simulink model "ODE_Hand_Model_v08_IPC_v03"  (Simulink 7.5)
settings: Solver=FixedStepDiscrete  StartTime=0.0  StopTime=inf  FixedStep=0.0315/(4*12)  RelTol=1e-3
values from neighbouring files (symbols this model uses):
  f_step = 0.7    [Set_Parameters.m]
  force_step = 20    [Set_Parameters.m]
  K_Conn = eye(4)*k_conn    [Set_Parameters.m]
  K_D = 30    [Set_Parameters.m]
  K_Or = eye(3)*k_Or    [Set_Parameters.m]
  K_Ot = eye(3)*k_Ot    [Set_Parameters.m]
  K_P = 350    [Set_Parameters.m]
  ksi = 0.9    [Set_Parameters.m]
  Kx = diag([diag(K_Ot)' diag(K_Or)' diag(K_Conn)'])    [Set_Parameters.m]
  l_des = [l1_des; l2_des; l3_des; l4_des]    [Set_Parameters.m]
  Mo = diag([sphere_mass*ones(1,3) (2/5)*sphere_mass*sphere_radius^2*ones(1,3)])    [Set_Parameters.m]
  qd_initial_touch = [0 0.3655   -0.5897   -0.5897     0       -0.3333   +0.5942   +0.5942         0       -0.298   --0.5226   --0.5226           0       -0.3333   +0.5942   +0.5942]    [Set_Parameters.m]
  R_O_Desired = R_O(x_i_v02(qd_initial_touch))    [Set_Parameters.m]
  t_f_start = 2.5    [Set_Parameters.m]
  torque_step = 60    [Set_Parameters.m]
  x_O_desired = (1/4)*sum(x_i_v02(qd_initial_touch))    [Set_Parameters.m]
undefined symbols (not defined in the file or in its folder): sigbuilder_block
libraries: dspmtrx3 x33, simulink x2, dspinverses x1
(part 2 of 6)

== matlab function Control/IPC/J/J_Or1/Embedded MATLAB Function1 ==
  data: xi input double size=[4 3]; J output double
%#eml
function J=J1(xi)

x1x=xi(1,1); x1y=xi(1,2); x1z=xi(1,3); 
x2x=xi(2,1); x2y=xi(2,2); x2z=xi(2,3);
x3x=xi(3,1); x3y=xi(3,2); x3z=xi(3,3);
x4x=xi(4,1); x4y=xi(4,2); x4z=xi(4,3);


J=[(x1x + (-1) .* x3x) .* (x1y + (-1) .* x3y) .* ((x1x + (-1) .*  ...
  x3x) .^ 2 + (x1y + (-1) .* x3y) .^ 2 + (x1z + (-1) .* x3z) .^ 2)  ...
  .^ (-3 / 2) .* (((-1) .* x1y + x3y) .* (x2x + (-1) .* x4x) + (x1x  ...
  + (-1) .* x3x) .* (x2y + (-1) .* x4y)) .* ((((-1) .* x1y + x3y) .* ...
   (x2x + (-1) .* x4x) + (x1x + (-1) .* x3x) .* (x2y + (-1) .* x4y)) ...
   .^ 2 + ((x1z + (-1) .* x3z) .* (x2x + (-1) .* x4x) + (-1) .* ( ...
  x1x + (-1) .* x3x) .* (x2z + (-1) .* x4z)) .^ 2 + (((-1) .* x1z +  ...
  x3z) .* (x2y + (-1) .* x4y) + (x1y + (-1) .* x3y) .* (x2z + (-1)  ...
  .* x4z)) .^ 2) .^ (-1 / 2) .* (((x1x + (-1) .* x3x) .* ((x1x + ( ...
  -1) .* x3x) .^ 2 + (x1y + (-1) .* x3y) .^ 2 + (x1z + (-1) .* x3z)  ...
  .^ 2) .^ (-1 / 2) + (x2x + (-1) .* x4x) .* ((x2x + (-1) .* x4x)  ...
  .^ 2 + (x2y + (-1) .* x4y) .^ 2 + (x2z + (-1) .* x4z) .^ 2) .^ ( ...
  -1 / 2)) .^ 2 + ((x1y + (-1) .* x3y) .* ((x1x + (-1) .* x3x) .^ 2  ...
  + (x1y + (-1) .* x3y) .^ 2 + (x1z + (-1) .* x3z) .^ 2) .^ (-1 / 2) ...
   + (x2y + (-1) .* x4y) .* ((x2x + (-1) .* x4x) .^ 2 + (x2y + (-1)  ...
  .* x4y) .^ 2 + (x2z + (-1) .* x4z) .^ 2) .^ (-1 / 2)) .^ 2 + ((( ...
  x1x + (-1) .* x3x) .^ 2 + (x1y + (-1) .* x3y) .^ 2 + (x1z + (-1)  ...
  .* x3z) .^ 2) .^ (-1 / 2) .* (x1z + (-1) .* x3z) + ((x2x + (-1) .* ...
   x4x) .^ 2 + (x2y + (-1) .* x4y) .^ 2 + (x2z + (-1) .* x4z) .^ 2)  ...
  .^ (-1 / 2) .* (x2z + (-1) .* x4z)) .^ 2) .^ (-1 / 2) + (1 / 2) .* ...
   (((-1) .* x1y + x3y) .* (x2x + (-1) .* x4x) + (x1x + (-1) .* x3x) ...
   .* (x2y + (-1) .* x4y)) .* ((((-1) .* x1y + x3y) .* (x2x + (-1)  ...
  .* x4x) + (x1x + (-1) .* x3x) .* (x2y + (-1) .* x4y)) .^ 2 + (( ...
  x1z + (-1) .* x3z) .* (x2x + (-1) .* x4x) + (-1) .* (x1x + (-1) .* ...
   x3x) .* (x2z + (-1) .* x4z)) .^ 2 + (((-1) .* x1z + x3z) .* (x2y  ...
  + (-1) .* x4y) + (x1y + (-1) .* x3y) .* (x2z + (-1) .* x4z)) .^ 2) ...
   .^ (-1 / 2) .* (2 .* ((-1) .* (x1x + (-1) .* x3x) .^ 2 .* ((x1x + ...
   (-1) .* x3x) .^ 2 + (x1y + (-1) .* x3y) .^ 2 + (x1z + (-1) .*  ...
  x3z) .^ 2) .^ (-3 / 2) + ((x1x + (-1) .* x3x) .^ 2 + (x1y + (-1)  ...
  .* x3y) .^ 2 + (x1z + (-1) .* x3z) .^ 2) .^ (-1 / 2)) .* ((x1x + ( ...
  -1) .* x3x) .* ((x1x + (-1) .* x3x) .^ 2 + (x1y + (-1) .* x3y) .^  ...
  2 + (x1z + (-1) .* x3z) .^ 2) .^ (-1 / 2) + (x2x + (-1) .* x4x) .* ...
   ((x2x + (-1) .* x4x) .^ 2 + (x2y + (-1) .* x4y) .^ 2 + (x2z + ( ...
  -1) .* x4z) .^ 2) .^ (-1 / 2)) + (-2) .* (x1x + (-1) .* x3x) .* ( ...
  x1y + (-1) .* x3y) .* ((x1x + (-1) .* x3x) .^ 2 + (x1y + (-1) .*  ...
  x3y) .^ 2 + (x1z + (-1) .* x3z) .^ 2) .^ (-3 / 2) .* ((x1y + (-1)  ...
  .* x3y) .* ((x1x + (-1) .* x3x) .^ 2 + (x1y + (-1) .* x3y) .^ 2 +  ...
  (x1z + (-1) .* x3z) .^ 2) .^ (-1 / 2) + (x2y + (-1) .* x4y) .* (( ...
  x2x + (-1) .* x4x) .^ 2 + (x2y + (-1) .* x4y) .^ 2 + (x2z + (-1)  ...
  .* x4z) .^ 2) .^ (-1 / 2)) + (-2) .* (x1x + (-1) .* x3x) .* ((x1x  ...
  + (-1) .* x3x) .^ 2 + (x1y + (-1) .* x3y) .^ 2 + (x1z + (-1) .*  ...
  x3z) .^ 2) .^ (-3 / 2) .* (x1z + (-1) .* x3z) .* (((x1x + (-1) .*  ...
  x3x) .^ 2 + (x1y + (-1) .* x3y) .^ 2 + (x1z + (-1) .* x3z) .^ 2)  ...
  .^ (-1 / 2) .* (x1z + (-1) .* x3z) + ((x2x + (-1) .* x4x) .^ 2 + ( ...
  x2y + (-1) .* x4y) .^ 2 + (x2z + (-1) .* x4z) .^ 2) .^ (-1 / 2) .* ...
   (x2z + (-1) .* x4z))) .* (((x1x + (-1) .* x3x) .* ((x1x + (-1) .* ...
   x3x) .^ 2 + (x1y + (-1) .* x3y) .^ 2 + (x1z + (-1) .* x3z) .^ 2)  ...
  .^ (-1 / 2) + (x2x + (-1) .* x4x) .* ((x2x + (-1) .* x4x) .^ 2 + ( ...
  x2y + (-1) .* x4y) .^ 2 + (x2z + (-1) .* x4z) .^ 2) .^ (-1 / 2))  ...
  .^ 2 + ((x1y + (-1) .* x3y) .* ((x1x + (-1) .* x3x) .^ 2 + (x1y +  ...
  (-1) .* x3y) .^ 2 + (x1z + (-1) .* x3z) .^ 2) .^ (-1 / 2) + (x2y + ...
   (-1) .* x4y) .* ((x2x + (-1) .* x4x) .^ 2 + (x2y + (-1) .* x4y)  ...
  .^ 2 + (x2z + (-1) .* x4z) .^ 2) .^ (-1 / 2)) .^ 2 + (((x1x + (-1) ...
   .* x3x) .^ 2 + (x1y + (-1) .* x3y) .^ 2 + (x1z + (-1) .* x3z) .^  ...
  2) .^ (-1 / 2) .* (x1z + (-1) .* x3z) + ((x2x + (-1) .* x4x) .^ 2  ...
  + (x2y + (-1) .* x4y) .^ 2 + (x2z + (-1) .* x4z) .^ 2) .^ (-1 / 2) ...
   .* (x2z + (-1) .* x4z)) .^ 2) .^ (-3 / 2) .* ((x1y + (-1) .* x3y) ...
   .* ((x1x + (-1) .* x3x) .^ 2 + (x1y + (-1) .* x3y) .^ 2 + (x1z +  ...
  (-1) .* x3z) .^ 2) .^ (-1 / 2) + (x2y + (-1) .* x4y) .* ((x2x + ( ...
  -1) .* x4x) .^ 2 + (x2y + (-1) .* x4y) .^ 2 + (x2z + (-1) .* x4z)  ...
  .^ 2) .^ (-1 / 2)) + (-1) .* (x2y + (-1) .* x4y) .* ((((-1) .*  ...
  x1y + x3y) .* (x2x + (-1) .* x4x) + (x1x + (-1) .* x3x) .* (x2y +  ...
  (-1) .* x4y)) .^ 2 + ((x1z + (-1) .* x3z) .* (x2x + (-1) .* x4x) + ...
   (-1) .* (x1x + (-1) .* x3x) .* (x2z + (-1) .* x4z)) .^ 2 + (((-1) ...
   .* x1z + x3z) .* (x2y + (-1) .* x4y) + (x1y + (-1) .* x3y) .* ( ...
  x2z + (-1) .* x4z)) .^ 2) .^ (-1 / 2) .* (((x1x + (-1) .* x3x) .*  ...
  ((x1x + (-1) .* x3x) .^ 2 + (x1y + (-1) .* x3y) .^ 2 + (x1z + (-1) ...
   .* x3z) .^ 2) .^ (-1 / 2) + (x2x + (-1) .* x4x) .* ((x2x + (-1)  ...
  .* x4x) .^ 2 + (x2y + (-1) .* x4y) .^ 2 + (x2z + (-1) .* x4z) .^  ...
  2) .^ (-1 / 2)) .^ 2 + ((x1y + (-1) .* x3y) .* ((x1x + (-1) .*  ...
  x3x) .^ 2 + (x1y + (-1) .* x3y) .^ 2 + (x1z + (-1) .* x3z) .^ 2)  ...
  .^ (-1 / 2) + (x2y + (-1) .* x4y) .* ((x2x + (-1) .* x4x) .^ 2 + ( ...
  x2y + (-1) .* x4y) .^ 2 + (x2z + (-1) .* x4z) .^ 2) .^ (-1 / 2))  ...
  .^ 2 + (((x1x + (-1) .* x3x) .^ 2 + (x1y + (-1) .* x3y) .^ 2 + ( ...
  x1z + (-1) .* x3z) .^ 2) .^ (-1 / 2) .* (x1z + (-1) .* x3z) + (( ...
  x2x + (-1) .* x4x) .^ 2 + (x2y + (-1) .* x4y) .^ 2 + (x2z + (-1)  ...
  .* x4z) .^ 2) .^ (-1 / 2) .* (x2z + (-1) .* x4z)) .^ 2) .^ (-1 /  ...
  2) .* ((x1y + (-1) .* x3y) .* ((x1x + (-1) .* x3x) .^ 2 + (x1y + ( ...
  -1) .* x3y) .^ 2 + (x1z + (-1) .* x3z) .^ 2) .^ (-1 / 2) + (x2y +  ...
  (-1) .* x4y) .* ((x2x + (-1) .* x4x) .^ 2 + (x2y + (-1) .* x4y)  ...
  .^ 2 + (x2z + (-1) .* x4z) .^ 2) .^ (-1 / 2)) + (-1) .* (x1x + ( ...
  -1) .* x3x) .* ((x1x + (-1) .* x3x) .^ 2 + (x1y + (-1) .* x3y) .^  ...
  2 + (x1z + (-1) .* x3z) .^ 2) .^ (-3 / 2) .* (x1z + (-1) .* x3z)  ...
  .* ((((-1) .* x1y + x3y) .* (x2x + (-1) .* x4x) + (x1x + (-1) .*  ...
  x3x) .* (x2y + (-1) .* x4y)) .^ 2 + ((x1z + (-1) .* x3z) .* (x2x + ...
   (-1) .* x4x) + (-1) .* (x1x + (-1) .* x3x) .* (x2z + (-1) .* x4z) ...
  ) .^ 2 + (((-1) .* x1z + x3z) .* (x2y + (-1) .* x4y) + (x1y + (-1) ...
   .* x3y) .* (x2z + (-1) .* x4z)) .^ 2) .^ (-1 / 2) .* (((x1x + ( ...
  -1) .* x3x) .* ((x1x + (-1) .* x3x) .^ 2 + (x1y + (-1) .* x3y) .^  ...
  2 + (x1z + (-1) .* x3z) .^ 2) .^ (-1 / 2) + (x2x + (-1) .* x4x) .* ...
   ((x2x + (-1) .* x4x) .^ 2 + (x2y + (-1) .* x4y) .^ 2 + (x2z + ( ...
  -1) .* x4z) .^ 2) .^ (-1 / 2)) .^ 2 + ((x1y + (-1) .* x3y) .* (( ...
  x1x + (-1) .* x3x) .^ 2 + (x1y + (-1) .* x3y) .^ 2 + (x1z + (-1)  ...
  .* x3z) .^ 2) .^ (-1 / 2) + (x2y + (-1) .* x4y) .* ((x2x + (-1) .* ...
   x4x) .^ 2 + (x2y + (-1) .* x4y) .^ 2 + (x2z + (-1) .* x4z) .^ 2)  ...
  .^ (-1 / 2)) .^ 2 + (((x1x + (-1) .* x3x) .^ 2 + (x1y + (-1) .*  ...
  x3y) .^ 2 + (x1z + (-1) .* x3z) .^ 2) .^ (-1 / 2) .* (x1z + (-1)  ...
  .* x3z) + ((x2x + (-1) .* x4x) .^ 2 + (x2y + (-1) .* x4y) .^ 2 + ( ...
  x2z + (-1) .* x4z) .^ 2) .^ (-1 / 2) .* (x2z + (-1) .* x4z)) .^ 2) ...
   .^ (-1 / 2) .* ((x1z + (-1) .* x3z) .* (x2x + (-1) .* x4x) + (-1) ...
   .* (x1x + (-1) .* x3x) .* (x2z + (-1) .* x4z)) + (-1 / 2) .* (((( ...
  -1) .* x1y + x3y) .* (x2x + (-1) .* x4x) + (x1x + (-1) .* x3x) .*  ...
  (x2y + (-1) .* x4y)) .^ 2 + ((x1z + (-1) .* x3z) .* (x2x + (-1) .* ...
   x4x) + (-1) .* (x1x + (-1) .* x3x) .* (x2z + (-1) .* x4z)) .^ 2 + ...
   (((-1) .* x1z + x3z) .* (x2y + (-1) .* x4y) + (x1y + (-1) .* x3y) ...
   .* (x2z + (-1) .* x4z)) .^ 2) .^ (-1 / 2) .* (2 .* ((-1) .* (x1x  ...
  + (-1) .* x3x) .^ 2 .* ((x1x + (-1) .* x3x) .^ 2 + (x1y + (-1) .*  ...
  x3y) .^ 2 + (x1z + (-1) .* x3z) .^ 2) .^ (-3 / 2) + ((x1x + (-1)  ...
  .* x3x) .^ 2 + (x1y + (-1) .* x3y) .^ 2 + (x1z + (-1) .* x3z) .^  ...
  2) .^ (-1 / 2)) .* ((x1x + (-1) .* x3x) .* ((x1x + (-1) .* x3x)  ...
  .^ 2 + (x1y + (-1) .* x3y) .^ 2 + (x1z + (-1) .* x3z) .^ 2) .^ ( ...
  -1 / 2) + (x2x + (-1) .* x4x) .* ((x2x + (-1) .* x4x) .^ 2 + (x2y  ...
  + (-1) .* x4y) .^ 2 + (x2z + (-1) .* x4z) .^ 2) .^ (-1 / 2)) + ( ...
  -2) .* (x1x + (-1) .* x3x) .* (x1y + (-1) .* x3y) .* ((x1x + (-1)  ...
  .* x3x) .^ 2 + (x1y + (-1) .* x3y) .^ 2 + (x1z + (-1) .* x3z) .^  ...
  2) .^ (-3 / 2) .* ((x1y + (-1) .* x3y) .* ((x1x + (-1) .* x3x) .^  ...
  2 + (x1y + (-1) .* x3y) .^ 2 + (x1z + (-1) .* x3z) .^ 2) .^ (-1 /  ...
  2) + (x2y + (-1) .* x4y) .* ((x2x + (-1) .* x4x) .^ 2 + (x2y + ( ...
  -1) .* x4y) .^ 2 + (x2z + (-1) .* x4z) .^ 2) .^ (-1 / 2)) + (-2)  ...
  .* (x1x + (-1) .* x3x) .* ((x1x + (-1) .* x3x) .^ 2 + (x1y + (-1)  ...
  .* x3y) .^ 2 + (x1z + (-1) .* x3z) .^ 2) .^ (-3 / 2) .* (x1z + ( ...
  -1) .* x3z) .* (((x1x + (-1) .* x3x) .^ 2 + (x1y + (-1) .* x3y)  ...
  .^ 2 + (x1z + (-1) .* x3z) .^ 2) .^ (-1 / 2) .* (x1z + (-1) .*  ...
  x3z) + ((x2x + (-1) .* x4x) .^ 2 + (x2y + (-1) .* x4y) .^ 2 + ( ...
  x2z + (-1) .* x4z) .^ 2) .^ (-1 / 2) .* (x2z + (-1) .* x4z))) .* ( ...
  ((x1x + (-1) .* x3x) .* ((x1x + (-1) .* x3x) .^ 2 + (x1y + (-1) .* ...
   x3y) .^ 2 + (x1z + (-1) .* x3z) .^ 2) .^ (-1 / 2) + (x2x + (-1)  ...
  .* x4x) .* ((x2x + (-1) .* x4x) .^ 2 + (x2y + (-1) .* x4y) .^ 2 +  ...
  (x2z + (-1) .* x4z) .^ 2) .^ (-1 / 2)) .^ 2 + ((x1y + (-1) .* x3y) ...
   .* ((x1x + (-1) .* x3x) .^ 2 + (x1y + (-1) .* x3y) .^ 2 + (x1z +  ...
  (-1) .* x3z) .^ 2) .^ (-1 / 2) + (x2y + (-1) .* x4y) .* ((x2x + ( ...
  -1) .* x4x) .^ 2 + (x2y + (-1) .* x4y) .^ 2 + (x2z + (-1) .* x4z)  ...
  .^ 2) .^ (-1 / 2)) .^ 2 + (((x1x + (-1) .* x3x) .^ 2 + (x1y + (-1) ...
   .* x3y) .^ 2 + (x1z + (-1) .* x3z) .^ 2) .^ (-1 / 2) .* (x1z + ( ...
  -1) .* x3z) + ((x2x + (-1) .* x4x) .^ 2 + (x2y + (-1) .* x4y) .^  ...
  2 + (x2z + (-1) .* x4z) .^ 2) .^ (-1 / 2) .* (x2z + (-1) .* x4z))  ...
  .^ 2) .^ (-3 / 2) .* ((x1z + (-1) .* x3z) .* (x2x + (-1) .* x4x) + ...
   (-1) .* (x1x + (-1) .* x3x) .* (x2z + (-1) .* x4z)) .* (((x1x + ( ...
  -1) .* x3x) .^ 2 + (x1y + (-1) .* x3y) .^ 2 + (x1z + (-1) .* x3z)  ...
  .^ 2) .^ (-1 / 2) .* (x1z + (-1) .* x3z) + ((x2x + (-1) .* x4x)  ...
  .^ 2 + (x2y + (-1) .* x4y) .^ 2 + (x2z + (-1) .* x4z) .^ 2) .^ ( ...
  -1 / 2) .* (x2z + (-1) .* x4z)) + ((((-1) .* x1y + x3y) .* (x2x +  ...
  (-1) .* x4x) + (x1x + (-1) .* x3x) .* (x2y + (-1) .* x4y)) .^ 2 +  ...
  ((x1z + (-1) .* x3z) .* (x2x + (-1) .* x4x) + (-1) .* (x1x + (-1)  ...
  .* x3x) .* (x2z + (-1) .* x4z)) .^ 2 + (((-1) .* x1z + x3z) .* ( ...
  x2y + (-1) .* x4y) + (x1y + (-1) .* x3y) .* (x2z + (-1) .* x4z))  ...
  .^ 2) .^ (-1 / 2) .* (((x1x + (-1) .* x3x) .* ((x1x + (-1) .* x3x) ...
   .^ 2 + (x1y + (-1) .* x3y) .^ 2 + (x1z + (-1) .* x3z) .^ 2) .^ ( ...
  -1 / 2) + (x2x + (-1) .* x4x) .* ((x2x + (-1) .* x4x) .^ 2 + (x2y  ...
  + (-1) .* x4y) .^ 2 + (x2z + (-1) .* x4z) .^ 2) .^ (-1 / 2)) .^ 2  ...
  + ((x1y + (-1) .* x3y) .* ((x1x + (-1) .* x3x) .^ 2 + (x1y + (-1)  ...
  .* x3y) .^ 2 + (x1z + (-1) .* x3z) .^ 2) .^ (-1 / 2) + (x2y + (-1) ...
   .* x4y) .* ((x2x + (-1) .* x4x) .^ 2 + (x2y + (-1) .* x4y) .^ 2 + ...
   (x2z + (-1) .* x4z) .^ 2) .^ (-1 / 2)) .^ 2 + (((x1x + (-1) .*  ...
  x3x) .^ 2 + (x1y + (-1) .* x3y) .^ 2 + (x1z + (-1) .* x3z) .^ 2)  ...
  .^ (-1 / 2) .* (x1z + (-1) .* x3z) + ((x2x + (-1) .* x4x) .^ 2 + ( ...
  x2y + (-1) .* x4y) .^ 2 + (x2z + (-1) .* x4z) .^ 2) .^ (-1 / 2) .* ...
   (x2z + (-1) .* x4z)) .^ 2) .^ (-1 / 2) .* (((x1x + (-1) .* x3x)  ...
  .^ 2 + (x1y + (-1) .* x3y) .^ 2 + (x1z + (-1) .* x3z) .^ 2) .^ ( ...
  -1 / 2) .* (x1z + (-1) .* x3z) + ((x2x + (-1) .* x4x) .^ 2 + (x2y  ...
  + (-1) .* x4y) .^ 2 + (x2z + (-1) .* x4z) .^ 2) .^ (-1 / 2) .* ( ...
  x2z + (-1) .* x4z)) .* ((-1) .* x2z + x4z) + (1 / 2) .* (((-1) .*  ...
  x1y + x3y) .* (x2x + (-1) .* x4x) + (x1x + (-1) .* x3x) .* (x2y +  ...
  (-1) .* x4y)) .* ((((-1) .* x1y + x3y) .* (x2x + (-1) .* x4x) + ( ...
  x1x + (-1) .* x3x) .* (x2y + (-1) .* x4y)) .^ 2 + ((x1z + (-1) .*  ...
  x3z) .* (x2x + (-1) .* x4x) + (-1) .* (x1x + (-1) .* x3x) .* (x2z  ...
  + (-1) .* x4z)) .^ 2 + (((-1) .* x1z + x3z) .* (x2y + (-1) .* x4y) ...
   + (x1y + (-1) .* x3y) .* (x2z + (-1) .* x4z)) .^ 2) .^ (-3 / 2)  ...
  .* (((x1x + (-1) .* x3x) .* ((x1x + (-1) .* x3x) .^ 2 + (x1y + ( ...
  -1) .* x3y) .^ 2 + (x1z + (-1) .* x3z) .^ 2) .^ (-1 / 2) + (x2x +  ...
  (-1) .* x4x) .* ((x2x + (-1) .* x4x) .^ 2 + (x2y + (-1) .* x4y)  ...
  .^ 2 + (x2z + (-1) .* x4z) .^ 2) .^ (-1 / 2)) .^ 2 + ((x1y + (-1)  ...
  .* x3y) .* ((x1x + (-1) .* x3x) .^ 2 + (x1y + (-1) .* x3y) .^ 2 +  ...
  (x1z + (-1) .* x3z) .^ 2) .^ (-1 / 2) + (x2y + (-1) .* x4y) .* (( ...
  x2x + (-1) .* x4x) .^ 2 + (x2y + (-1) .* x4y) .^ 2 + (x2z + (-1)  ...
  .* x4z) .^ 2) .^ (-1 / 2)) .^ 2 + (((x1x + (-1) .* x3x) .^ 2 + ( ...
  x1y + (-1) .* x3y) .^ 2 + (x1z + (-1) .* x3z) .^ 2) .^ (-1 / 2) .* ...
   (x1z + (-1) .* x3z) + ((x2x + (-1) .* x4x) .^ 2 + (x2y + (-1) .*  ...
  x4y) .^ 2 + (x2z + (-1) .* x4z) .^ 2) .^ (-1 / 2) .* (x2z + (-1)  ...
  .* x4z)) .^ 2) .^ (-1 / 2) .* ((x1y + (-1) .* x3y) .* ((x1x + (-1) ...
   .* x3x) .^ 2 + (x1y + (-1) .* x3y) .^ 2 + (x1z + (-1) .* x3z) .^  ...
  2) .^ (-1 / 2) + (x2y + (-1) .* x4y) .* ((x2x + (-1) .* x4x) .^ 2  ...
  + (x2y + (-1) .* x4y) .^ 2 + (x2z + (-1) .* x4z) .^ 2) .^ (-1 / 2) ...
  ) .* (2 .* (((-1) .* x1y + x3y) .* (x2x + (-1) .* x4x) + (x1x + ( ...
  -1) .* x3x) .* (x2y + (-1) .* x4y)) .* (x2y + (-1) .* x4y) + 2 .*  ...
  ((x1z + (-1) .* x3z) .* (x2x + (-1) .* x4x) + (-1) .* (x1x + (-1)  ...
  .* x3x) .* (x2z + (-1) .* x4z)) .* ((-1) .* x2z + x4z)) + (-1 / 2) ...
   .* ((((-1) .* x1y + x3y) .* (x2x + (-1) .* x4x) + (x1x + (-1) .*  ...
  x3x) .* (x2y + (-1) .* x4y)) .^ 2 + ((x1z + (-1) .* x3z) .* (x2x + ...
   (-1) .* x4x) + (-1) .* (x1x + (-1) .* x3x) .* (x2z + (-1) .* x4z) ...
  ) .^ 2 + (((-1) .* x1z + x3z) .* (x2y + (-1) .* x4y) + (x1y + (-1) ...
   .* x3y) .* (x2z + (-1) .* x4z)) .^ 2) .^ (-3 / 2) .* (((x1x + ( ...
  -1) .* x3x) .* ((x1x + (-1) .* x3x) .^ 2 + (x1y + (-1) .* x3y) .^  ...
  2 + (x1z + (-1) .* x3z) .^ 2) .^ (-1 / 2) + (x2x + (-1) .* x4x) .* ...
   ((x2x + (-1) .* x4x) .^ 2 + (x2y + (-1) .* x4y) .^ 2 + (x2z + ( ...
  -1) .* x4z) .^ 2) .^ (-1 / 2)) .^ 2 + ((x1y + (-1) .* x3y) .* (( ...
  x1x + (-1) .* x3x) .^ 2 + (x1y + (-1) .* x3y) .^ 2 + (x1z + (-1)  ...
  .* x3z) .^ 2) .^ (-1 / 2) + (x2y + (-1) .* x4y) .* ((x2x + (-1) .* ...
   x4x) .^ 2 + (x2y + (-1) .* x4y) .^ 2 + (x2z + (-1) .* x4z) .^ 2)  ...
  .^ (-1 / 2)) .^ 2 + (((x1x + (-1) .* x3x) .^ 2 + (x1y + (-1) .*  ...
  x3y) .^ 2 + (x1z + (-1) .* x3z) .^ 2) .^ (-1 / 2) .* (x1z + (-1)  ...
  .* x3z) + ((x2x + (-1) .* x4x) .^ 2 + (x2y + (-1) .* x4y) .^ 2 + ( ...
  x2z + (-1) .* x4z) .^ 2) .^ (-1 / 2) .* (x2z + (-1) .* x4z)) .^ 2) ...
   .^ (-1 / 2) .* ((x1z + (-1) .* x3z) .* (x2x + (-1) .* x4x) + (-1) ...
   .* (x1x + (-1) .* x3x) .* (x2z + (-1) .* x4z)) .* (((x1x + (-1)  ...
  .* x3x) .^ 2 + (x1y + (-1) .* x3y) .^ 2 + (x1z + (-1) .* x3z) .^  ...
  2) .^ (-1 / 2) .* (x1z + (-1) .* x3z) + ((x2x + (-1) .* x4x) .^ 2  ...
  + (x2y + (-1) .* x4y) .^ 2 + (x2z + (-1) .* x4z) .^ 2) .^ (-1 / 2) ...
   .* (x2z + (-1) .* x4z)) .* (2 .* (((-1) .* x1y + x3y) .* (x2x + ( ...
  -1) .* x4x) + (x1x + (-1) .* x3x) .* (x2y + (-1) .* x4y)) .* (x2y  ...
  + (-1) .* x4y) + 2 .* ((x1z + (-1) .* x3z) .* (x2x + (-1) .* x4x)  ...
  + (-1) .* (x1x + (-1) .* x3x) .* (x2z + (-1) .* x4z)) .* ((-1) .*  ...
  x2z + x4z)),(-1) .* ((-1) .* (x1y + (-1) .* x3y) .^ 2 .* ((x1x + ( ...
  -1) .* x3x) .^ 2 + (x1y + (-1) .* x3y) .^ 2 + (x1z + (-1) .* x3z)  ...
  .^ 2) .^ (-3 / 2) + ((x1x + (-1) .* x3x) .^ 2 + (x1y + (-1) .*  ...
  x3y) .^ 2 + (x1z + (-1) .* x3z) .^ 2) .^ (-1 / 2)) .* (((-1) .*  ...
  x1y + x3y) .* (x2x + (-1) .* x4x) + (x1x + (-1) .* x3x) .* (x2y +  ...
  (-1) .* x4y)) .* ((((-1) .* x1y + x3y) .* (x2x + (-1) .* x4x) + ( ...
  x1x + (-1) .* x3x) .* (x2y + (-1) .* x4y)) .^ 2 + ((x1z + (-1) .*  ...
  x3z) .* (x2x + (-1) .* x4x) + (-1) .* (x1x + (-1) .* x3x) .* (x2z  ...
  + (-1) .* x4z)) .^ 2 + (((-1) .* x1z + x3z) .* (x2y + (-1) .* x4y) ...
   + (x1y + (-1) .* x3y) .* (x2z + (-1) .* x4z)) .^ 2) .^ (-1 / 2)  ...
  .* (((x1x + (-1) .* x3x) .* ((x1x + (-1) .* x3x) .^ 2 + (x1y + ( ...
  -1) .* x3y) .^ 2 + (x1z + (-1) .* x3z) .^ 2) .^ (-1 / 2) + (x2x +  ...
  (-1) .* x4x) .* ((x2x + (-1) .* x4x) .^ 2 + (x2y + (-1) .* x4y)  ...
  .^ 2 + (x2z + (-1) .* x4z) .^ 2) .^ (-1 / 2)) .^ 2 + ((x1y + (-1)  ...
  .* x3y) .* ((x1x + (-1) .* x3x) .^ 2 + (x1y + (-1) .* x3y) .^ 2 +  ...
  (x1z + (-1) .* x3z) .^ 2) .^ (-1 / 2) + (x2y + (-1) .* x4y) .* (( ...
  x2x + (-1) .* x4x) .^ 2 + (x2y + (-1) .* x4y) .^ 2 + (x2z + (-1)  ...
  .* x4z) .^ 2) .^ (-1 / 2)) .^ 2 + (((x1x + (-1) .* x3x) .^ 2 + ( ...
  x1y + (-1) .* x3y) .^ 2 + (x1z + (-1) .* x3z) .^ 2) .^ (-1 / 2) .* ...
   (x1z + (-1) .* x3z) + ((x2x + (-1) .* x4x) .^ 2 + (x2y + (-1) .*  ...
  x4y) .^ 2 + (x2z + (-1) .* x4z) .^ 2) .^ (-1 / 2) .* (x2z + (-1)  ...
  .* x4z)) .^ 2) .^ (-1 / 2) + (1 / 2) .* (((-1) .* x1y + x3y) .* ( ...
  x2x + (-1) .* x4x) + (x1x + (-1) .* x3x) .* (x2y + (-1) .* x4y))  ...
  .* ((((-1) .* x1y + x3y) .* (x2x + (-1) .* x4x) + (x1x + (-1) .*  ...
  x3x) .* (x2y + (-1) .* x4y)) .^ 2 + ((x1z + (-1) .* x3z) .* (x2x + ...
   (-1) .* x4x) + (-1) .* (x1x + (-1) .* x3x) .* (x2z + (-1) .* x4z) ...
  ) .^ 2 + (((-1) .* x1z + x3z) .* (x2y + (-1) .* x4y) + (x1y + (-1) ...
   .* x3y) .* (x2z + (-1) .* x4z)) .^ 2) .^ (-1 / 2) .* ((-2) .* ( ...
  x1x + (-1) .* x3x) .* (x1y + (-1) .* x3y) .* ((x1x + (-1) .* x3x)  ...
  .^ 2 + (x1y + (-1) .* x3y) .^ 2 + (x1z + (-1) .* x3z) .^ 2) .^ ( ...
  -3 / 2) .* ((x1x + (-1) .* x3x) .* ((x1x + (-1) .* x3x) .^ 2 + ( ...
  x1y + (-1) .* x3y) .^ 2 + (x1z + (-1) .* x3z) .^ 2) .^ (-1 / 2) +  ...
  (x2x + (-1) .* x4x) .* ((x2x + (-1) .* x4x) .^ 2 + (x2y + (-1) .*  ...
  x4y) .^ 2 + (x2z + (-1) .* x4z) .^ 2) .^ (-1 / 2)) + 2 .* ((-1) .* ...
   (x1y + (-1) .* x3y) .^ 2 .* ((x1x + (-1) .* x3x) .^ 2 + (x1y + ( ...
  -1) .* x3y) .^ 2 + (x1z + (-1) .* x3z) .^ 2) .^ (-3 / 2) + ((x1x + ...
   (-1) .* x3x) .^ 2 + (x1y + (-1) .* x3y) .^ 2 + (x1z + (-1) .*  ...
  x3z) .^ 2) .^ (-1 / 2)) .* ((x1y + (-1) .* x3y) .* ((x1x + (-1) .* ...
   x3x) .^ 2 + (x1y + (-1) .* x3y) .^ 2 + (x1z + (-1) .* x3z) .^ 2)  ...
  .^ (-1 / 2) + (x2y + (-1) .* x4y) .* ((x2x + (-1) .* x4x) .^ 2 + ( ...
  x2y + (-1) .* x4y) .^ 2 + (x2z + (-1) .* x4z) .^ 2) .^ (-1 / 2)) + ...
   (-2) .* (x1y + (-1) .* x3y) .* ((x1x + (-1) .* x3x) .^ 2 + (x1y + ...
   (-1) .* x3y) .^ 2 + (x1z + (-1) .* x3z) .^ 2) .^ (-3 / 2) .* ( ...
  x1z + (-1) .* x3z) .* (((x1x + (-1) .* x3x) .^ 2 + (x1y + (-1) .*  ...
  x3y) .^ 2 + (x1z + (-1) .* x3z) .^ 2) .^ (-1 / 2) .* (x1z + (-1)  ...
  .* x3z) + ((x2x + (-1) .* x4x) .^ 2 + (x2y + (-1) .* x4y) .^ 2 + ( ...
  x2z + (-1) .* x4z) .^ 2) .^ (-1 / 2) .* (x2z + (-1) .* x4z))) .* ( ...
  ((x1x + (-1) .* x3x) .* ((x1x + (-1) .* x3x) .^ 2 + (x1y + (-1) .* ...
   x3y) .^ 2 + (x1z + (-1) .* x3z) .^ 2) .^ (-1 / 2) + (x2x + (-1)  ...
  .* x4x) .* ((x2x + (-1) .* x4x) .^ 2 + (x2y + (-1) .* x4y) .^ 2 +  ...
  (x2z + (-1) .* x4z) .^ 2) .^ (-1 / 2)) .^ 2 + ((x1y + (-1) .* x3y) ...
   .* ((x1x + (-1) .* x3x) .^ 2 + (x1y + (-1) .* x3y) .^ 2 + (x1z +  ...
  (-1) .* x3z) .^ 2) .^ (-1 / 2) + (x2y + (-1) .* x4y) .* ((x2x + ( ...
  -1) .* x4x) .^ 2 + (x2y + (-1) .* x4y) .^ 2 + (x2z + (-1) .* x4z)  ...
  .^ 2) .^ (-1 / 2)) .^ 2 + (((x1x + (-1) .* x3x) .^ 2 + (x1y + (-1) ...
   .* x3y) .^ 2 + (x1z + (-1) .* x3z) .^ 2) .^ (-1 / 2) .* (x1z + ( ...
  -1) .* x3z) + ((x2x + (-1) .* x4x) .^ 2 + (x2y + (-1) .* x4y) .^  ...
  2 + (x2z + (-1) .* x4z) .^ 2) .^ (-1 / 2) .* (x2z + (-1) .* x4z))  ...
  .^ 2) .^ (-3 / 2) .* ((x1y + (-1) .* x3y) .* ((x1x + (-1) .* x3x)  ...
  .^ 2 + (x1y + (-1) .* x3y) .^ 2 + (x1z + (-1) .* x3z) .^ 2) .^ ( ...
  -1 / 2) + (x2y + (-1) .* x4y) .* ((x2x + (-1) .* x4x) .^ 2 + (x2y  ...
  + (-1) .* x4y) .^ 2 + (x2z + (-1) .* x4z) .^ 2) .^ (-1 / 2)) + ( ...
  -1) .* ((-1) .* x2x + x4x) .* ((((-1) .* x1y + x3y) .* (x2x + (-1) ...
   .* x4x) + (x1x + (-1) .* x3x) .* (x2y + (-1) .* x4y)) .^ 2 + (( ...
  x1z + (-1) .* x3z) .* (x2x + (-1) .* x4x) + (-1) .* (x1x + (-1) .* ...
   x3x) .* (x2z + (-1) .* x4z)) .^ 2 + (((-1) .* x1z + x3z) .* (x2y  ...
  + (-1) .* x4y) + (x1y + (-1) .* x3y) .* (x2z + (-1) .* x4z)) .^ 2) ...
   .^ (-1 / 2) .* (((x1x + (-1) .* x3x) .* ((x1x + (-1) .* x3x) .^  ...
  2 + (x1y + (-1) .* x3y) .^ 2 + (x1z + (-1) .* x3z) .^ 2) .^ (-1 /  ...
  2) + (x2x + (-1) .* x4x) .* ((x2x + (-1) .* x4x) .^ 2 + (x2y + ( ...
  -1) .* x4y) .^ 2 + (x2z + (-1) .* x4z) .^ 2) .^ (-1 / 2)) .^ 2 + ( ...
  (x1y + (-1) .* x3y) .* ((x1x + (-1) .* x3x) .^ 2 + (x1y + (-1) .*  ...
  x3y) .^ 2 + (x1z + (-1) .* x3z) .^ 2) .^ (-1 / 2) + (x2y + (-1) .* ...
   x4y) .* ((x2x + (-1) .* x4x) .^ 2 + (x2y + (-1) .* x4y) .^ 2 + ( ...
  x2z + (-1) .* x4z) .^ 2) .^ (-1 / 2)) .^ 2 + (((x1x + (-1) .* x3x) ...
   .^ 2 + (x1y + (-1) .* x3y) .^ 2 + (x1z + (-1) .* x3z) .^ 2) .^ ( ...
  -1 / 2) .* (x1z + (-1) .* x3z) + ((x2x + (-1) .* x4x) .^ 2 + (x2y  ...
  + (-1) .* x4y) .^ 2 + (x2z + (-1) .* x4z) .^ 2) .^ (-1 / 2) .* ( ...
  x2z + (-1) .* x4z)) .^ 2) .^ (-1 / 2) .* ((x1y + (-1) .* x3y) .* ( ...
  (x1x + (-1) .* x3x) .^ 2 + (x1y + (-1) .* x3y) .^ 2 + (x1z + (-1)  ...
  .* x3z) .^ 2) .^ (-1 / 2) + (x2y + (-1) .* x4y) .* ((x2x + (-1) .* ...
   x4x) .^ 2 + (x2y + (-1) .* x4y) .^ 2 + (x2z + (-1) .* x4z) .^ 2)  ...
  .^ (-1 / 2)) + (-1) .* (x1y + (-1) .* x3y) .* ((x1x + (-1) .* x3x) ...
   .^ 2 + (x1y + (-1) .* x3y) .^ 2 + (x1z + (-1) .* x3z) .^ 2) .^ ( ...
  -3 / 2) .* (x1z + (-1) .* x3z) .* ((((-1) .* x1y + x3y) .* (x2x +  ...
  (-1) .* x4x) + (x1x + (-1) .* x3x) .* (x2y + (-1) .* x4y)) .^ 2 +  ...
  ((x1z + (-1) .* x3z) .* (x2x + (-1) .* x4x) + (-1) .* (x1x + (-1)  ...
  .* x3x) .* (x2z + (-1) .* x4z)) .^ 2 + (((-1) .* x1z + x3z) .* ( ...
  x2y + (-1) .* x4y) + (x1y + (-1) .* x3y) .* (x2z + (-1) .* x4z))  ...
  .^ 2) .^ (-1 / 2) .* (((x1x + (-1) .* x3x) .* ((x1x + (-1) .* x3x) ...
   .^ 2 + (x1y + (-1) .* x3y) .^ 2 + (x1z + (-1) .* x3z) .^ 2) .^ ( ...
  -1 / 2) + (x2x + (-1) .* x4x) .* ((x2x + (-1) .* x4x) .^ 2 + (x2y  ...
  + (-1) .* x4y) .^ 2 + (x2z + (-1) .* x4z) .^ 2) .^ (-1 / 2)) .^ 2  ...
  + ((x1y + (-1) .* x3y) .* ((x1x + (-1) .* x3x) .^ 2 + (x1y + (-1)  ...
  .* x3y) .^ 2 + (x1z + (-1) .* x3z) .^ 2) .^ (-1 / 2) + (x2y + (-1) ...
   .* x4y) .* ((x2x + (-1) .* x4x) .^ 2 + (x2y + (-1) .* x4y) .^ 2 + ...
   (x2z + (-1) .* x4z) .^ 2) .^ (-1 / 2)) .^ 2 + (((x1x + (-1) .*  ...
  x3x) .^ 2 + (x1y + (-1) .* x3y) .^ 2 + (x1z + (-1) .* x3z) .^ 2)  ...
  .^ (-1 / 2) .* (x1z + (-1) .* x3z) + ((x2x + (-1) .* x4x) .^ 2 + ( ...
  x2y + (-1) .* x4y) .^ 2 + (x2z + (-1) .* x4z) .^ 2) .^ (-1 / 2) .* ...
   (x2z + (-1) .* x4z)) .^ 2) .^ (-1 / 2) .* ((x1z + (-1) .* x3z) .* ...
   (x2x + (-1) .* x4x) + (-1) .* (x1x + (-1) .* x3x) .* (x2z + (-1)  ...
  .* x4z)) + (1 / 2) .* (((-1) .* x1y + x3y) .* (x2x + (-1) .* x4x)  ...
  + (x1x + (-1) .* x3x) .* (x2y + (-1) .* x4y)) .* ((((-1) .* x1y +  ...
  x3y) .* (x2x + (-1) .* x4x) + (x1x + (-1) .* x3x) .* (x2y + (-1)  ...
  .* x4y)) .^ 2 + ((x1z + (-1) .* x3z) .* (x2x + (-1) .* x4x) + (-1) ...
   .* (x1x + (-1) .* x3x) .* (x2z + (-1) .* x4z)) .^ 2 + (((-1) .*  ...
  x1z + x3z) .* (x2y + (-1) .* x4y) + (x1y + (-1) .* x3y) .* (x2z +  ...
  (-1) .* x4z)) .^ 2) .^ (-3 / 2) .* (((x1x + (-1) .* x3x) .* ((x1x  ...
  + (-1) .* x3x) .^ 2 + (x1y + (-1) .* x3y) .^ 2 + (x1z + (-1) .*  ...
  x3z) .^ 2) .^ (-1 / 2) + (x2x + (-1) .* x4x) .* ((x2x + (-1) .*  ...
  x4x) .^ 2 + (x2y + (-1) .* x4y) .^ 2 + (x2z + (-1) .* x4z) .^ 2)  ...
  .^ (-1 / 2)) .^ 2 + ((x1y + (-1) .* x3y) .* ((x1x + (-1) .* x3x)  ...
  .^ 2 + (x1y + (-1) .* x3y) .^ 2 + (x1z + (-1) .* x3z) .^ 2) .^ ( ...
  -1 / 2) + (x2y + (-1) .* x4y) .* ((x2x + (-1) .* x4x) .^ 2 + (x2y  ...
  + (-1) .* x4y) .^ 2 + (x2z + (-1) .* x4z) .^ 2) .^ (-1 / 2)) .^ 2  ...
  + (((x1x + (-1) .* x3x) .^ 2 + (x1y + (-1) .* x3y) .^ 2 + (x1z + ( ...
  -1) .* x3z) .^ 2) .^ (-1 / 2) .* (x1z + (-1) .* x3z) + ((x2x + ( ...
  -1) .* x4x) .^ 2 + (x2y + (-1) .* x4y) .^ 2 + (x2z + (-1) .* x4z)  ...
  .^ 2) .^ (-1 / 2) .* (x2z + (-1) .* x4z)) .^ 2) .^ (-1 / 2) .* (( ...
  x1y + (-1) .* x3y) .* ((x1x + (-1) .* x3x) .^ 2 + (x1y + (-1) .*  ...
  x3y) .^ 2 + (x1z + (-1) .* x3z) .^ 2) .^ (-1 / 2) + (x2y + (-1) .* ...
   x4y) .* ((x2x + (-1) .* x4x) .^ 2 + (x2y + (-1) .* x4y) .^ 2 + ( ...
  x2z + (-1) .* x4z) .^ 2) .^ (-1 / 2)) .* (2 .* ((-1) .* x2x + x4x) ...
   .* (((-1) .* x1y + x3y) .* (x2x + (-1) .* x4x) + (x1x + (-1) .*  ...
  x3x) .* (x2y + (-1) .* x4y)) + 2 .* (((-1) .* x1z + x3z) .* (x2y + ...
   (-1) .* x4y) + (x1y + (-1) .* x3y) .* (x2z + (-1) .* x4z)) .* ( ...
  x2z + (-1) .* x4z)) + (-1 / 2) .* ((((-1) .* x1y + x3y) .* (x2x +  ...
  (-1) .* x4x) + (x1x + (-1) .* x3x) .* (x2y + (-1) .* x4y)) .^ 2 +  ...
  ((x1z + (-1) .* x3z) .* (x2x + (-1) .* x4x) + (-1) .* (x1x + (-1)  ...
  .* x3x) .* (x2z + (-1) .* x4z)) .^ 2 + (((-1) .* x1z + x3z) .* ( ...
  x2y + (-1) .* x4y) + (x1y + (-1) .* x3y) .* (x2z + (-1) .* x4z))  ...
  .^ 2) .^ (-1 / 2) .* ((-2) .* (x1x + (-1) .* x3x) .* (x1y + (-1)  ...
  .* x3y) .* ((x1x + (-1) .* x3x) .^ 2 + (x1y + (-1) .* x3y) .^ 2 +  ...
  (x1z + (-1) .* x3z) .^ 2) .^ (-3 / 2) .* ((x1x + (-1) .* x3x) .* ( ...
  (x1x + (-1) .* x3x) .^ 2 + (x1y + (-1) .* x3y) .^ 2 + (x1z + (-1)  ...
  .* x3z) .^ 2) .^ (-1 / 2) + (x2x + (-1) .* x4x) .* ((x2x + (-1) .* ...
   x4x) .^ 2 + (x2y + (-1) .* x4y) .^ 2 + (x2z + (-1) .* x4z) .^ 2)  ...
  .^ (-1 / 2)) + 2 .* ((-1) .* (x1y + (-1) .* x3y) .^ 2 .* ((x1x + ( ...
  -1) .* x3x) .^ 2 + (x1y + (-1) .* x3y) .^ 2 + (x1z + (-1) .* x3z)  ...
  .^ 2) .^ (-3 / 2) + ((x1x + (-1) .* x3x) .^ 2 + (x1y + (-1) .*  ...
  x3y) .^ 2 + (x1z + (-1) .* x3z) .^ 2) .^ (-1 / 2)) .* ((x1y + (-1) ...
   .* x3y) .* ((x1x + (-1) .* x3x) .^ 2 + (x1y + (-1) .* x3y) .^ 2 + ...
   (x1z + (-1) .* x3z) .^ 2) .^ (-1 / 2) + (x2y + (-1) .* x4y) .* (( ...
  x2x + (-1) .* x4x) .^ 2 + (x2y + (-1) .* x4y) .^ 2 + (x2z + (-1)  ...
  .* x4z) .^ 2) .^ (-1 / 2)) + (-2) .* (x1y + (-1) .* x3y) .* ((x1x  ...
  + (-1) .* x3x) .^ 2 + (x1y + (-1) .* x3y) .^ 2 + (x1z + (-1) .*  ...
  x3z) .^ 2) .^ (-3 / 2) .* (x1z + (-1) .* x3z) .* (((x1x + (-1) .*  ...
  x3x) .^ 2 + (x1y + (-1) .* x3y) .^ 2 + (x1z + (-1) .* x3z) .^ 2)  ...
  .^ (-1 / 2) .* (x1z + (-1) .* x3z) + ((x2x + (-1) .* x4x) .^ 2 + ( ...
  x2y + (-1) .* x4y) .^ 2 + (x2z + (-1) .* x4z) .^ 2) .^ (-1 / 2) .* ...
   (x2z + (-1) .* x4z))) .* (((x1x + (-1) .* x3x) .* ((x1x + (-1) .* ...
   x3x) .^ 2 + (x1y + (-1) .* x3y) .^ 2 + (x1z + (-1) .* x3z) .^ 2)  ...
  .^ (-1 / 2) + (x2x + (-1) .* x4x) .* ((x2x + (-1) .* x4x) .^ 2 + ( ...
  x2y + (-1) .* x4y) .^ 2 + (x2z + (-1) .* x4z) .^ 2) .^ (-1 / 2))  ...
  .^ 2 + ((x1y + (-1) .* x3y) .* ((x1x + (-1) .* x3x) .^ 2 + (x1y +  ...
  (-1) .* x3y) .^ 2 + (x1z + (-1) .* x3z) .^ 2) .^ (-1 / 2) + (x2y + ...
   (-1) .* x4y) .* ((x2x + (-1) .* x4x) .^ 2 + (x2y + (-1) .* x4y)  ...
  .^ 2 + (x2z + (-1) .* x4z) .^ 2) .^ (-1 / 2)) .^ 2 + (((x1x + (-1) ...
   .* x3x) .^ 2 + (x1y + (-1) .* x3y) .^ 2 + (x1z + (-1) .* x3z) .^  ...
  2) .^ (-1 / 2) .* (x1z + (-1) .* x3z) + ((x2x + (-1) .* x4x) .^ 2  ...
  + (x2y + (-1) .* x4y) .^ 2 + (x2z + (-1) .* x4z) .^ 2) .^ (-1 / 2) ...
   .* (x2z + (-1) .* x4z)) .^ 2) .^ (-3 / 2) .* ((x1z + (-1) .* x3z) ...
   .* (x2x + (-1) .* x4x) + (-1) .* (x1x + (-1) .* x3x) .* (x2z + ( ...
  -1) .* x4z)) .* (((x1x + (-1) .* x3x) .^ 2 + (x1y + (-1) .* x3y)  ...
  .^ 2 + (x1z + (-1) .* x3z) .^ 2) .^ (-1 / 2) .* (x1z + (-1) .*  ...
  x3z) + ((x2x + (-1) .* x4x) .^ 2 + (x2y + (-1) .* x4y) .^ 2 + ( ...
  x2z + (-1) .* x4z) .^ 2) .^ (-1 / 2) .* (x2z + (-1) .* x4z)) + ( ...
  -1 / 2) .* ((((-1) .* x1y + x3y) .* (x2x + (-1) .* x4x) + (x1x + ( ...
  -1) .* x3x) .* (x2y + (-1) .* x4y)) .^ 2 + ((x1z + (-1) .* x3z) .* ...
   (x2x + (-1) .* x4x) + (-1) .* (x1x + (-1) .* x3x) .* (x2z + (-1)  ...
  .* x4z)) .^ 2 + (((-1) .* x1z + x3z) .* (x2y + (-1) .* x4y) + ( ...
  x1y + (-1) .* x3y) .* (x2z + (-1) .* x4z)) .^ 2) .^ (-3 / 2) .* (( ...
  (x1x + (-1) .* x3x) .* ((x1x + (-1) .* x3x) .^ 2 + (x1y + (-1) .*  ...
  x3y) .^ 2 + (x1z + (-1) .* x3z) .^ 2) .^ (-1 / 2) + (x2x + (-1) .* ...
   x4x) .* ((x2x + (-1) .* x4x) .^ 2 + (x2y + (-1) .* x4y) .^ 2 + ( ...
  x2z + (-1) .* x4z) .^ 2) .^ (-1 / 2)) .^ 2 + ((x1y + (-1) .* x3y)  ...
  .* ((x1x + (-1) .* x3x) .^ 2 + (x1y + (-1) .* x3y) .^ 2 + (x1z + ( ...
  -1) .* x3z) .^ 2) .^ (-1 / 2) + (x2y + (-1) .* x4y) .* ((x2x + ( ...
  -1) .* x4x) .^ 2 + (x2y + (-1) .* x4y) .^ 2 + (x2z + (-1) .* x4z)  ...
  .^ 2) .^ (-1 / 2)) .^ 2 + (((x1x + (-1) .* x3x) .^ 2 + (x1y + (-1) ...
   .* x3y) .^ 2 + (x1z + (-1) .* x3z) .^ 2) .^ (-1 / 2) .* (x1z + ( ...
  -1) .* x3z) + ((x2x + (-1) .* x4x) .^ 2 + (x2y + (-1) .* x4y) .^  ...
  2 + (x2z + (-1) .* x4z) .^ 2) .^ (-1 / 2) .* (x2z + (-1) .* x4z))  ...
  .^ 2) .^ (-1 / 2) .* ((x1z + (-1) .* x3z) .* (x2x + (-1) .* x4x) + ...
   (-1) .* (x1x + (-1) .* x3x) .* (x2z + (-1) .* x4z)) .* (2 .* (( ...
  -1) .* x2x + x4x) .* (((-1) .* x1y + x3y) .* (x2x + (-1) .* x4x) + ...
   (x1x + (-1) .* x3x) .* (x2y + (-1) .* x4y)) + 2 .* (((-1) .* x1z  ...
  + x3z) .* (x2y + (-1) .* x4y) + (x1y + (-1) .* x3y) .* (x2z + (-1) ...
   .* x4z)) .* (x2z + (-1) .* x4z)) .* (((x1x + (-1) .* x3x) .^ 2 +  ...
  (x1y + (-1) .* x3y) .^ 2 + (x1z + (-1) .* x3z) .^ 2) .^ (-1 / 2)  ...
  .* (x1z + (-1) .* x3z) + ((x2x + (-1) .* x4x) .^ 2 + (x2y + (-1)  ...
  .* x4y) .^ 2 + (x2z + (-1) .* x4z) .^ 2) .^ (-1 / 2) .* (x2z + ( ...
  -1) .* x4z)),(x1y + (-1) .* x3y) .* ((x1x + (-1) .* x3x) .^ 2 + ( ...
  x1y + (-1) .* x3y) .^ 2 + (x1z + (-1) .* x3z) .^ 2) .^ (-3 / 2) .* ...
   (x1z + (-1) .* x3z) .* (((-1) .* x1y + x3y) .* (x2x + (-1) .*  ...
  x4x) + (x1x + (-1) .* x3x) .* (x2y + (-1) .* x4y)) .* ((((-1) .*  ...
  x1y + x3y) .* (x2x + (-1) .* x4x) + (x1x + (-1) .* x3x) .* (x2y +  ...
  (-1) .* x4y)) .^ 2 + ((x1z + (-1) .* x3z) .* (x2x + (-1) .* x4x) + ...
   (-1) .* (x1x + (-1) .* x3x) .* (x2z + (-1) .* x4z)) .^ 2 + (((-1) ...
   .* x1z + x3z) .* (x2y + (-1) .* x4y) + (x1y + (-1) .* x3y) .* ( ...
  x2z + (-1) .* x4z)) .^ 2) .^ (-1 / 2) .* (((x1x + (-1) .* x3x) .*  ...
  ((x1x + (-1) .* x3x) .^ 2 + (x1y + (-1) .* x3y) .^ 2 + (x1z + (-1) ...
   .* x3z) .^ 2) .^ (-1 / 2) + (x2x + (-1) .* x4x) .* ((x2x + (-1)  ...
  .* x4x) .^ 2 + (x2y + (-1) .* x4y) .^ 2 + (x2z + (-1) .* x4z) .^  ...
  2) .^ (-1 / 2)) .^ 2 + ((x1y + (-1) .* x3y) .* ((x1x + (-1) .*  ...
  x3x) .^ 2 + (x1y + (-1) .* x3y) .^ 2 + (x1z + (-1) .* x3z) .^ 2)  ...
  .^ (-1 / 2) + (x2y + (-1) .* x4y) .* ((x2x + (-1) .* x4x) .^ 2 + ( ...
  x2y + (-1) .* x4y) .^ 2 + (x2z + (-1) .* x4z) .^ 2) .^ (-1 / 2))  ...
  .^ 2 + (((x1x + (-1) .* x3x) .^ 2 + (x1y + (-1) .* x3y) .^ 2 + ( ...
  x1z + (-1) .* x3z) .^ 2) .^ (-1 / 2) .* (x1z + (-1) .* x3z) + (( ...
  x2x + (-1) .* x4x) .^ 2 + (x2y + (-1) .* x4y) .^ 2 + (x2z + (-1)  ...
  .* x4z) .^ 2) .^ (-1 / 2) .* (x2z + (-1) .* x4z)) .^ 2) .^ (-1 /  ...
  2) + (1 / 2) .* (((-1) .* x1y + x3y) .* (x2x + (-1) .* x4x) + ( ...
  x1x + (-1) .* x3x) .* (x2y + (-1) .* x4y)) .* ((((-1) .* x1y +  ...
  x3y) .* (x2x + (-1) .* x4x) + (x1x + (-1) .* x3x) .* (x2y + (-1)  ...
  .* x4y)) .^ 2 + ((x1z + (-1) .* x3z) .* (x2x + (-1) .* x4x) + (-1) ...
   .* (x1x + (-1) .* x3x) .* (x2z + (-1) .* x4z)) .^ 2 + (((-1) .*  ...
  x1z + x3z) .* (x2y + (-1) .* x4y) + (x1y + (-1) .* x3y) .* (x2z +  ...
  (-1) .* x4z)) .^ 2) .^ (-1 / 2) .* ((-2) .* (x1x + (-1) .* x3x) .* ...
   ((x1x + (-1) .* x3x) .^ 2 + (x1y + (-1) .* x3y) .^ 2 + (x1z + ( ...
  -1) .* x3z) .^ 2) .^ (-3 / 2) .* (x1z + (-1) .* x3z) .* ((x1x + ( ...
  -1) .* x3x) .* ((x1x + (-1) .* x3x) .^ 2 + (x1y + (-1) .* x3y) .^  ...
  2 + (x1z + (-1) .* x3z) .^ 2) .^ (-1 / 2) + (x2x + (-1) .* x4x) .* ...
   ((x2x + (-1) .* x4x) .^ 2 + (x2y + (-1) .* x4y) .^ 2 + (x2z + ( ...
  -1) .* x4z) .^ 2) .^ (-1 / 2)) + (-2) .* (x1y + (-1) .* x3y) .* (( ...
  x1x + (-1) .* x3x) .^ 2 + (x1y + (-1) .* x3y) .^ 2 + (x1z + (-1)  ...
  .* x3z) .^ 2) .^ (-3 / 2) .* (x1z + (-1) .* x3z) .* ((x1y + (-1)  ...
  .* x3y) .* ((x1x + (-1) .* x3x) .^ 2 + (x1y + (-1) .* x3y) .^ 2 +  ...
  (x1z + (-1) .* x3z) .^ 2) .^ (-1 / 2) + (x2y + (-1) .* x4y) .* (( ...
  x2x + (-1) .* x4x) .^ 2 + (x2y + (-1) .* x4y) .^ 2 + (x2z + (-1)  ...
  .* x4z) .^ 2) .^ (-1 / 2)) + 2 .* (((x1x + (-1) .* x3x) .^ 2 + ( ...
  x1y + (-1) .* x3y) .^ 2 + (x1z + (-1) .* x3z) .^ 2) .^ (-1 / 2) +  ...
  (-1) .* ((x1x + (-1) .* x3x) .^ 2 + (x1y + (-1) .* x3y) .^ 2 + ( ...
  x1z + (-1) .* x3z) .^ 2) .^ (-3 / 2) .* (x1z + (-1) .* x3z) .^ 2)  ...
  .* (((x1x + (-1) .* x3x) .^ 2 + (x1y + (-1) .* x3y) .^ 2 + (x1z +  ...
  (-1) .* x3z) .^ 2) .^ (-1 / 2) .* (x1z + (-1) .* x3z) + ((x2x + ( ...
  -1) .* x4x) .^ 2 + (x2y + (-1) .* x4y) .^ 2 + (x2z + (-1) .* x4z)  ...
  .^ 2) .^ (-1 / 2) .* (x2z + (-1) .* x4z))) .* (((x1x + (-1) .*  ...
  x3x) .* ((x1x + (-1) .* x3x) .^ 2 + (x1y + (-1) .* x3y) .^ 2 + ( ...
  x1z + (-1) .* x3z) .^ 2) .^ (-1 / 2) + (x2x + (-1) .* x4x) .* (( ...
  x2x + (-1) .* x4x) .^ 2 + (x2y + (-1) .* x4y) .^ 2 + (x2z + (-1)  ...
  .* x4z) .^ 2) .^ (-1 / 2)) .^ 2 + ((x1y + (-1) .* x3y) .* ((x1x +  ...
  (-1) .* x3x) .^ 2 + (x1y + (-1) .* x3y) .^ 2 + (x1z + (-1) .* x3z) ...
   .^ 2) .^ (-1 / 2) + (x2y + (-1) .* x4y) .* ((x2x + (-1) .* x4x)  ...
  .^ 2 + (x2y + (-1) .* x4y) .^ 2 + (x2z + (-1) .* x4z) .^ 2) .^ ( ...
  -1 / 2)) .^ 2 + (((x1x + (-1) .* x3x) .^ 2 + (x1y + (-1) .* x3y)  ...
  .^ 2 + (x1z + (-1) .* x3z) .^ 2) .^ (-1 / 2) .* (x1z + (-1) .*  ...
  x3z) + ((x2x + (-1) .* x4x) .^ 2 + (x2y + (-1) .* x4y) .^ 2 + ( ...
  x2z + (-1) .* x4z) .^ 2) .^ (-1 / 2) .* (x2z + (-1) .* x4z)) .^ 2) ...
   .^ (-3 / 2) .* ((x1y + (-1) .* x3y) .* ((x1x + (-1) .* x3x) .^ 2  ...
  + (x1y + (-1) .* x3y) .^ 2 + (x1z + (-1) .* x3z) .^ 2) .^ (-1 / 2) ...
   + (x2y + (-1) .* x4y) .* ((x2x + (-1) .* x4x) .^ 2 + (x2y + (-1)  ...
  .* x4y) .^ 2 + (x2z + (-1) .* x4z) .^ 2) .^ (-1 / 2)) + (1 / 2) .* ...
   (((-1) .* x1y + x3y) .* (x2x + (-1) .* x4x) + (x1x + (-1) .* x3x) ...
   .* (x2y + (-1) .* x4y)) .* (2 .* (x2x + (-1) .* x4x) .* ((x1z + ( ...
  -1) .* x3z) .* (x2x + (-1) .* x4x) + (-1) .* (x1x + (-1) .* x3x)  ...
  .* (x2z + (-1) .* x4z)) + 2 .* ((-1) .* x2y + x4y) .* (((-1) .*  ...
  x1z + x3z) .* (x2y + (-1) .* x4y) + (x1y + (-1) .* x3y) .* (x2z +  ...
  (-1) .* x4z))) .* ((((-1) .* x1y + x3y) .* (x2x + (-1) .* x4x) + ( ...
  x1x + (-1) .* x3x) .* (x2y + (-1) .* x4y)) .^ 2 + ((x1z + (-1) .*  ...
  x3z) .* (x2x + (-1) .* x4x) + (-1) .* (x1x + (-1) .* x3x) .* (x2z  ...
  + (-1) .* x4z)) .^ 2 + (((-1) .* x1z + x3z) .* (x2y + (-1) .* x4y) ...
   + (x1y + (-1) .* x3y) .* (x2z + (-1) .* x4z)) .^ 2) .^ (-3 / 2)  ...
  .* (((x1x + (-1) .* x3x) .* ((x1x + (-1) .* x3x) .^ 2 + (x1y + ( ...
  -1) .* x3y) .^ 2 + (x1z + (-1) .* x3z) .^ 2) .^ (-1 / 2) + (x2x +  ...
  (-1) .* x4x) .* ((x2x + (-1) .* x4x) .^ 2 + (x2y + (-1) .* x4y)  ...
  .^ 2 + (x2z + (-1) .* x4z) .^ 2) .^ (-1 / 2)) .^ 2 + ((x1y + (-1)  ...
  .* x3y) .* ((x1x + (-1) .* x3x) .^ 2 + (x1y + (-1) .* x3y) .^ 2 +  ...
  (x1z + (-1) .* x3z) .^ 2) .^ (-1 / 2) + (x2y + (-1) .* x4y) .* (( ...
  x2x + (-1) .* x4x) .^ 2 + (x2y + (-1) .* x4y) .^ 2 + (x2z + (-1)  ...
  .* x4z) .^ 2) .^ (-1 / 2)) .^ 2 + (((x1x + (-1) .* x3x) .^ 2 + ( ...
  x1y + (-1) .* x3y) .^ 2 + (x1z + (-1) .* x3z) .^ 2) .^ (-1 / 2) .* ...
   (x1z + (-1) .* x3z) + ((x2x + (-1) .* x4x) .^ 2 + (x2y + (-1) .*  ...
  x4y) .^ 2 + (x2z + (-1) .* x4z) .^ 2) .^ (-1 / 2) .* (x2z + (-1)  ...
  .* x4z)) .^ 2) .^ (-1 / 2) .* ((x1y + (-1) .* x3y) .* ((x1x + (-1) ...
   .* x3x) .^ 2 + (x1y + (-1) .* x3y) .^ 2 + (x1z + (-1) .* x3z) .^  ...
  2) .^ (-1 / 2) + (x2y + (-1) .* x4y) .* ((x2x + (-1) .* x4x) .^ 2  ...
  + (x2y + (-1) .* x4y) .^ 2 + (x2z + (-1) .* x4z) .^ 2) .^ (-1 / 2) ...
  ) + (((x1x + (-1) .* x3x) .^ 2 + (x1y + (-1) .* x3y) .^ 2 + (x1z + ...
   (-1) .* x3z) .^ 2) .^ (-1 / 2) + (-1) .* ((x1x + (-1) .* x3x) .^  ...
  2 + (x1y + (-1) .* x3y) .^ 2 + (x1z + (-1) .* x3z) .^ 2) .^ (-3 /  ...
  2) .* (x1z + (-1) .* x3z) .^ 2) .* ((((-1) .* x1y + x3y) .* (x2x + ...
   (-1) .* x4x) + (x1x + (-1) .* x3x) .* (x2y + (-1) .* x4y)) .^ 2 + ...
   ((x1z + (-1) .* x3z) .* (x2x + (-1) .* x4x) + (-1) .* (x1x + (-1) ...
   .* x3x) .* (x2z + (-1) .* x4z)) .^ 2 + (((-1) .* x1z + x3z) .* ( ...
  x2y + (-1) .* x4y) + (x1y + (-1) .* x3y) .* (x2z + (-1) .* x4z))  ...
  .^ 2) .^ (-1 / 2) .* (((x1x + (-1) .* x3x) .* ((x1x + (-1) .* x3x) ...
   .^ 2 + (x1y + (-1) .* x3y) .^ 2 + (x1z + (-1) .* x3z) .^ 2) .^ ( ...
  -1 / 2) + (x2x + (-1) .* x4x) .* ((x2x + (-1) .* x4x) .^ 2 + (x2y  ...
  + (-1) .* x4y) .^ 2 + (x2z + (-1) .* x4z) .^ 2) .^ (-1 / 2)) .^ 2  ...
  + ((x1y + (-1) .* x3y) .* ((x1x + (-1) .* x3x) .^ 2 + (x1y + (-1)  ...
  .* x3y) .^ 2 + (x1z + (-1) .* x3z) .^ 2) .^ (-1 / 2) + (x2y + (-1) ...
   .* x4y) .* ((x2x + (-1) .* x4x) .^ 2 + (x2y + (-1) .* x4y) .^ 2 + ...
   (x2z + (-1) .* x4z) .^ 2) .^ (-1 / 2)) .^ 2 + (((x1x + (-1) .*  ...
  x3x) .^ 2 + (x1y + (-1) .* x3y) .^ 2 + (x1z + (-1) .* x3z) .^ 2)  ...
  .^ (-1 / 2) .* (x1z + (-1) .* x3z) + ((x2x + (-1) .* x4x) .^ 2 + ( ...
  x2y + (-1) .* x4y) .^ 2 + (x2z + (-1) .* x4z) .^ 2) .^ (-1 / 2) .* ...
   (x2z + (-1) .* x4z)) .^ 2) .^ (-1 / 2) .* ((x1z + (-1) .* x3z) .* ...
   (x2x + (-1) .* x4x) + (-1) .* (x1x + (-1) .* x3x) .* (x2z + (-1)  ...
  .* x4z)) + (x2x + (-1) .* x4x) .* ((((-1) .* x1y + x3y) .* (x2x +  ...
  (-1) .* x4x) + (x1x + (-1) .* x3x) .* (x2y + (-1) .* x4y)) .^ 2 +  ...
  ((x1z + (-1) .* x3z) .* (x2x + (-1) .* x4x) + (-1) .* (x1x + (-1)  ...
  .* x3x) .* (x2z + (-1) .* x4z)) .^ 2 + (((-1) .* x1z + x3z) .* ( ...
  x2y + (-1) .* x4y) + (x1y + (-1) .* x3y) .* (x2z + (-1) .* x4z))  ...
  .^ 2) .^ (-1 / 2) .* (((x1x + (-1) .* x3x) .* ((x1x + (-1) .* x3x) ...
   .^ 2 + (x1y + (-1) .* x3y) .^ 2 + (x1z + (-1) .* x3z) .^ 2) .^ ( ...
  -1 / 2) + (x2x + (-1) .* x4x) .* ((x2x + (-1) .* x4x) .^ 2 + (x2y  ...
  + (-1) .* x4y) .^ 2 + (x2z + (-1) .* x4z) .^ 2) .^ (-1 / 2)) .^ 2  ...
  + ((x1y + (-1) .* x3y) .* ((x1x + (-1) .* x3x) .^ 2 + (x1y + (-1)  ...
  .* x3y) .^ 2 + (x1z + (-1) .* x3z) .^ 2) .^ (-1 / 2) + (x2y + (-1) ...
   .* x4y) .* ((x2x + (-1) .* x4x) .^ 2 + (x2y + (-1) .* x4y) .^ 2 + ...
   (x2z + (-1) .* x4z) .^ 2) .^ (-1 / 2)) .^ 2 + (((x1x + (-1) .*  ...
  x3x) .^ 2 + (x1y + (-1) .* x3y) .^ 2 + (x1z + (-1) .* x3z) .^ 2)  ...
  .^ (-1 / 2) .* (x1z + (-1) .* x3z) + ((x2x + (-1) .* x4x) .^ 2 + ( ...
  x2y + (-1) .* x4y) .^ 2 + (x2z + (-1) .* x4z) .^ 2) .^ (-1 / 2) .* ...
   (x2z + (-1) .* x4z)) .^ 2) .^ (-1 / 2) .* (((x1x + (-1) .* x3x)  ...
  .^ 2 + (x1y + (-1) .* x3y) .^ 2 + (x1z + (-1) .* x3z) .^ 2) .^ ( ...
  -1 / 2) .* (x1z + (-1) .* x3z) + ((x2x + (-1) .* x4x) .^ 2 + (x2y  ...
  + (-1) .* x4y) .^ 2 + (x2z + (-1) .* x4z) .^ 2) .^ (-1 / 2) .* ( ...
  x2z + (-1) .* x4z)) + (-1 / 2) .* ((((-1) .* x1y + x3y) .* (x2x +  ...
  (-1) .* x4x) + (x1x + (-1) .* x3x) .* (x2y + (-1) .* x4y)) .^ 2 +  ...
  ((x1z + (-1) .* x3z) .* (x2x + (-1) .* x4x) + (-1) .* (x1x + (-1)  ...
  .* x3x) .* (x2z + (-1) .* x4z)) .^ 2 + (((-1) .* x1z + x3z) .* ( ...
  x2y + (-1) .* x4y) + (x1y + (-1) .* x3y) .* (x2z + (-1) .* x4z))  ...
  .^ 2) .^ (-1 / 2) .* ((-2) .* (x1x + (-1) .* x3x) .* ((x1x + (-1)  ...
  .* x3x) .^ 2 + (x1y + (-1) .* x3y) .^ 2 + (x1z + (-1) .* x3z) .^  ...
  2) .^ (-3 / 2) .* (x1z + (-1) .* x3z) .* ((x1x + (-1) .* x3x) .* ( ...
  (x1x + (-1) .* x3x) .^ 2 + (x1y + (-1) .* x3y) .^ 2 + (x1z + (-1)  ...
  .* x3z) .^ 2) .^ (-1 / 2) + (x2x + (-1) .* x4x) .* ((x2x + (-1) .* ...
   x4x) .^ 2 + (x2y + (-1) .* x4y) .^ 2 + (x2z + (-1) .* x4z) .^ 2)  ...
  .^ (-1 / 2)) + (-2) .* (x1y + (-1) .* x3y) .* ((x1x + (-1) .* x3x) ...
   .^ 2 + (x1y + (-1) .* x3y) .^ 2 + (x1z + (-1) .* x3z) .^ 2) .^ ( ...
  -3 / 2) .* (x1z + (-1) .* x3z) .* ((x1y + (-1) .* x3y) .* ((x1x +  ...
  (-1) .* x3x) .^ 2 + (x1y + (-1) .* x3y) .^ 2 + (x1z + (-1) .* x3z) ...
   .^ 2) .^ (-1 / 2) + (x2y + (-1) .* x4y) .* ((x2x + (-1) .* x4x)  ...
  .^ 2 + (x2y + (-1) .* x4y) .^ 2 + (x2z + (-1) .* x4z) .^ 2) .^ ( ...
  -1 / 2)) + 2 .* (((x1x + (-1) .* x3x) .^ 2 + (x1y + (-1) .* x3y)  ...
  .^ 2 + (x1z + (-1) .* x3z) .^ 2) .^ (-1 / 2) + (-1) .* ((x1x + ( ...
  -1) .* x3x) .^ 2 + (x1y + (-1) .* x3y) .^ 2 + (x1z + (-1) .* x3z)  ...
  .^ 2) .^ (-3 / 2) .* (x1z + (-1) .* x3z) .^ 2) .* (((x1x + (-1) .* ...
   x3x) .^ 2 + (x1y + (-1) .* x3y) .^ 2 + (x1z + (-1) .* x3z) .^ 2)  ...
  .^ (-1 / 2) .* (x1z + (-1) .* x3z) + ((x2x + (-1) .* x4x) .^ 2 + ( ...
  x2y + (-1) .* x4y) .^ 2 + (x2z + (-1) .* x4z) .^ 2) .^ (-1 / 2) .* ...
   (x2z + (-1) .* x4z))) .* (((x1x + (-1) .* x3x) .* ((x1x + (-1) .* ...
   x3x) .^ 2 + (x1y + (-1) .* x3y) .^ 2 + (x1z + (-1) .* x3z) .^ 2)  ...
  .^ (-1 / 2) + (x2x + (-1) .* x4x) .* ((x2x + (-1) .* x4x) .^ 2 + ( ...
  x2y + (-1) .* x4y) .^ 2 + (x2z + (-1) .* x4z) .^ 2) .^ (-1 / 2))  ...
  .^ 2 + ((x1y + (-1) .* x3y) .* ((x1x + (-1) .* x3x) .^ 2 + (x1y +  ...
  (-1) .* x3y) .^ 2 + (x1z + (-1) .* x3z) .^ 2) .^ (-1 / 2) + (x2y + ...
   (-1) .* x4y) .* ((x2x + (-1) .* x4x) .^ 2 + (x2y + (-1) .* x4y)  ...
  .^ 2 + (x2z + (-1) .* x4z) .^ 2) .^ (-1 / 2)) .^ 2 + (((x1x + (-1) ...
   .* x3x) .^ 2 + (x1y + (-1) .* x3y) .^ 2 + (x1z + (-1) .* x3z) .^  ...
  2) .^ (-1 / 2) .* (x1z + (-1) .* x3z) + ((x2x + (-1) .* x4x) .^ 2  ...
  + (x2y + (-1) .* x4y) .^ 2 + (x2z + (-1) .* x4z) .^ 2) .^ (-1 / 2) ...
   .* (x2z + (-1) .* x4z)) .^ 2) .^ (-3 / 2) .* ((x1z + (-1) .* x3z) ...
   .* (x2x + (-1) .* x4x) + (-1) .* (x1x + (-1) .* x3x) .* (x2z + ( ...
  -1) .* x4z)) .* (((x1x + (-1) .* x3x) .^ 2 + (x1y + (-1) .* x3y)  ...
  .^ 2 + (x1z + (-1) .* x3z) .^ 2) .^ (-1 / 2) .* (x1z + (-1) .*  ...
  x3z) + ((x2x + (-1) .* x4x) .^ 2 + (x2y + (-1) .* x4y) .^ 2 + ( ...
  x2z + (-1) .* x4z) .^ 2) .^ (-1 / 2) .* (x2z + (-1) .* x4z)) + ( ...
  -1 / 2) .* (2 .* (x2x + (-1) .* x4x) .* ((x1z + (-1) .* x3z) .* ( ...
  x2x + (-1) .* x4x) + (-1) .* (x1x + (-1) .* x3x) .* (x2z + (-1) .* ...
   x4z)) + 2 .* ((-1) .* x2y + x4y) .* (((-1) .* x1z + x3z) .* (x2y  ...
  + (-1) .* x4y) + (x1y + (-1) .* x3y) .* (x2z + (-1) .* x4z))) .* ( ...
  (((-1) .* x1y + x3y) .* (x2x + (-1) .* x4x) + (x1x + (-1) .* x3x)  ...
  .* (x2y + (-1) .* x4y)) .^ 2 + ((x1z + (-1) .* x3z) .* (x2x + (-1) ...
   .* x4x) + (-1) .* (x1x + (-1) .* x3x) .* (x2z + (-1) .* x4z)) .^  ...
  2 + (((-1) .* x1z + x3z) .* (x2y + (-1) .* x4y) + (x1y + (-1) .*  ...
  x3y) .* (x2z + (-1) .* x4z)) .^ 2) .^ (-3 / 2) .* (((x1x + (-1) .* ...
   x3x) .* ((x1x + (-1) .* x3x) .^ 2 + (x1y + (-1) .* x3y) .^ 2 + ( ...
  x1z + (-1) .* x3z) .^ 2) .^ (-1 / 2) + (x2x + (-1) .* x4x) .* (( ...
  x2x + (-1) .* x4x) .^ 2 + (x2y + (-1) .* x4y) .^ 2 + (x2z + (-1)  ...
  .* x4z) .^ 2) .^ (-1 / 2)) .^ 2 + ((x1y + (-1) .* x3y) .* ((x1x +  ...
  (-1) .* x3x) .^ 2 + (x1y + (-1) .* x3y) .^ 2 + (x1z + (-1) .* x3z) ...
   .^ 2) .^ (-1 / 2) + (x2y + (-1) .* x4y) .* ((x2x + (-1) .* x4x)  ...
  .^ 2 + (x2y + (-1) .* x4y) .^ 2 + (x2z + (-1) .* x4z) .^ 2) .^ ( ...
  -1 / 2)) .^ 2 + (((x1x + (-1) .* x3x) .^ 2 + (x1y + (-1) .* x3y)  ...
  .^ 2 + (x1z + (-1) .* x3z) .^ 2) .^ (-1 / 2) .* (x1z + (-1) .*  ...
  x3z) + ((x2x + (-1) .* x4x) .^ 2 + (x2y + (-1) .* x4y) .^ 2 + ( ...
  x2z + (-1) .* x4z) .^ 2) .^ (-1 / 2) .* (x2z + (-1) .* x4z)) .^ 2) ...
   .^ (-1 / 2) .* ((x1z + (-1) .* x3z) .* (x2x + (-1) .* x4x) + (-1) ...
   .* (x1x + (-1) .* x3x) .* (x2z + (-1) .* x4z)) .* (((x1x + (-1)  ...
  .* x3x) .^ 2 + (x1y + (-1) .* x3y) .^ 2 + (x1z + (-1) .* x3z) .^  ...
  2) .^ (-1 / 2) .* (x1z + (-1) .* x3z) + ((x2x + (-1) .* x4x) .^ 2  ...
  + (x2y + (-1) .* x4y) .^ 2 + (x2z + (-1) .* x4z) .^ 2) .^ (-1 / 2) ...
   .* (x2z + (-1) .* x4z)),(1 / 2) .* (((-1) .* x1y + x3y) .* (x2x + ...
   (-1) .* x4x) + (x1x + (-1) .* x3x) .* (x2y + (-1) .* x4y)) .* (2  ...
  .* ((-1) .* x1y + x3y) .* (((-1) .* x1y + x3y) .* (x2x + (-1) .*  ...
  x4x) + (x1x + (-1) .* x3x) .* (x2y + (-1) .* x4y)) + 2 .* (x1z + ( ...
  -1) .* x3z) .* ((x1z + (-1) .* x3z) .* (x2x + (-1) .* x4x) + (-1)  ...
  .* (x1x + (-1) .* x3x) .* (x2z + (-1) .* x4z))) .* ((((-1) .* x1y  ...
  + x3y) .* (x2x + (-1) .* x4x) + (x1x + (-1) .* x3x) .* (x2y + (-1) ...
   .* x4y)) .^ 2 + ((x1z + (-1) .* x3z) .* (x2x + (-1) .* x4x) + ( ...
  -1) .* (x1x + (-1) .* x3x) .* (x2z + (-1) .* x4z)) .^ 2 + (((-1)  ...
  .* x1z + x3z) .* (x2y + (-1) .* x4y) + (x1y + (-1) .* x3y) .* ( ...
  x2z + (-1) .* x4z)) .^ 2) .^ (-3 / 2) .* (((x1x + (-1) .* x3x) .*  ...
  ((x1x + (-1) .* x3x) .^ 2 + (x1y + (-1) .* x3y) .^ 2 + (x1z + (-1) ...
   .* x3z) .^ 2) .^ (-1 / 2) + (x2x + (-1) .* x4x) .* ((x2x + (-1)  ...
  .* x4x) .^ 2 + (x2y + (-1) .* x4y) .^ 2 + (x2z + (-1) .* x4z) .^  ...
  2) .^ (-1 / 2)) .^ 2 + ((x1y + (-1) .* x3y) .* ((x1x + (-1) .*  ...
  x3x) .^ 2 + (x1y + (-1) .* x3y) .^ 2 + (x1z + (-1) .* x3z) .^ 2)  ...
  .^ (-1 / 2) + (x2y + (-1) .* x4y) .* ((x2x + (-1) .* x4x) .^ 2 + ( ...
  x2y + (-1) .* x4y) .^ 2 + (x2z + (-1) .* x4z) .^ 2) .^ (-1 / 2))  ...
  .^ 2 + (((x1x + (-1) .* x3x) .^ 2 + (x1y + (-1) .* x3y) .^ 2 + ( ...
  x1z + (-1) .* x3z) .^ 2) .^ (-1 / 2) .* (x1z + (-1) .* x3z) + (( ...
  x2x + (-1) .* x4x) .^ 2 + (x2y + (-1) .* x4y) .^ 2 + (x2z + (-1)  ...
  .* x4z) .^ 2) .^ (-1 / 2) .* (x2z + (-1) .* x4z)) .^ 2) .^ (-1 /  ...
  2) .* ((x1y + (-1) .* x3y) .* ((x1x + (-1) .* x3x) .^ 2 + (x1y + ( ...
  -1) .* x3y) .^ 2 + (x1z + (-1) .* x3z) .^ 2) .^ (-1 / 2) + (x2y +  ...
  (-1) .* x4y) .* ((x2x + (-1) .* x4x) .^ 2 + (x2y + (-1) .* x4y)  ...
  .^ 2 + (x2z + (-1) .* x4z) .^ 2) .^ (-1 / 2)) + (-1) .* ((-1) .*  ...
  x1y + x3y) .* ((((-1) .* x1y + x3y) .* (x2x + (-1) .* x4x) + (x1x  ...
  + (-1) .* x3x) .* (x2y + (-1) .* x4y)) .^ 2 + ((x1z + (-1) .* x3z) ...
   .* (x2x + (-1) .* x4x) + (-1) .* (x1x + (-1) .* x3x) .* (x2z + ( ...
  -1) .* x4z)) .^ 2 + (((-1) .* x1z + x3z) .* (x2y + (-1) .* x4y) +  ...
  (x1y + (-1) .* x3y) .* (x2z + (-1) .* x4z)) .^ 2) .^ (-1 / 2) .* ( ...
  ((x1x + (-1) .* x3x) .* ((x1x + (-1) .* x3x) .^ 2 + (x1y + (-1) .* ...
   x3y) .^ 2 + (x1z + (-1) .* x3z) .^ 2) .^ (-1 / 2) + (x2x + (-1)  ...
  .* x4x) .* ((x2x + (-1) .* x4x) .^ 2 + (x2y + (-1) .* x4y) .^ 2 +  ...
  (x2z + (-1) .* x4z) .^ 2) .^ (-1 / 2)) .^ 2 + ((x1y + (-1) .* x3y) ...
   .* ((x1x + (-1) .* x3x) .^ 2 + (x1y + (-1) .* x3y) .^ 2 + (x1z +  ...
  (-1) .* x3z) .^ 2) .^ (-1 / 2) + (x2y + (-1) .* x4y) .* ((x2x + ( ...
  -1) .* x4x) .^ 2 + (x2y + (-1) .* x4y) .^ 2 + (x2z + (-1) .* x4z)  ...
  .^ 2) .^ (-1 / 2)) .^ 2 + (((x1x + (-1) .* x3x) .^ 2 + (x1y + (-1) ...
   .* x3y) .^ 2 + (x1z + (-1) .* x3z) .^ 2) .^ (-1 / 2) .* (x1z + ( ...
  -1) .* x3z) + ((x2x + (-1) .* x4x) .^ 2 + (x2y + (-1) .* x4y) .^  ...
  2 + (x2z + (-1) .* x4z) .^ 2) .^ (-1 / 2) .* (x2z + (-1) .* x4z))  ...
  .^ 2) .^ (-1 / 2) .* ((x1y + (-1) .* x3y) .* ((x1x + (-1) .* x3x)  ...
  .^ 2 + (x1y + (-1) .* x3y) .^ 2 + (x1z + (-1) .* x3z) .^ 2) .^ ( ...
  -1 / 2) + (x2y + (-1) .* x4y) .* ((x2x + (-1) .* x4x) .^ 2 + (x2y  ...
  + (-1) .* x4y) .^ 2 + (x2z + (-1) .* x4z) .^ 2) .^ (-1 / 2)) + (1  ...
  / 2) .* (((-1) .* x1y + x3y) .* (x2x + (-1) .* x4x) + (x1x + (-1)  ...
  .* x3x) .* (x2y + (-1) .* x4y)) .* ((((-1) .* x1y + x3y) .* (x2x + ...
   (-1) .* x4x) + (x1x + (-1) .* x3x) .* (x2y + (-1) .* x4y)) .^ 2 + ...
   ((x1z + (-1) .* x3z) .* (x2x + (-1) .* x4x) + (-1) .* (x1x + (-1) ...
   .* x3x) .* (x2z + (-1) .* x4z)) .^ 2 + (((-1) .* x1z + x3z) .* ( ...
  x2y + (-1) .* x4y) + (x1y + (-1) .* x3y) .* (x2z + (-1) .* x4z))  ...
  .^ 2) .^ (-1 / 2) .* (((x1x + (-1) .* x3x) .* ((x1x + (-1) .* x3x) ...
   .^ 2 + (x1y + (-1) .* x3y) .^ 2 + (x1z + (-1) .* x3z) .^ 2) .^ ( ...
  -1 / 2) + (x2x + (-1) .* x4x) .* ((x2x + (-1) .* x4x) .^ 2 + (x2y  ...
  + (-1) .* x4y) .^ 2 + (x2z + (-1) .* x4z) .^ 2) .^ (-1 / 2)) .^ 2  ...
  + ((x1y + (-1) .* x3y) .* ((x1x + (-1) .* x3x) .^ 2 + (x1y + (-1)  ...
  .* x3y) .^ 2 + (x1z + (-1) .* x3z) .^ 2) .^ (-1 / 2) + (x2y + (-1) ...
   .* x4y) .* ((x2x + (-1) .* x4x) .^ 2 + (x2y + (-1) .* x4y) .^ 2 + ...
   (x2z + (-1) .* x4z) .^ 2) .^ (-1 / 2)) .^ 2 + (((x1x + (-1) .*  ...
  x3x) .^ 2 + (x1y + (-1) .* x3y) .^ 2 + (x1z + (-1) .* x3z) .^ 2)  ...
  .^ (-1 / 2) .* (x1z + (-1) .* x3z) + ((x2x + (-1) .* x4x) .^ 2 + ( ...
  x2y + (-1) .* x4y) .^ 2 + (x2z + (-1) .* x4z) .^ 2) .^ (-1 / 2) .* ...
   (x2z + (-1) .* x4z)) .^ 2) .^ (-3 / 2) .* ((x1y + (-1) .* x3y) .* ...
   ((x1x + (-1) .* x3x) .^ 2 + (x1y + (-1) .* x3y) .^ 2 + (x1z + ( ...
  -1) .* x3z) .^ 2) .^ (-1 / 2) + (x2y + (-1) .* x4y) .* ((x2x + ( ...
  -1) .* x4x) .^ 2 + (x2y + (-1) .* x4y) .^ 2 + (x2z + (-1) .* x4z)  ...
  .^ 2) .^ (-1 / 2)) .* (2 .* ((-1) .* (x2x + (-1) .* x4x) .^ 2 .* ( ...
  (x2x + (-1) .* x4x) .^ 2 + (x2y + (-1) .* x4y) .^ 2 + (x2z + (-1)  ...
  .* x4z) .^ 2) .^ (-3 / 2) + ((x2x + (-1) .* x4x) .^ 2 + (x2y + ( ...
  -1) .* x4y) .^ 2 + (x2z + (-1) .* x4z) .^ 2) .^ (-1 / 2)) .* (( ...
  x1x + (-1) .* x3x) .* ((x1x + (-1) .* x3x) .^ 2 + (x1y + (-1) .*  ...
  x3y) .^ 2 + (x1z + (-1) .* x3z) .^ 2) .^ (-1 / 2) + (x2x + (-1) .* ...
   x4x) .* ((x2x + (-1) .* x4x) .^ 2 + (x2y + (-1) .* x4y) .^ 2 + ( ...
  x2z + (-1) .* x4z) .^ 2) .^ (-1 / 2)) + (-2) .* (x2x + (-1) .*  ...
  x4x) .* (x2y + (-1) .* x4y) .* ((x1y + (-1) .* x3y) .* ((x1x + ( ...
  -1) .* x3x) .^ 2 + (x1y + (-1) .* x3y) .^ 2 + (x1z + (-1) .* x3z)  ...
  .^ 2) .^ (-1 / 2) + (x2y + (-1) .* x4y) .* ((x2x + (-1) .* x4x)  ...
  .^ 2 + (x2y + (-1) .* x4y) .^ 2 + (x2z + (-1) .* x4z) .^ 2) .^ ( ...
  -1 / 2)) .* ((x2x + (-1) .* x4x) .^ 2 + (x2y + (-1) .* x4y) .^ 2 + ...
   (x2z + (-1) .* x4z) .^ 2) .^ (-3 / 2) + (-2) .* (x2x + (-1) .*  ...
  x4x) .* (((x1x + (-1) .* x3x) .^ 2 + (x1y + (-1) .* x3y) .^ 2 + ( ...
  x1z + (-1) .* x3z) .^ 2) .^ (-1 / 2) .* (x1z + (-1) .* x3z) + (( ...
  x2x + (-1) .* x4x) .^ 2 + (x2y + (-1) .* x4y) .^ 2 + (x2z + (-1)  ...
  .* x4z) .^ 2) .^ (-1 / 2) .* (x2z + (-1) .* x4z)) .* ((x2x + (-1)  ...
  .* x4x) .^ 2 + (x2y + (-1) .* x4y) .^ 2 + (x2z + (-1) .* x4z) .^  ...
  2) .^ (-3 / 2) .* (x2z + (-1) .* x4z)) + (x1z + (-1) .* x3z) .* (( ...
  ((-1) .* x1y + x3y) .* (x2x + (-1) .* x4x) + (x1x + (-1) .* x3x)  ...
  .* (x2y + (-1) .* x4y)) .^ 2 + ((x1z + (-1) .* x3z) .* (x2x + (-1) ...
   .* x4x) + (-1) .* (x1x + (-1) .* x3x) .* (x2z + (-1) .* x4z)) .^  ...
  2 + (((-1) .* x1z + x3z) .* (x2y + (-1) .* x4y) + (x1y + (-1) .*  ...
  x3y) .* (x2z + (-1) .* x4z)) .^ 2) .^ (-1 / 2) .* (((x1x + (-1) .* ...
   x3x) .* ((x1x + (-1) .* x3x) .^ 2 + (x1y + (-1) .* x3y) .^ 2 + ( ...
  x1z + (-1) .* x3z) .^ 2) .^ (-1 / 2) + (x2x + (-1) .* x4x) .* (( ...
  x2x + (-1) .* x4x) .^ 2 + (x2y + (-1) .* x4y) .^ 2 + (x2z + (-1)  ...
  .* x4z) .^ 2) .^ (-1 / 2)) .^ 2 + ((x1y + (-1) .* x3y) .* ((x1x +  ...
  (-1) .* x3x) .^ 2 + (x1y + (-1) .* x3y) .^ 2 + (x1z + (-1) .* x3z) ...
   .^ 2) .^ (-1 / 2) + (x2y + (-1) .* x4y) .* ((x2x + (-1) .* x4x)  ...
  .^ 2 + (x2y + (-1) .* x4y) .^ 2 + (x2z + (-1) .* x4z) .^ 2) .^ ( ...
  -1 / 2)) .^ 2 + (((x1x + (-1) .* x3x) .^ 2 + (x1y + (-1) .* x3y)  ...
  .^ 2 + (x1z + (-1) .* x3z) .^ 2) .^ (-1 / 2) .* (x1z + (-1) .*  ...
  x3z) + ((x2x + (-1) .* x4x) .^ 2 + (x2y + (-1) .* x4y) .^ 2 + ( ...
  x2z + (-1) .* x4z) .^ 2) .^ (-1 / 2) .* (x2z + (-1) .* x4z)) .^ 2) ...
   .^ (-1 / 2) .* (((x1x + (-1) .* x3x) .^ 2 + (x1y + (-1) .* x3y)  ...
  .^ 2 + (x1z + (-1) .* x3z) .^ 2) .^ (-1 / 2) .* (x1z + (-1) .*  ...
  x3z) + ((x2x + (-1) .* x4x) .^ 2 + (x2y + (-1) .* x4y) .^ 2 + ( ...
  x2z + (-1) .* x4z) .^ 2) .^ (-1 / 2) .* (x2z + (-1) .* x4z)) + ( ...
  -1 / 2) .* (2 .* ((-1) .* x1y + x3y) .* (((-1) .* x1y + x3y) .* ( ...
  x2x + (-1) .* x4x) + (x1x + (-1) .* x3x) .* (x2y + (-1) .* x4y)) + ...
   2 .* (x1z + (-1) .* x3z) .* ((x1z + (-1) .* x3z) .* (x2x + (-1)  ...
  .* x4x) + (-1) .* (x1x + (-1) .* x3x) .* (x2z + (-1) .* x4z))) .*  ...
  ((((-1) .* x1y + x3y) .* (x2x + (-1) .* x4x) + (x1x + (-1) .* x3x) ...
   .* (x2y + (-1) .* x4y)) .^ 2 + ((x1z + (-1) .* x3z) .* (x2x + ( ...
  -1) .* x4x) + (-1) .* (x1x + (-1) .* x3x) .* (x2z + (-1) .* x4z))  ...
  .^ 2 + (((-1) .* x1z + x3z) .* (x2y + (-1) .* x4y) + (x1y + (-1)  ...
  .* x3y) .* (x2z + (-1) .* x4z)) .^ 2) .^ (-3 / 2) .* (((x1x + (-1) ...
   .* x3x) .* ((x1x + (-1) .* x3x) .^ 2 + (x1y + (-1) .* x3y) .^ 2 + ...
   (x1z + (-1) .* x3z) .^ 2) .^ (-1 / 2) + (x2x + (-1) .* x4x) .* (( ...
  x2x + (-1) .* x4x) .^ 2 + (x2y + (-1) .* x4y) .^ 2 + (x2z + (-1)  ...
  .* x4z) .^ 2) .^ (-1 / 2)) .^ 2 + ((x1y + (-1) .* x3y) .* ((x1x +  ...
  (-1) .* x3x) .^ 2 + (x1y + (-1) .* x3y) .^ 2 + (x1z + (-1) .* x3z) ...
   .^ 2) .^ (-1 / 2) + (x2y + (-1) .* x4y) .* ((x2x + (-1) .* x4x)  ...
  .^ 2 + (x2y + (-1) .* x4y) .^ 2 + (x2z + (-1) .* x4z) .^ 2) .^ ( ...
  -1 / 2)) .^ 2 + (((x1x + (-1) .* x3x) .^ 2 + (x1y + (-1) .* x3y)  ...
  .^ 2 + (x1z + (-1) .* x3z) .^ 2) .^ (-1 / 2) .* (x1z + (-1) .*  ...
  x3z) + ((x2x + (-1) .* x4x) .^ 2 + (x2y + (-1) .* x4y) .^ 2 + ( ...
  x2z + (-1) .* x4z) .^ 2) .^ (-1 / 2) .* (x2z + (-1) .* x4z)) .^ 2) ...
   .^ (-1 / 2) .* ((x1z + (-1) .* x3z) .* (x2x + (-1) .* x4x) + (-1) ...
   .* (x1x + (-1) .* x3x) .* (x2z + (-1) .* x4z)) .* (((x1x + (-1)  ...
  .* x3x) .^ 2 + (x1y + (-1) .* x3y) .^ 2 + (x1z + (-1) .* x3z) .^  ...
  2) .^ (-1 / 2) .* (x1z + (-1) .* x3z) + ((x2x + (-1) .* x4x) .^ 2  ...
  + (x2y + (-1) .* x4y) .^ 2 + (x2z + (-1) .* x4z) .^ 2) .^ (-1 / 2) ...
   .* (x2z + (-1) .* x4z)) + (-1 / 2) .* ((((-1) .* x1y + x3y) .* ( ...
  x2x + (-1) .* x4x) + (x1x + (-1) .* x3x) .* (x2y + (-1) .* x4y))  ...
  .^ 2 + ((x1z + (-1) .* x3z) .* (x2x + (-1) .* x4x) + (-1) .* (x1x  ...
  + (-1) .* x3x) .* (x2z + (-1) .* x4z)) .^ 2 + (((-1) .* x1z + x3z) ...
   .* (x2y + (-1) .* x4y) + (x1y + (-1) .* x3y) .* (x2z + (-1) .*  ...
  x4z)) .^ 2) .^ (-1 / 2) .* (((x1x + (-1) .* x3x) .* ((x1x + (-1)  ...
  .* x3x) .^ 2 + (x1y + (-1) .* x3y) .^ 2 + (x1z + (-1) .* x3z) .^  ...
  2) .^ (-1 / 2) + (x2x + (-1) .* x4x) .* ((x2x + (-1) .* x4x) .^ 2  ...
  + (x2y + (-1) .* x4y) .^ 2 + (x2z + (-1) .* x4z) .^ 2) .^ (-1 / 2) ...
  ) .^ 2 + ((x1y + (-1) .* x3y) .* ((x1x + (-1) .* x3x) .^ 2 + (x1y  ...
  + (-1) .* x3y) .^ 2 + (x1z + (-1) .* x3z) .^ 2) .^ (-1 / 2) + ( ...
  x2y + (-1) .* x4y) .* ((x2x + (-1) .* x4x) .^ 2 + (x2y + (-1) .*  ...
  x4y) .^ 2 + (x2z + (-1) .* x4z) .^ 2) .^ (-1 / 2)) .^ 2 + (((x1x + ...
   (-1) .* x3x) .^ 2 + (x1y + (-1) .* x3y) .^ 2 + (x1z + (-1) .*  ...
  x3z) .^ 2) .^ (-1 / 2) .* (x1z + (-1) .* x3z) + ((x2x + (-1) .*  ...
  x4x) .^ 2 + (x2y + (-1) .* x4y) .^ 2 + (x2z + (-1) .* x4z) .^ 2)  ...
  .^ (-1 / 2) .* (x2z + (-1) .* x4z)) .^ 2) .^ (-3 / 2) .* ((x1z + ( ...
  -1) .* x3z) .* (x2x + (-1) .* x4x) + (-1) .* (x1x + (-1) .* x3x)  ...
  .* (x2z + (-1) .* x4z)) .* (2 .* ((-1) .* (x2x + (-1) .* x4x) .^  ...
  2 .* ((x2x + (-1) .* x4x) .^ 2 + (x2y + (-1) .* x4y) .^ 2 + (x2z + ...
   (-1) .* x4z) .^ 2) .^ (-3 / 2) + ((x2x + (-1) .* x4x) .^ 2 + ( ...
  x2y + (-1) .* x4y) .^ 2 + (x2z + (-1) .* x4z) .^ 2) .^ (-1 / 2))  ...
  .* ((x1x + (-1) .* x3x) .* ((x1x + (-1) .* x3x) .^ 2 + (x1y + (-1) ...
   .* x3y) .^ 2 + (x1z + (-1) .* x3z) .^ 2) .^ (-1 / 2) + (x2x + ( ...
  -1) .* x4x) .* ((x2x + (-1) .* x4x) .^ 2 + (x2y + (-1) .* x4y) .^  ...
  2 + (x2z + (-1) .* x4z) .^ 2) .^ (-1 / 2)) + (-2) .* (x2x + (-1)  ...
  .* x4x) .* (x2y + (-1) .* x4y) .* ((x1y + (-1) .* x3y) .* ((x1x +  ...
  (-1) .* x3x) .^ 2 + (x1y + (-1) .* x3y) .^ 2 + (x1z + (-1) .* x3z) ...
   .^ 2) .^ (-1 / 2) + (x2y + (-1) .* x4y) .* ((x2x + (-1) .* x4x)  ...
  .^ 2 + (x2y + (-1) .* x4y) .^ 2 + (x2z + (-1) .* x4z) .^ 2) .^ ( ...
  -1 / 2)) .* ((x2x + (-1) .* x4x) .^ 2 + (x2y + (-1) .* x4y) .^ 2 + ...
   (x2z + (-1) .* x4z) .^ 2) .^ (-3 / 2) + (-2) .* (x2x + (-1) .*  ...
  x4x) .* (((x1x + (-1) .* x3x) .^ 2 + (x1y + (-1) .* x3y) .^ 2 + ( ...
  x1z + (-1) .* x3z) .^ 2) .^ (-1 / 2) .* (x1z + (-1) .* x3z) + (( ...
  x2x + (-1) .* x4x) .^ 2 + (x2y + (-1) .* x4y) .^ 2 + (x2z + (-1)  ...
  .* x4z) .^ 2) .^ (-1 / 2) .* (x2z + (-1) .* x4z)) .* ((x2x + (-1)  ...
  .* x4x) .^ 2 + (x2y + (-1) .* x4y) .^ 2 + (x2z + (-1) .* x4z) .^  ...
  2) .^ (-3 / 2) .* (x2z + (-1) .* x4z)) .* (((x1x + (-1) .* x3x)  ...
  .^ 2 + (x1y + (-1) .* x3y) .^ 2 + (x1z + (-1) .* x3z) .^ 2) .^ ( ...
  -1 / 2) .* (x1z + (-1) .* x3z) + ((x2x + (-1) .* x4x) .^ 2 + (x2y  ...
  + (-1) .* x4y) .^ 2 + (x2z + (-1) .* x4z) .^ 2) .^ (-1 / 2) .* ( ...
  x2z + (-1) .* x4z)) + (x2x + (-1) .* x4x) .* (((-1) .* x1y + x3y)  ...
  .* (x2x + (-1) .* x4x) + (x1x + (-1) .* x3x) .* (x2y + (-1) .*  ...
  x4y)) .* (x2y + (-1) .* x4y) .* ((((-1) .* x1y + x3y) .* (x2x + ( ...
  -1) .* x4x) + (x1x + (-1) .* x3x) .* (x2y + (-1) .* x4y)) .^ 2 + ( ...
  (x1z + (-1) .* x3z) .* (x2x + (-1) .* x4x) + (-1) .* (x1x + (-1)  ...
  .* x3x) .* (x2z + (-1) .* x4z)) .^ 2 + (((-1) .* x1z + x3z) .* ( ...
  x2y + (-1) .* x4y) + (x1y + (-1) .* x3y) .* (x2z + (-1) .* x4z))  ...
  .^ 2) .^ (-1 / 2) .* (((x1x + (-1) .* x3x) .* ((x1x + (-1) .* x3x) ...
   .^ 2 + (x1y + (-1) .* x3y) .^ 2 + (x1z + (-1) .* x3z) .^ 2) .^ ( ...
  -1 / 2) + (x2x + (-1) .* x4x) .* ((x2x + (-1) .* x4x) .^ 2 + (x2y  ...
  + (-1) .* x4y) .^ 2 + (x2z + (-1) .* x4z) .^ 2) .^ (-1 / 2)) .^ 2  ...
  + ((x1y + (-1) .* x3y) .* ((x1x + (-1) .* x3x) .^ 2 + (x1y + (-1)  ...
  .* x3y) .^ 2 + (x1z + (-1) .* x3z) .^ 2) .^ (-1 / 2) + (x2y + (-1) ...
   .* x4y) .* ((x2x + (-1) .* x4x) .^ 2 + (x2y + (-1) .* x4y) .^ 2 + ...
   (x2z + (-1) .* x4z) .^ 2) .^ (-1 / 2)) .^ 2 + (((x1x + (-1) .*  ...
  x3x) .^ 2 + (x1y + (-1) .* x3y) .^ 2 + (x1z + (-1) .* x3z) .^ 2)  ...
  .^ (-1 / 2) .* (x1z + (-1) .* x3z) + ((x2x + (-1) .* x4x) .^ 2 + ( ...
  x2y + (-1) .* x4y) .^ 2 + (x2z + (-1) .* x4z) .^ 2) .^ (-1 / 2) .* ...
   (x2z + (-1) .* x4z)) .^ 2) .^ (-1 / 2) .* ((x2x + (-1) .* x4x)  ...
  .^ 2 + (x2y + (-1) .* x4y) .^ 2 + (x2z + (-1) .* x4z) .^ 2) .^ ( ...
  -3 / 2) + (-1) .* (x2x + (-1) .* x4x) .* ((((-1) .* x1y + x3y) .*  ...
  (x2x + (-1) .* x4x) + (x1x + (-1) .* x3x) .* (x2y + (-1) .* x4y))  ...
  .^ 2 + ((x1z + (-1) .* x3z) .* (x2x + (-1) .* x4x) + (-1) .* (x1x  ...
  + (-1) .* x3x) .* (x2z + (-1) .* x4z)) .^ 2 + (((-1) .* x1z + x3z) ...
   .* (x2y + (-1) .* x4y) + (x1y + (-1) .* x3y) .* (x2z + (-1) .*  ...
  x4z)) .^ 2) .^ (-1 / 2) .* (((x1x + (-1) .* x3x) .* ((x1x + (-1)  ...
  .* x3x) .^ 2 + (x1y + (-1) .* x3y) .^ 2 + (x1z + (-1) .* x3z) .^  ...
  2) .^ (-1 / 2) + (x2x + (-1) .* x4x) .* ((x2x + (-1) .* x4x) .^ 2  ...
  + (x2y + (-1) .* x4y) .^ 2 + (x2z + (-1) .* x4z) .^ 2) .^ (-1 / 2) ...
  ) .^ 2 + ((x1y + (-1) .* x3y) .* ((x1x + (-1) .* x3x) .^ 2 + (x1y  ...
  + (-1) .* x3y) .^ 2 + (x1z + (-1) .* x3z) .^ 2) .^ (-1 / 2) + ( ...
  x2y + (-1) .* x4y) .* ((x2x + (-1) .* x4x) .^ 2 + (x2y + (-1) .*  ...
  x4y) .^ 2 + (x2z + (-1) .* x4z) .^ 2) .^ (-1 / 2)) .^ 2 + (((x1x + ...
   (-1) .* x3x) .^ 2 + (x1y + (-1) .* x3y) .^ 2 + (x1z + (-1) .*  ...
  x3z) .^ 2) .^ (-1 / 2) .* (x1z + (-1) .* x3z) + ((x2x + (-1) .*  ...
  x4x) .^ 2 + (x2y + (-1) .* x4y) .^ 2 + (x2z + (-1) .* x4z) .^ 2)  ...
  .^ (-1 / 2) .* (x2z + (-1) .* x4z)) .^ 2) .^ (-1 / 2) .* ((x1z + ( ...
  -1) .* x3z) .* (x2x + (-1) .* x4x) + (-1) .* (x1x + (-1) .* x3x)  ...
  .* (x2z + (-1) .* x4z)) .* ((x2x + (-1) .* x4x) .^ 2 + (x2y + (-1) ...
   .* x4y) .^ 2 + (x2z + (-1) .* x4z) .^ 2) .^ (-3 / 2) .* (x2z + ( ...
  -1) .* x4z),(-1) .* (((-1) .* x1y + x3y) .* (x2x + (-1) .* x4x) +  ...
  (x1x + (-1) .* x3x) .* (x2y + (-1) .* x4y)) .* ((((-1) .* x1y +  ...
  x3y) .* (x2x + (-1) .* x4x) + (x1x + (-1) .* x3x) .* (x2y + (-1)  ...
  .* x4y)) .^ 2 + ((x1z + (-1) .* x3z) .* (x2x + (-1) .* x4x) + (-1) ...
   .* (x1x + (-1) .* x3x) .* (x2z + (-1) .* x4z)) .^ 2 + (((-1) .*  ...
  x1z + x3z) .* (x2y + (-1) .* x4y) + (x1y + (-1) .* x3y) .* (x2z +  ...
  (-1) .* x4z)) .^ 2) .^ (-1 / 2) .* (((x1x + (-1) .* x3x) .* ((x1x  ...
  + (-1) .* x3x) .^ 2 + (x1y + (-1) .* x3y) .^ 2 + (x1z + (-1) .*  ...
  x3z) .^ 2) .^ (-1 / 2) + (x2x + (-1) .* x4x) .* ((x2x + (-1) .*  ...
  x4x) .^ 2 + (x2y + (-1) .* x4y) .^ 2 + (x2z + (-1) .* x4z) .^ 2)  ...
  .^ (-1 / 2)) .^ 2 + ((x1y + (-1) .* x3y) .* ((x1x + (-1) .* x3x)  ...
  .^ 2 + (x1y + (-1) .* x3y) .^ 2 + (x1z + (-1) .* x3z) .^ 2) .^ ( ...
  -1 / 2) + (x2y + (-1) .* x4y) .* ((x2x + (-1) .* x4x) .^ 2 + (x2y  ...
  + (-1) .* x4y) .^ 2 + (x2z + (-1) .* x4z) .^ 2) .^ (-1 / 2)) .^ 2  ...
  + (((x1x + (-1) .* x3x) .^ 2 + (x1y + (-1) .* x3y) .^ 2 + (x1z + ( ...
  -1) .* x3z) .^ 2) .^ (-1 / 2) .* (x1z + (-1) .* x3z) + ((x2x + ( ...
  -1) .* x4x) .^ 2 + (x2y + (-1) .* x4y) .^ 2 + (x2z + (-1) .* x4z)  ...
  .^ 2) .^ (-1 / 2) .* (x2z + (-1) .* x4z)) .^ 2) .^ (-1 / 2) .* (( ...
  -1) .* (x2y + (-1) .* x4y) .^ 2 .* ((x2x + (-1) .* x4x) .^ 2 + ( ...
  x2y + (-1) .* x4y) .^ 2 + (x2z + (-1) .* x4z) .^ 2) .^ (-3 / 2) +  ...
  ((x2x + (-1) .* x4x) .^ 2 + (x2y + (-1) .* x4y) .^ 2 + (x2z + (-1) ...
   .* x4z) .^ 2) .^ (-1 / 2)) + (1 / 2) .* (((-1) .* x1y + x3y) .* ( ...
  x2x + (-1) .* x4x) + (x1x + (-1) .* x3x) .* (x2y + (-1) .* x4y))  ...
  .* (2 .* (x1x + (-1) .* x3x) .* (((-1) .* x1y + x3y) .* (x2x + ( ...
  -1) .* x4x) + (x1x + (-1) .* x3x) .* (x2y + (-1) .* x4y)) + 2 .* ( ...
  (-1) .* x1z + x3z) .* (((-1) .* x1z + x3z) .* (x2y + (-1) .* x4y)  ...
  + (x1y + (-1) .* x3y) .* (x2z + (-1) .* x4z))) .* ((((-1) .* x1y + ...
   x3y) .* (x2x + (-1) .* x4x) + (x1x + (-1) .* x3x) .* (x2y + (-1)  ...
  .* x4y)) .^ 2 + ((x1z + (-1) .* x3z) .* (x2x + (-1) .* x4x) + (-1) ...
   .* (x1x + (-1) .* x3x) .* (x2z + (-1) .* x4z)) .^ 2 + (((-1) .*  ...
  x1z + x3z) .* (x2y + (-1) .* x4y) + (x1y + (-1) .* x3y) .* (x2z +  ...
  (-1) .* x4z)) .^ 2) .^ (-3 / 2) .* (((x1x + (-1) .* x3x) .* ((x1x  ...
  + (-1) .* x3x) .^ 2 + (x1y + (-1) .* x3y) .^ 2 + (x1z + (-1) .*  ...
  x3z) .^ 2) .^ (-1 / 2) + (x2x + (-1) .* x4x) .* ((x2x + (-1) .*  ...
  x4x) .^ 2 + (x2y + (-1) .* x4y) .^ 2 + (x2z + (-1) .* x4z) .^ 2)  ...
  .^ (-1 / 2)) .^ 2 + ((x1y + (-1) .* x3y) .* ((x1x + (-1) .* x3x)  ...
  .^ 2 + (x1y + (-1) .* x3y) .^ 2 + (x1z + (-1) .* x3z) .^ 2) .^ ( ...
  -1 / 2) + (x2y + (-1) .* x4y) .* ((x2x + (-1) .* x4x) .^ 2 + (x2y  ...
  + (-1) .* x4y) .^ 2 + (x2z + (-1) .* x4z) .^ 2) .^ (-1 / 2)) .^ 2  ...
  + (((x1x + (-1) .* x3x) .^ 2 + (x1y + (-1) .* x3y) .^ 2 + (x1z + ( ...
  -1) .* x3z) .^ 2) .^ (-1 / 2) .* (x1z + (-1) .* x3z) + ((x2x + ( ...
  -1) .* x4x) .^ 2 + (x2y + (-1) .* x4y) .^ 2 + (x2z + (-1) .* x4z)  ...
  .^ 2) .^ (-1 / 2) .* (x2z + (-1) .* x4z)) .^ 2) .^ (-1 / 2) .* (( ...
  x1y + (-1) .* x3y) .* ((x1x + (-1) .* x3x) .^ 2 + (x1y + (-1) .*  ...
  x3y) .^ 2 + (x1z + (-1) .* x3z) .^ 2) .^ (-1 / 2) + (x2y + (-1) .* ...
   x4y) .* ((x2x + (-1) .* x4x) .^ 2 + (x2y + (-1) .* x4y) .^ 2 + ( ...
  x2z + (-1) .* x4z) .^ 2) .^ (-1 / 2)) + (-1) .* (x1x + (-1) .*  ...
  x3x) .* ((((-1) .* x1y + x3y) .* (x2x + (-1) .* x4x) + (x1x + (-1) ...
   .* x3x) .* (x2y + (-1) .* x4y)) .^ 2 + ((x1z + (-1) .* x3z) .* ( ...
  x2x + (-1) .* x4x) + (-1) .* (x1x + (-1) .* x3x) .* (x2z + (-1) .* ...
   x4z)) .^ 2 + (((-1) .* x1z + x3z) .* (x2y + (-1) .* x4y) + (x1y + ...
   (-1) .* x3y) .* (x2z + (-1) .* x4z)) .^ 2) .^ (-1 / 2) .* (((x1x  ...
  + (-1) .* x3x) .* ((x1x + (-1) .* x3x) .^ 2 + (x1y + (-1) .* x3y)  ...
  .^ 2 + (x1z + (-1) .* x3z) .^ 2) .^ (-1 / 2) + (x2x + (-1) .* x4x) ...
   .* ((x2x + (-1) .* x4x) .^ 2 + (x2y + (-1) .* x4y) .^ 2 + (x2z +  ...
  (-1) .* x4z) .^ 2) .^ (-1 / 2)) .^ 2 + ((x1y + (-1) .* x3y) .* (( ...
  x1x + (-1) .* x3x) .^ 2 + (x1y + (-1) .* x3y) .^ 2 + (x1z + (-1)  ...
  .* x3z) .^ 2) .^ (-1 / 2) + (x2y + (-1) .* x4y) .* ((x2x + (-1) .* ...
   x4x) .^ 2 + (x2y + (-1) .* x4y) .^ 2 + (x2z + (-1) .* x4z) .^ 2)  ...
  .^ (-1 / 2)) .^ 2 + (((x1x + (-1) .* x3x) .^ 2 + (x1y + (-1) .*  ...
  x3y) .^ 2 + (x1z + (-1) .* x3z) .^ 2) .^ (-1 / 2) .* (x1z + (-1)  ...
  .* x3z) + ((x2x + (-1) .* x4x) .^ 2 + (x2y + (-1) .* x4y) .^ 2 + ( ...
  x2z + (-1) .* x4z) .^ 2) .^ (-1 / 2) .* (x2z + (-1) .* x4z)) .^ 2) ...
   .^ (-1 / 2) .* ((x1y + (-1) .* x3y) .* ((x1x + (-1) .* x3x) .^ 2  ...
  + (x1y + (-1) .* x3y) .^ 2 + (x1z + (-1) .* x3z) .^ 2) .^ (-1 / 2) ...
   + (x2y + (-1) .* x4y) .* ((x2x + (-1) .* x4x) .^ 2 + (x2y + (-1)  ...
  .* x4y) .^ 2 + (x2z + (-1) .* x4z) .^ 2) .^ (-1 / 2)) + (1 / 2) .* ...
   (((-1) .* x1y + x3y) .* (x2x + (-1) .* x4x) + (x1x + (-1) .* x3x) ...
   .* (x2y + (-1) .* x4y)) .* ((((-1) .* x1y + x3y) .* (x2x + (-1)  ...
  .* x4x) + (x1x + (-1) .* x3x) .* (x2y + (-1) .* x4y)) .^ 2 + (( ...
  x1z + (-1) .* x3z) .* (x2x + (-1) .* x4x) + (-1) .* (x1x + (-1) .* ...
   x3x) .* (x2z + (-1) .* x4z)) .^ 2 + (((-1) .* x1z + x3z) .* (x2y  ...
  + (-1) .* x4y) + (x1y + (-1) .* x3y) .* (x2z + (-1) .* x4z)) .^ 2) ...
   .^ (-1 / 2) .* (((x1x + (-1) .* x3x) .* ((x1x + (-1) .* x3x) .^  ...
  2 + (x1y + (-1) .* x3y) .^ 2 + (x1z + (-1) .* x3z) .^ 2) .^ (-1 /  ...
  2) + (x2x + (-1) .* x4x) .* ((x2x + (-1) .* x4x) .^ 2 + (x2y + ( ...
  -1) .* x4y) .^ 2 + (x2z + (-1) .* x4z) .^ 2) .^ (-1 / 2)) .^ 2 + ( ...
  (x1y + (-1) .* x3y) .* ((x1x + (-1) .* x3x) .^ 2 + (x1y + (-1) .*  ...
  x3y) .^ 2 + (x1z + (-1) .* x3z) .^ 2) .^ (-1 / 2) + (x2y + (-1) .* ...
   x4y) .* ((x2x + (-1) .* x4x) .^ 2 + (x2y + (-1) .* x4y) .^ 2 + ( ...
  x2z + (-1) .* x4z) .^ 2) .^ (-1 / 2)) .^ 2 + (((x1x + (-1) .* x3x) ...
   .^ 2 + (x1y + (-1) .* x3y) .^ 2 + (x1z + (-1) .* x3z) .^ 2) .^ ( ...
  -1 / 2) .* (x1z + (-1) .* x3z) + ((x2x + (-1) .* x4x) .^ 2 + (x2y  ...
  + (-1) .* x4y) .^ 2 + (x2z + (-1) .* x4z) .^ 2) .^ (-1 / 2) .* ( ...
  x2z + (-1) .* x4z)) .^ 2) .^ (-3 / 2) .* ((x1y + (-1) .* x3y) .* ( ...
  (x1x + (-1) .* x3x) .^ 2 + (x1y + (-1) .* x3y) .^ 2 + (x1z + (-1)  ...
  .* x3z) .^ 2) .^ (-1 / 2) + (x2y + (-1) .* x4y) .* ((x2x + (-1) .* ...
   x4x) .^ 2 + (x2y + (-1) .* x4y) .^ 2 + (x2z + (-1) .* x4z) .^ 2)  ...
  .^ (-1 / 2)) .* (2 .* ((-1) .* (x2y + (-1) .* x4y) .^ 2 .* ((x2x + ...
   (-1) .* x4x) .^ 2 + (x2y + (-1) .* x4y) .^ 2 + (x2z + (-1) .*  ...
  x4z) .^ 2) .^ (-3 / 2) + ((x2x + (-1) .* x4x) .^ 2 + (x2y + (-1)  ...
  .* x4y) .^ 2 + (x2z + (-1) .* x4z) .^ 2) .^ (-1 / 2)) .* ((x1y + ( ...
  -1) .* x3y) .* ((x1x + (-1) .* x3x) .^ 2 + (x1y + (-1) .* x3y) .^  ...
  2 + (x1z + (-1) .* x3z) .^ 2) .^ (-1 / 2) + (x2y + (-1) .* x4y) .* ...
   ((x2x + (-1) .* x4x) .^ 2 + (x2y + (-1) .* x4y) .^ 2 + (x2z + ( ...
  -1) .* x4z) .^ 2) .^ (-1 / 2)) + (-2) .* (x2x + (-1) .* x4x) .* ( ...
  x2y + (-1) .* x4y) .* ((x1x + (-1) .* x3x) .* ((x1x + (-1) .* x3x) ...
   .^ 2 + (x1y + (-1) .* x3y) .^ 2 + (x1z + (-1) .* x3z) .^ 2) .^ ( ...
  -1 / 2) + (x2x + (-1) .* x4x) .* ((x2x + (-1) .* x4x) .^ 2 + (x2y  ...
  + (-1) .* x4y) .^ 2 + (x2z + (-1) .* x4z) .^ 2) .^ (-1 / 2)) .* (( ...
  x2x + (-1) .* x4x) .^ 2 + (x2y + (-1) .* x4y) .^ 2 + (x2z + (-1)  ...
  .* x4z) .^ 2) .^ (-3 / 2) + (-2) .* (x2y + (-1) .* x4y) .* (((x1x  ...
  + (-1) .* x3x) .^ 2 + (x1y + (-1) .* x3y) .^ 2 + (x1z + (-1) .*  ...
  x3z) .^ 2) .^ (-1 / 2) .* (x1z + (-1) .* x3z) + ((x2x + (-1) .*  ...
  x4x) .^ 2 + (x2y + (-1) .* x4y) .^ 2 + (x2z + (-1) .* x4z) .^ 2)  ...
  .^ (-1 / 2) .* (x2z + (-1) .* x4z)) .* ((x2x + (-1) .* x4x) .^ 2 + ...
   (x2y + (-1) .* x4y) .^ 2 + (x2z + (-1) .* x4z) .^ 2) .^ (-3 / 2)  ...
  .* (x2z + (-1) .* x4z)) + (-1 / 2) .* (2 .* (x1x + (-1) .* x3x) .* ...
   (((-1) .* x1y + x3y) .* (x2x + (-1) .* x4x) + (x1x + (-1) .* x3x) ...
   .* (x2y + (-1) .* x4y)) + 2 .* ((-1) .* x1z + x3z) .* (((-1) .*  ...
  x1z + x3z) .* (x2y + (-1) .* x4y) + (x1y + (-1) .* x3y) .* (x2z +  ...
  (-1) .* x4z))) .* ((((-1) .* x1y + x3y) .* (x2x + (-1) .* x4x) + ( ...
  x1x + (-1) .* x3x) .* (x2y + (-1) .* x4y)) .^ 2 + ((x1z + (-1) .*  ...
  x3z) .* (x2x + (-1) .* x4x) + (-1) .* (x1x + (-1) .* x3x) .* (x2z  ...
  + (-1) .* x4z)) .^ 2 + (((-1) .* x1z + x3z) .* (x2y + (-1) .* x4y) ...
   + (x1y + (-1) .* x3y) .* (x2z + (-1) .* x4z)) .^ 2) .^ (-3 / 2)  ...
  .* (((x1x + (-1) .* x3x) .* ((x1x + (-1) .* x3x) .^ 2 + (x1y + ( ...
  -1) .* x3y) .^ 2 + (x1z + (-1) .* x3z) .^ 2) .^ (-1 / 2) + (x2x +  ...
  (-1) .* x4x) .* ((x2x + (-1) .* x4x) .^ 2 + (x2y + (-1) .* x4y)  ...
  .^ 2 + (x2z + (-1) .* x4z) .^ 2) .^ (-1 / 2)) .^ 2 + ((x1y + (-1)  ...
  .* x3y) .* ((x1x + (-1) .* x3x) .^ 2 + (x1y + (-1) .* x3y) .^ 2 +  ...
  (x1z + (-1) .* x3z) .^ 2) .^ (-1 / 2) + (x2y + (-1) .* x4y) .* (( ...
  x2x + (-1) .* x4x) .^ 2 + (x2y + (-1) .* x4y) .^ 2 + (x2z + (-1)  ...
  .* x4z) .^ 2) .^ (-1 / 2)) .^ 2 + (((x1x + (-1) .* x3x) .^ 2 + ( ...
  x1y + (-1) .* x3y) .^ 2 + (x1z + (-1) .* x3z) .^ 2) .^ (-1 / 2) .* ...
   (x1z + (-1) .* x3z) + ((x2x + (-1) .* x4x) .^ 2 + (x2y + (-1) .*  ...
  x4y) .^ 2 + (x2z + (-1) .* x4z) .^ 2) .^ (-1 / 2) .* (x2z + (-1)  ...
  .* x4z)) .^ 2) .^ (-1 / 2) .* ((x1z + (-1) .* x3z) .* (x2x + (-1)  ...
  .* x4x) + (-1) .* (x1x + (-1) .* x3x) .* (x2z + (-1) .* x4z)) .* ( ...
  ((x1x + (-1) .* x3x) .^ 2 + (x1y + (-1) .* x3y) .^ 2 + (x1z + (-1) ...
   .* x3z) .^ 2) .^ (-1 / 2) .* (x1z + (-1) .* x3z) + ((x2x + (-1)  ...
  .* x4x) .^ 2 + (x2y + (-1) .* x4y) .^ 2 + (x2z + (-1) .* x4z) .^  ...
  2) .^ (-1 / 2) .* (x2z + (-1) .* x4z)) + (-1 / 2) .* ((((-1) .*  ...
  x1y + x3y) .* (x2x + (-1) .* x4x) + (x1x + (-1) .* x3x) .* (x2y +  ...
  (-1) .* x4y)) .^ 2 + ((x1z + (-1) .* x3z) .* (x2x + (-1) .* x4x) + ...
   (-1) .* (x1x + (-1) .* x3x) .* (x2z + (-1) .* x4z)) .^ 2 + (((-1) ...
   .* x1z + x3z) .* (x2y + (-1) .* x4y) + (x1y + (-1) .* x3y) .* ( ...
  x2z + (-1) .* x4z)) .^ 2) .^ (-1 / 2) .* (((x1x + (-1) .* x3x) .*  ...
  ((x1x + (-1) .* x3x) .^ 2 + (x1y + (-1) .* x3y) .^ 2 + (x1z + (-1) ...
   .* x3z) .^ 2) .^ (-1 / 2) + (x2x + (-1) .* x4x) .* ((x2x + (-1)  ...
  .* x4x) .^ 2 + (x2y + (-1) .* x4y) .^ 2 + (x2z + (-1) .* x4z) .^  ...
  2) .^ (-1 / 2)) .^ 2 + ((x1y + (-1) .* x3y) .* ((x1x + (-1) .*  ...
  x3x) .^ 2 + (x1y + (-1) .* x3y) .^ 2 + (x1z + (-1) .* x3z) .^ 2)  ...
  .^ (-1 / 2) + (x2y + (-1) .* x4y) .* ((x2x + (-1) .* x4x) .^ 2 + ( ...
  x2y + (-1) .* x4y) .^ 2 + (x2z + (-1) .* x4z) .^ 2) .^ (-1 / 2))  ...
  .^ 2 + (((x1x + (-1) .* x3x) .^ 2 + (x1y + (-1) .* x3y) .^ 2 + ( ...
  x1z + (-1) .* x3z) .^ 2) .^ (-1 / 2) .* (x1z + (-1) .* x3z) + (( ...
  x2x + (-1) .* x4x) .^ 2 + (x2y + (-1) .* x4y) .^ 2 + (x2z + (-1)  ...
  .* x4z) .^ 2) .^ (-1 / 2) .* (x2z + (-1) .* x4z)) .^ 2) .^ (-3 /  ...
  2) .* ((x1z + (-1) .* x3z) .* (x2x + (-1) .* x4x) + (-1) .* (x1x + ...
   (-1) .* x3x) .* (x2z + (-1) .* x4z)) .* (2 .* ((-1) .* (x2y + ( ...
  -1) .* x4y) .^ 2 .* ((x2x + (-1) .* x4x) .^ 2 + (x2y + (-1) .*  ...
  x4y) .^ 2 + (x2z + (-1) .* x4z) .^ 2) .^ (-3 / 2) + ((x2x + (-1)  ...
  .* x4x) .^ 2 + (x2y + (-1) .* x4y) .^ 2 + (x2z + (-1) .* x4z) .^  ...
  2) .^ (-1 / 2)) .* ((x1y + (-1) .* x3y) .* ((x1x + (-1) .* x3x)  ...
  .^ 2 + (x1y + (-1) .* x3y) .^ 2 + (x1z + (-1) .* x3z) .^ 2) .^ ( ...
  -1 / 2) + (x2y + (-1) .* x4y) .* ((x2x + (-1) .* x4x) .^ 2 + (x2y  ...
  + (-1) .* x4y) .^ 2 + (x2z + (-1) .* x4z) .^ 2) .^ (-1 / 2)) + ( ...
  -2) .* (x2x + (-1) .* x4x) .* (x2y + (-1) .* x4y) .* ((x1x + (-1)  ...
  .* x3x) .* ((x1x + (-1) .* x3x) .^ 2 + (x1y + (-1) .* x3y) .^ 2 +  ...
  (x1z + (-1) .* x3z) .^ 2) .^ (-1 / 2) + (x2x + (-1) .* x4x) .* (( ...
  x2x + (-1) .* x4x) .^ 2 + (x2y + (-1) .* x4y) .^ 2 + (x2z + (-1)  ...
  .* x4z) .^ 2) .^ (-1 / 2)) .* ((x2x + (-1) .* x4x) .^ 2 + (x2y + ( ...
  -1) .* x4y) .^ 2 + (x2z + (-1) .* x4z) .^ 2) .^ (-3 / 2) + (-2) .* ...
   (x2y + (-1) .* x4y) .* (((x1x + (-1) .* x3x) .^ 2 + (x1y + (-1)  ...
  .* x3y) .^ 2 + (x1z + (-1) .* x3z) .^ 2) .^ (-1 / 2) .* (x1z + ( ...
  -1) .* x3z) + ((x2x + (-1) .* x4x) .^ 2 + (x2y + (-1) .* x4y) .^  ...
  2 + (x2z + (-1) .* x4z) .^ 2) .^ (-1 / 2) .* (x2z + (-1) .* x4z))  ...
  .* ((x2x + (-1) .* x4x) .^ 2 + (x2y + (-1) .* x4y) .^ 2 + (x2z + ( ...
  -1) .* x4z) .^ 2) .^ (-3 / 2) .* (x2z + (-1) .* x4z)) .* (((x1x +  ...
  (-1) .* x3x) .^ 2 + (x1y + (-1) .* x3y) .^ 2 + (x1z + (-1) .* x3z) ...
   .^ 2) .^ (-1 / 2) .* (x1z + (-1) .* x3z) + ((x2x + (-1) .* x4x)  ...
  .^ 2 + (x2y + (-1) .* x4y) .^ 2 + (x2z + (-1) .* x4z) .^ 2) .^ ( ...
  -1 / 2) .* (x2z + (-1) .* x4z)) + (-1) .* (x2y + (-1) .* x4y) .* ( ...
  (((-1) .* x1y + x3y) .* (x2x + (-1) .* x4x) + (x1x + (-1) .* x3x)  ...
  .* (x2y + (-1) .* x4y)) .^ 2 + ((x1z + (-1) .* x3z) .* (x2x + (-1) ...
   .* x4x) + (-1) .* (x1x + (-1) .* x3x) .* (x2z + (-1) .* x4z)) .^  ...
  2 + (((-1) .* x1z + x3z) .* (x2y + (-1) .* x4y) + (x1y + (-1) .*  ...
  x3y) .* (x2z + (-1) .* x4z)) .^ 2) .^ (-1 / 2) .* (((x1x + (-1) .* ...
   x3x) .* ((x1x + (-1) .* x3x) .^ 2 + (x1y + (-1) .* x3y) .^ 2 + ( ...
  x1z + (-1) .* x3z) .^ 2) .^ (-1 / 2) + (x2x + (-1) .* x4x) .* (( ...
  x2x + (-1) .* x4x) .^ 2 + (x2y + (-1) .* x4y) .^ 2 + (x2z + (-1)  ...
  .* x4z) .^ 2) .^ (-1 / 2)) .^ 2 + ((x1y + (-1) .* x3y) .* ((x1x +  ...
  (-1) .* x3x) .^ 2 + (x1y + (-1) .* x3y) .^ 2 + (x1z + (-1) .* x3z) ...
   .^ 2) .^ (-1 / 2) + (x2y + (-1) .* x4y) .* ((x2x + (-1) .* x4x)  ...
  .^ 2 + (x2y + (-1) .* x4y) .^ 2 + (x2z + (-1) .* x4z) .^ 2) .^ ( ...
  -1 / 2)) .^ 2 + (((x1x + (-1) .* x3x) .^ 2 + (x1y + (-1) .* x3y)  ...
  .^ 2 + (x1z + (-1) .* x3z) .^ 2) .^ (-1 / 2) .* (x1z + (-1) .*  ...
  x3z) + ((x2x + (-1) .* x4x) .^ 2 + (x2y + (-1) .* x4y) .^ 2 + ( ...
  x2z + (-1) .* x4z) .^ 2) .^ (-1 / 2) .* (x2z + (-1) .* x4z)) .^ 2) ...
   .^ (-1 / 2) .* ((x1z + (-1) .* x3z) .* (x2x + (-1) .* x4x) + (-1) ...
   .* (x1x + (-1) .* x3x) .* (x2z + (-1) .* x4z)) .* ((x2x + (-1) .* ...
   x4x) .^ 2 + (x2y + (-1) .* x4y) .^ 2 + (x2z + (-1) .* x4z) .^ 2)  ...
  .^ (-3 / 2) .* (x2z + (-1) .* x4z),(1 / 2) .* (((-1) .* x1y + x3y) ...
   .* (x2x + (-1) .* x4x) + (x1x + (-1) .* x3x) .* (x2y + (-1) .*  ...
  x4y)) .* (2 .* ((-1) .* x1x + x3x) .* ((x1z + (-1) .* x3z) .* ( ...
  x2x + (-1) .* x4x) + (-1) .* (x1x + (-1) .* x3x) .* (x2z + (-1) .* ...
   x4z)) + 2 .* (x1y + (-1) .* x3y) .* (((-1) .* x1z + x3z) .* (x2y  ...
  + (-1) .* x4y) + (x1y + (-1) .* x3y) .* (x2z + (-1) .* x4z))) .* ( ...
  (((-1) .* x1y + x3y) .* (x2x + (-1) .* x4x) + (x1x + (-1) .* x3x)  ...
  .* (x2y + (-1) .* x4y)) .^ 2 + ((x1z + (-1) .* x3z) .* (x2x + (-1) ...
   .* x4x) + (-1) .* (x1x + (-1) .* x3x) .* (x2z + (-1) .* x4z)) .^  ...
  2 + (((-1) .* x1z + x3z) .* (x2y + (-1) .* x4y) + (x1y + (-1) .*  ...
  x3y) .* (x2z + (-1) .* x4z)) .^ 2) .^ (-3 / 2) .* (((x1x + (-1) .* ...
   x3x) .* ((x1x + (-1) .* x3x) .^ 2 + (x1y + (-1) .* x3y) .^ 2 + ( ...
  x1z + (-1) .* x3z) .^ 2) .^ (-1 / 2) + (x2x + (-1) .* x4x) .* (( ...
  x2x + (-1) .* x4x) .^ 2 + (x2y + (-1) .* x4y) .^ 2 + (x2z + (-1)  ...
  .* x4z) .^ 2) .^ (-1 / 2)) .^ 2 + ((x1y + (-1) .* x3y) .* ((x1x +  ...
  (-1) .* x3x) .^ 2 + (x1y + (-1) .* x3y) .^ 2 + (x1z + (-1) .* x3z) ...
   .^ 2) .^ (-1 / 2) + (x2y + (-1) .* x4y) .* ((x2x + (-1) .* x4x)  ...
  .^ 2 + (x2y + (-1) .* x4y) .^ 2 + (x2z + (-1) .* x4z) .^ 2) .^ ( ...
  -1 / 2)) .^ 2 + (((x1x + (-1) .* x3x) .^ 2 + (x1y + (-1) .* x3y)  ...
  .^ 2 + (x1z + (-1) .* x3z) .^ 2) .^ (-1 / 2) .* (x1z + (-1) .*  ...
  x3z) + ((x2x + (-1) .* x4x) .^ 2 + (x2y + (-1) .* x4y) .^ 2 + ( ...
  x2z + (-1) .* x4z) .^ 2) .^ (-1 / 2) .* (x2z + (-1) .* x4z)) .^ 2) ...
   .^ (-1 / 2) .* ((x1y + (-1) .* x3y) .* ((x1x + (-1) .* x3x) .^ 2  ...
  + (x1y + (-1) .* x3y) .^ 2 + (x1z + (-1) .* x3z) .^ 2) .^ (-1 / 2) ...
   + (x2y + (-1) .* x4y) .* ((x2x + (-1) .* x4x) .^ 2 + (x2y + (-1)  ...
  .* x4y) .^ 2 + (x2z + (-1) .* x4z) .^ 2) .^ (-1 / 2)) + (1 / 2) .* ...
   (((-1) .* x1y + x3y) .* (x2x + (-1) .* x4x) + (x1x + (-1) .* x3x) ...
   .* (x2y + (-1) .* x4y)) .* ((((-1) .* x1y + x3y) .* (x2x + (-1)  ...
  .* x4x) + (x1x + (-1) .* x3x) .* (x2y + (-1) .* x4y)) .^ 2 + (( ...
  x1z + (-1) .* x3z) .* (x2x + (-1) .* x4x) + (-1) .* (x1x + (-1) .* ...
   x3x) .* (x2z + (-1) .* x4z)) .^ 2 + (((-1) .* x1z + x3z) .* (x2y  ...
  + (-1) .* x4y) + (x1y + (-1) .* x3y) .* (x2z + (-1) .* x4z)) .^ 2) ...
   .^ (-1 / 2) .* (((x1x + (-1) .* x3x) .* ((x1x + (-1) .* x3x) .^  ...
  2 + (x1y + (-1) .* x3y) .^ 2 + (x1z + (-1) .* x3z) .^ 2) .^ (-1 /  ...
  2) + (x2x + (-1) .* x4x) .* ((x2x + (-1) .* x4x) .^ 2 + (x2y + ( ...
  -1) .* x4y) .^ 2 + (x2z + (-1) .* x4z) .^ 2) .^ (-1 / 2)) .^ 2 + ( ...
  (x1y + (-1) .* x3y) .* ((x1x + (-1) .* x3x) .^ 2 + (x1y + (-1) .*  ...
  x3y) .^ 2 + (x1z + (-1) .* x3z) .^ 2) .^ (-1 / 2) + (x2y + (-1) .* ...
   x4y) .* ((x2x + (-1) .* x4x) .^ 2 + (x2y + (-1) .* x4y) .^ 2 + ( ...
  x2z + (-1) .* x4z) .^ 2) .^ (-1 / 2)) .^ 2 + (((x1x + (-1) .* x3x) ...
   .^ 2 + (x1y + (-1) .* x3y) .^ 2 + (x1z + (-1) .* x3z) .^ 2) .^ ( ...
  -1 / 2) .* (x1z + (-1) .* x3z) + ((x2x + (-1) .* x4x) .^ 2 + (x2y  ...
  + (-1) .* x4y) .^ 2 + (x2z + (-1) .* x4z) .^ 2) .^ (-1 / 2) .* ( ...
  x2z + (-1) .* x4z)) .^ 2) .^ (-3 / 2) .* ((x1y + (-1) .* x3y) .* ( ...
  (x1x + (-1) .* x3x) .^ 2 + (x1y + (-1) .* x3y) .^ 2 + (x1z + (-1)  ...
  .* x3z) .^ 2) .^ (-1 / 2) + (x2y + (-1) .* x4y) .* ((x2x + (-1) .* ...
   x4x) .^ 2 + (x2y + (-1) .* x4y) .^ 2 + (x2z + (-1) .* x4z) .^ 2)  ...
  .^ (-1 / 2)) .* (2 .* (((x1x + (-1) .* x3x) .^ 2 + (x1y + (-1) .*  ...
  x3y) .^ 2 + (x1z + (-1) .* x3z) .^ 2) .^ (-1 / 2) .* (x1z + (-1)  ...
  .* x3z) + ((x2x + (-1) .* x4x) .^ 2 + (x2y + (-1) .* x4y) .^ 2 + ( ...
  x2z + (-1) .* x4z) .^ 2) .^ (-1 / 2) .* (x2z + (-1) .* x4z)) .* (( ...
  (x2x + (-1) .* x4x) .^ 2 + (x2y + (-1) .* x4y) .^ 2 + (x2z + (-1)  ...
  .* x4z) .^ 2) .^ (-1 / 2) + (-1) .* ((x2x + (-1) .* x4x) .^ 2 + ( ...
  x2y + (-1) .* x4y) .^ 2 + (x2z + (-1) .* x4z) .^ 2) .^ (-3 / 2) .* ...
   (x2z + (-1) .* x4z) .^ 2) + (-2) .* (x2x + (-1) .* x4x) .* ((x1x  ...
  + (-1) .* x3x) .* ((x1x + (-1) .* x3x) .^ 2 + (x1y + (-1) .* x3y)  ...
  .^ 2 + (x1z + (-1) .* x3z) .^ 2) .^ (-1 / 2) + (x2x + (-1) .* x4x) ...
   .* ((x2x + (-1) .* x4x) .^ 2 + (x2y + (-1) .* x4y) .^ 2 + (x2z +  ...
  (-1) .* x4z) .^ 2) .^ (-1 / 2)) .* ((x2x + (-1) .* x4x) .^ 2 + ( ...
  x2y + (-1) .* x4y) .^ 2 + (x2z + (-1) .* x4z) .^ 2) .^ (-3 / 2) .* ...
   (x2z + (-1) .* x4z) + (-2) .* (x2y + (-1) .* x4y) .* ((x1y + (-1) ...
   .* x3y) .* ((x1x + (-1) .* x3x) .^ 2 + (x1y + (-1) .* x3y) .^ 2 + ...
   (x1z + (-1) .* x3z) .^ 2) .^ (-1 / 2) + (x2y + (-1) .* x4y) .* (( ...
  x2x + (-1) .* x4x) .^ 2 + (x2y + (-1) .* x4y) .^ 2 + (x2z + (-1)  ...
  .* x4z) .^ 2) .^ (-1 / 2)) .* ((x2x + (-1) .* x4x) .^ 2 + (x2y + ( ...
  -1) .* x4y) .^ 2 + (x2z + (-1) .* x4z) .^ 2) .^ (-3 / 2) .* (x2z + ...
   (-1) .* x4z)) + ((-1) .* x1x + x3x) .* ((((-1) .* x1y + x3y) .* ( ...
  x2x + (-1) .* x4x) + (x1x + (-1) .* x3x) .* (x2y + (-1) .* x4y))  ...
  .^ 2 + ((x1z + (-1) .* x3z) .* (x2x + (-1) .* x4x) + (-1) .* (x1x  ...
  + (-1) .* x3x) .* (x2z + (-1) .* x4z)) .^ 2 + (((-1) .* x1z + x3z) ...
   .* (x2y + (-1) .* x4y) + (x1y + (-1) .* x3y) .* (x2z + (-1) .*  ...
  x4z)) .^ 2) .^ (-1 / 2) .* (((x1x + (-1) .* x3x) .* ((x1x + (-1)  ...
  .* x3x) .^ 2 + (x1y + (-1) .* x3y) .^ 2 + (x1z + (-1) .* x3z) .^  ...
  2) .^ (-1 / 2) + (x2x + (-1) .* x4x) .* ((x2x + (-1) .* x4x) .^ 2  ...
  + (x2y + (-1) .* x4y) .^ 2 + (x2z + (-1) .* x4z) .^ 2) .^ (-1 / 2) ...
  ) .^ 2 + ((x1y + (-1) .* x3y) .* ((x1x + (-1) .* x3x) .^ 2 + (x1y  ...
  + (-1) .* x3y) .^ 2 + (x1z + (-1) .* x3z) .^ 2) .^ (-1 / 2) + ( ...
  x2y + (-1) .* x4y) .* ((x2x + (-1) .* x4x) .^ 2 + (x2y + (-1) .*  ...
  x4y) .^ 2 + (x2z + (-1) .* x4z) .^ 2) .^ (-1 / 2)) .^ 2 + (((x1x + ...
   (-1) .* x3x) .^ 2 + (x1y + (-1) .* x3y) .^ 2 + (x1z + (-1) .*  ...
  x3z) .^ 2) .^ (-1 / 2) .* (x1z + (-1) .* x3z) + ((x2x + (-1) .*  ...
  x4x) .^ 2 + (x2y + (-1) .* x4y) .^ 2 + (x2z + (-1) .* x4z) .^ 2)  ...
  .^ (-1 / 2) .* (x2z + (-1) .* x4z)) .^ 2) .^ (-1 / 2) .* (((x1x +  ...
  (-1) .* x3x) .^ 2 + (x1y + (-1) .* x3y) .^ 2 + (x1z + (-1) .* x3z) ...
   .^ 2) .^ (-1 / 2) .* (x1z + (-1) .* x3z) + ((x2x + (-1) .* x4x)  ...
  .^ 2 + (x2y + (-1) .* x4y) .^ 2 + (x2z + (-1) .* x4z) .^ 2) .^ ( ...
  -1 / 2) .* (x2z + (-1) .* x4z)) + (-1 / 2) .* (2 .* ((-1) .* x1x + ...
   x3x) .* ((x1z + (-1) .* x3z) .* (x2x + (-1) .* x4x) + (-1) .* ( ...
  x1x + (-1) .* x3x) .* (x2z + (-1) .* x4z)) + 2 .* (x1y + (-1) .*  ...
  x3y) .* (((-1) .* x1z + x3z) .* (x2y + (-1) .* x4y) + (x1y + (-1)  ...
  .* x3y) .* (x2z + (-1) .* x4z))) .* ((((-1) .* x1y + x3y) .* (x2x  ...
  + (-1) .* x4x) + (x1x + (-1) .* x3x) .* (x2y + (-1) .* x4y)) .^ 2  ...
  + ((x1z + (-1) .* x3z) .* (x2x + (-1) .* x4x) + (-1) .* (x1x + ( ...
  -1) .* x3x) .* (x2z + (-1) .* x4z)) .^ 2 + (((-1) .* x1z + x3z) .* ...
   (x2y + (-1) .* x4y) + (x1y + (-1) .* x3y) .* (x2z + (-1) .* x4z)) ...
   .^ 2) .^ (-3 / 2) .* (((x1x + (-1) .* x3x) .* ((x1x + (-1) .*  ...
  x3x) .^ 2 + (x1y + (-1) .* x3y) .^ 2 + (x1z + (-1) .* x3z) .^ 2)  ...
  .^ (-1 / 2) + (x2x + (-1) .* x4x) .* ((x2x + (-1) .* x4x) .^ 2 + ( ...
  x2y + (-1) .* x4y) .^ 2 + (x2z + (-1) .* x4z) .^ 2) .^ (-1 / 2))  ...
  .^ 2 + ((x1y + (-1) .* x3y) .* ((x1x + (-1) .* x3x) .^ 2 + (x1y +  ...
  (-1) .* x3y) .^ 2 + (x1z + (-1) .* x3z) .^ 2) .^ (-1 / 2) + (x2y + ...
   (-1) .* x4y) .* ((x2x + (-1) .* x4x) .^ 2 + (x2y + (-1) .* x4y)  ...
  .^ 2 + (x2z + (-1) .* x4z) .^ 2) .^ (-1 / 2)) .^ 2 + (((x1x + (-1) ...
   .* x3x) .^ 2 + (x1y + (-1) .* x3y) .^ 2 + (x1z + (-1) .* x3z) .^  ...
  2) .^ (-1 / 2) .* (x1z + (-1) .* x3z) + ((x2x + (-1) .* x4x) .^ 2  ...
  + (x2y + (-1) .* x4y) .^ 2 + (x2z + (-1) .* x4z) .^ 2) .^ (-1 / 2) ...
   .* (x2z + (-1) .* x4z)) .^ 2) .^ (-1 / 2) .* ((x1z + (-1) .* x3z) ...
   .* (x2x + (-1) .* x4x) + (-1) .* (x1x + (-1) .* x3x) .* (x2z + ( ...
  -1) .* x4z)) .* (((x1x + (-1) .* x3x) .^ 2 + (x1y + (-1) .* x3y)  ...
  .^ 2 + (x1z + (-1) .* x3z) .^ 2) .^ (-1 / 2) .* (x1z + (-1) .*  ...
  x3z) + ((x2x + (-1) .* x4x) .^ 2 + (x2y + (-1) .* x4y) .^ 2 + ( ...
  x2z + (-1) .* x4z) .^ 2) .^ (-1 / 2) .* (x2z + (-1) .* x4z)) + ( ...
  -1 / 2) .* ((((-1) .* x1y + x3y) .* (x2x + (-1) .* x4x) + (x1x + ( ...
  -1) .* x3x) .* (x2y + (-1) .* x4y)) .^ 2 + ((x1z + (-1) .* x3z) .* ...
   (x2x + (-1) .* x4x) + (-1) .* (x1x + (-1) .* x3x) .* (x2z + (-1)  ...
  .* x4z)) .^ 2 + (((-1) .* x1z + x3z) .* (x2y + (-1) .* x4y) + ( ...
  x1y + (-1) .* x3y) .* (x2z + (-1) .* x4z)) .^ 2) .^ (-1 / 2) .* (( ...
  (x1x + (-1) .* x3x) .* ((x1x + (-1) .* x3x) .^ 2 + (x1y + (-1) .*  ...
  x3y) .^ 2 + (x1z + (-1) .* x3z) .^ 2) .^ (-1 / 2) + (x2x + (-1) .* ...
   x4x) .* ((x2x + (-1) .* x4x) .^ 2 + (x2y + (-1) .* x4y) .^ 2 + ( ...
  x2z + (-1) .* x4z) .^ 2) .^ (-1 / 2)) .^ 2 + ((x1y + (-1) .* x3y)  ...
  .* ((x1x + (-1) .* x3x) .^ 2 + (x1y + (-1) .* x3y) .^ 2 + (x1z + ( ...
  -1) .* x3z) .^ 2) .^ (-1 / 2) + (x2y + (-1) .* x4y) .* ((x2x + ( ...
  -1) .* x4x) .^ 2 + (x2y + (-1) .* x4y) .^ 2 + (x2z + (-1) .* x4z)  ...
  .^ 2) .^ (-1 / 2)) .^ 2 + (((x1x + (-1) .* x3x) .^ 2 + (x1y + (-1) ...
   .* x3y) .^ 2 + (x1z + (-1) .* x3z) .^ 2) .^ (-1 / 2) .* (x1z + ( ...
  -1) .* x3z) + ((x2x + (-1) .* x4x) .^ 2 + (x2y + (-1) .* x4y) .^  ...
  2 + (x2z + (-1) .* x4z) .^ 2) .^ (-1 / 2) .* (x2z + (-1) .* x4z))  ...
  .^ 2) .^ (-3 / 2) .* ((x1z + (-1) .* x3z) .* (x2x + (-1) .* x4x) + ...
   (-1) .* (x1x + (-1) .* x3x) .* (x2z + (-1) .* x4z)) .* (2 .* ((( ...
  x1x + (-1) .* x3x) .^ 2 + (x1y + (-1) .* x3y) .^ 2 + (x1z + (-1)  ...
  .* x3z) .^ 2) .^ (-1 / 2) .* (x1z + (-1) .* x3z) + ((x2x + (-1) .* ...
   x4x) .^ 2 + (x2y + (-1) .* x4y) .^ 2 + (x2z + (-1) .* x4z) .^ 2)  ...
  .^ (-1 / 2) .* (x2z + (-1) .* x4z)) .* (((x2x + (-1) .* x4x) .^ 2  ...
  + (x2y + (-1) .* x4y) .^ 2 + (x2z + (-1) .* x4z) .^ 2) .^ (-1 / 2) ...
   + (-1) .* ((x2x + (-1) .* x4x) .^ 2 + (x2y + (-1) .* x4y) .^ 2 +  ...
  (x2z + (-1) .* x4z) .^ 2) .^ (-3 / 2) .* (x2z + (-1) .* x4z) .^ 2) ...
   + (-2) .* (x2x + (-1) .* x4x) .* ((x1x + (-1) .* x3x) .* ((x1x +  ...
  (-1) .* x3x) .^ 2 + (x1y + (-1) .* x3y) .^ 2 + (x1z + (-1) .* x3z) ...
   .^ 2) .^ (-1 / 2) + (x2x + (-1) .* x4x) .* ((x2x + (-1) .* x4x)  ...
  .^ 2 + (x2y + (-1) .* x4y) .^ 2 + (x2z + (-1) .* x4z) .^ 2) .^ ( ...
  -1 / 2)) .* ((x2x + (-1) .* x4x) .^ 2 + (x2y + (-1) .* x4y) .^ 2 + ...
   (x2z + (-1) .* x4z) .^ 2) .^ (-3 / 2) .* (x2z + (-1) .* x4z) + ( ...
  -2) .* (x2y + (-1) .* x4y) .* ((x1y + (-1) .* x3y) .* ((x1x + (-1) ...
   .* x3x) .^ 2 + (x1y + (-1) .* x3y) .^ 2 + (x1z + (-1) .* x3z) .^  ...
  2) .^ (-1 / 2) + (x2y + (-1) .* x4y) .* ((x2x + (-1) .* x4x) .^ 2  ...
  + (x2y + (-1) .* x4y) .^ 2 + (x2z + (-1) .* x4z) .^ 2) .^ (-1 / 2) ...
  ) .* ((x2x + (-1) .* x4x) .^ 2 + (x2y + (-1) .* x4y) .^ 2 + (x2z + ...
   (-1) .* x4z) .^ 2) .^ (-3 / 2) .* (x2z + (-1) .* x4z)) .* (((x1x  ...
  + (-1) .* x3x) .^ 2 + (x1y + (-1) .* x3y) .^ 2 + (x1z + (-1) .*  ...
  x3z) .^ 2) .^ (-1 / 2) .* (x1z + (-1) .* x3z) + ((x2x + (-1) .*  ...
  x4x) .^ 2 + (x2y + (-1) .* x4y) .^ 2 + (x2z + (-1) .* x4z) .^ 2)  ...
  .^ (-1 / 2) .* (x2z + (-1) .* x4z)) + ((((-1) .* x1y + x3y) .* ( ...
  x2x + (-1) .* x4x) + (x1x + (-1) .* x3x) .* (x2y + (-1) .* x4y))  ...
  .^ 2 + ((x1z + (-1) .* x3z) .* (x2x + (-1) .* x4x) + (-1) .* (x1x  ...
  + (-1) .* x3x) .* (x2z + (-1) .* x4z)) .^ 2 + (((-1) .* x1z + x3z) ...
   .* (x2y + (-1) .* x4y) + (x1y + (-1) .* x3y) .* (x2z + (-1) .*  ...
  x4z)) .^ 2) .^ (-1 / 2) .* (((x1x + (-1) .* x3x) .* ((x1x + (-1)  ...
  .* x3x) .^ 2 + (x1y + (-1) .* x3y) .^ 2 + (x1z + (-1) .* x3z) .^  ...
  2) .^ (-1 / 2) + (x2x + (-1) .* x4x) .* ((x2x + (-1) .* x4x) .^ 2  ...
  + (x2y + (-1) .* x4y) .^ 2 + (x2z + (-1) .* x4z) .^ 2) .^ (-1 / 2) ...
  ) .^ 2 + ((x1y + (-1) .* x3y) .* ((x1x + (-1) .* x3x) .^ 2 + (x1y  ...
  + (-1) .* x3y) .^ 2 + (x1z + (-1) .* x3z) .^ 2) .^ (-1 / 2) + ( ...
  x2y + (-1) .* x4y) .* ((x2x + (-1) .* x4x) .^ 2 + (x2y + (-1) .*  ...
  x4y) .^ 2 + (x2z + (-1) .* x4z) .^ 2) .^ (-1 / 2)) .^ 2 + (((x1x + ...
   (-1) .* x3x) .^ 2 + (x1y + (-1) .* x3y) .^ 2 + (x1z + (-1) .*  ...
  x3z) .^ 2) .^ (-1 / 2) .* (x1z + (-1) .* x3z) + ((x2x + (-1) .*  ...
  x4x) .^ 2 + (x2y + (-1) .* x4y) .^ 2 + (x2z + (-1) .* x4z) .^ 2)  ...
  .^ (-1 / 2) .* (x2z + (-1) .* x4z)) .^ 2) .^ (-1 / 2) .* ((x1z + ( ...
  -1) .* x3z) .* (x2x + (-1) .* x4x) + (-1) .* (x1x + (-1) .* x3x)  ...
  .* (x2z + (-1) .* x4z)) .* (((x2x + (-1) .* x4x) .^ 2 + (x2y + ( ...
  -1) .* x4y) .^ 2 + (x2z + (-1) .* x4z) .^ 2) .^ (-1 / 2) + (-1) .* ...
   ((x2x + (-1) .* x4x) .^ 2 + (x2y + (-1) .* x4y) .^ 2 + (x2z + ( ...
  -1) .* x4z) .^ 2) .^ (-3 / 2) .* (x2z + (-1) .* x4z) .^ 2) + ((( ...
  -1) .* x1y + x3y) .* (x2x + (-1) .* x4x) + (x1x + (-1) .* x3x) .*  ...
  (x2y + (-1) .* x4y)) .* (x2y + (-1) .* x4y) .* ((((-1) .* x1y +  ...
  x3y) .* (x2x + (-1) .* x4x) + (x1x + (-1) .* x3x) .* (x2y + (-1)  ...
  .* x4y)) .^ 2 + ((x1z + (-1) .* x3z) .* (x2x + (-1) .* x4x) + (-1) ...
   .* (x1x + (-1) .* x3x) .* (x2z + (-1) .* x4z)) .^ 2 + (((-1) .*  ...
  x1z + x3z) .* (x2y + (-1) .* x4y) + (x1y + (-1) .* x3y) .* (x2z +  ...
  (-1) .* x4z)) .^ 2) .^ (-1 / 2) .* (((x1x + (-1) .* x3x) .* ((x1x  ...
  + (-1) .* x3x) .^ 2 + (x1y + (-1) .* x3y) .^ 2 + (x1z + (-1) .*  ...
  x3z) .^ 2) .^ (-1 / 2) + (x2x + (-1) .* x4x) .* ((x2x + (-1) .*  ...
  x4x) .^ 2 + (x2y + (-1) .* x4y) .^ 2 + (x2z + (-1) .* x4z) .^ 2)  ...
  .^ (-1 / 2)) .^ 2 + ((x1y + (-1) .* x3y) .* ((x1x + (-1) .* x3x)  ...
  .^ 2 + (x1y + (-1) .* x3y) .^ 2 + (x1z + (-1) .* x3z) .^ 2) .^ ( ...
  -1 / 2) + (x2y + (-1) .* x4y) .* ((x2x + (-1) .* x4x) .^ 2 + (x2y  ...
  + (-1) .* x4y) .^ 2 + (x2z + (-1) .* x4z) .^ 2) .^ (-1 / 2)) .^ 2  ...
  + (((x1x + (-1) .* x3x) .^ 2 + (x1y + (-1) .* x3y) .^ 2 + (x1z + ( ...
  -1) .* x3z) .^ 2) .^ (-1 / 2) .* (x1z + (-1) .* x3z) + ((x2x + ( ...
  -1) .* x4x) .^ 2 + (x2y + (-1) .* x4y) .^ 2 + (x2z + (-1) .* x4z)  ...
  .^ 2) .^ (-1 / 2) .* (x2z + (-1) .* x4z)) .^ 2) .^ (-1 / 2) .* (( ...
  x2x + (-1) .* x4x) .^ 2 + (x2y + (-1) .* x4y) .^ 2 + (x2z + (-1)  ...
  .* x4z) .^ 2) .^ (-3 / 2) .* (x2z + (-1) .* x4z),(-1) .* (x1x + ( ...
  -1) .* x3x) .* (x1y + (-1) .* x3y) .* ((x1x + (-1) .* x3x) .^ 2 +  ...
  (x1y + (-1) .* x3y) .^ 2 + (x1z + (-1) .* x3z) .^ 2) .^ (-3 / 2)  ...
  .* (((-1) .* x1y + x3y) .* (x2x + (-1) .* x4x) + (x1x + (-1) .*  ...
  x3x) .* (x2y + (-1) .* x4y)) .* ((((-1) .* x1y + x3y) .* (x2x + ( ...
  -1) .* x4x) + (x1x + (-1) .* x3x) .* (x2y + (-1) .* x4y)) .^ 2 + ( ...
  (x1z + (-1) .* x3z) .* (x2x + (-1) .* x4x) + (-1) .* (x1x + (-1)  ...
  .* x3x) .* (x2z + (-1) .* x4z)) .^ 2 + (((-1) .* x1z + x3z) .* ( ...
  x2y + (-1) .* x4y) + (x1y + (-1) .* x3y) .* (x2z + (-1) .* x4z))  ...
  .^ 2) .^ (-1 / 2) .* (((x1x + (-1) .* x3x) .* ((x1x + (-1) .* x3x) ...
   .^ 2 + (x1y + (-1) .* x3y) .^ 2 + (x1z + (-1) .* x3z) .^ 2) .^ ( ...
  -1 / 2) + (x2x + (-1) .* x4x) .* ((x2x + (-1) .* x4x) .^ 2 + (x2y  ...
  + (-1) .* x4y) .^ 2 + (x2z + (-1) .* x4z) .^ 2) .^ (-1 / 2)) .^ 2  ...
  + ((x1y + (-1) .* x3y) .* ((x1x + (-1) .* x3x) .^ 2 + (x1y + (-1)  ...
  .* x3y) .^ 2 + (x1z + (-1) .* x3z) .^ 2) .^ (-1 / 2) + (x2y + (-1) ...
   .* x4y) .* ((x2x + (-1) .* x4x) .^ 2 + (x2y + (-1) .* x4y) .^ 2 + ...
   (x2z + (-1) .* x4z) .^ 2) .^ (-1 / 2)) .^ 2 + (((x1x + (-1) .*  ...
  x3x) .^ 2 + (x1y + (-1) .* x3y) .^ 2 + (x1z + (-1) .* x3z) .^ 2)  ...
  .^ (-1 / 2) .* (x1z + (-1) .* x3z) + ((x2x + (-1) .* x4x) .^ 2 + ( ...
  x2y + (-1) .* x4y) .^ 2 + (x2z + (-1) .* x4z) .^ 2) .^ (-1 / 2) .* ...
   (x2z + (-1) .* x4z)) .^ 2) .^ (-1 / 2) + (1 / 2) .* (((-1) .*  ...
  x1y + x3y) .* (x2x + (-1) .* x4x) + (x1x + (-1) .* x3x) .* (x2y +  ...
  (-1) .* x4y)) .* ((((-1) .* x1y + x3y) .* (x2x + (-1) .* x4x) + ( ...
  x1x + (-1) .* x3x) .* (x2y + (-1) .* x4y)) .^ 2 + ((x1z + (-1) .*  ...
  x3z) .* (x2x + (-1) .* x4x) + (-1) .* (x1x + (-1) .* x3x) .* (x2z  ...
  + (-1) .* x4z)) .^ 2 + (((-1) .* x1z + x3z) .* (x2y + (-1) .* x4y) ...
   + (x1y + (-1) .* x3y) .* (x2z + (-1) .* x4z)) .^ 2) .^ (-1 / 2)  ...
  .* (2 .* ((x1x + (-1) .* x3x) .^ 2 .* ((x1x + (-1) .* x3x) .^ 2 +  ...
  (x1y + (-1) .* x3y) .^ 2 + (x1z + (-1) .* x3z) .^ 2) .^ (-3 / 2) + ...
   (-1) .* ((x1x + (-1) .* x3x) .^ 2 + (x1y + (-1) .* x3y) .^ 2 + ( ...
  x1z + (-1) .* x3z) .^ 2) .^ (-1 / 2)) .* ((x1x + (-1) .* x3x) .* ( ...
  (x1x + (-1) .* x3x) .^ 2 + (x1y + (-1) .* x3y) .^ 2 + (x1z + (-1)  ...
  .* x3z) .^ 2) .^ (-1 / 2) + (x2x + (-1) .* x4x) .* ((x2x + (-1) .* ...
   x4x) .^ 2 + (x2y + (-1) .* x4y) .^ 2 + (x2z + (-1) .* x4z) .^ 2)  ...
  .^ (-1 / 2)) + 2 .* (x1x + (-1) .* x3x) .* (x1y + (-1) .* x3y) .*  ...
  ((x1x + (-1) .* x3x) .^ 2 + (x1y + (-1) .* x3y) .^ 2 + (x1z + (-1) ...
   .* x3z) .^ 2) .^ (-3 / 2) .* ((x1y + (-1) .* x3y) .* ((x1x + (-1) ...
   .* x3x) .^ 2 + (x1y + (-1) .* x3y) .^ 2 + (x1z + (-1) .* x3z) .^  ...
  2) .^ (-1 / 2) + (x2y + (-1) .* x4y) .* ((x2x + (-1) .* x4x) .^ 2  ...
  + (x2y + (-1) .* x4y) .^ 2 + (x2z + (-1) .* x4z) .^ 2) .^ (-1 / 2) ...
  ) + 2 .* (x1x + (-1) .* x3x) .* ((x1x + (-1) .* x3x) .^ 2 + (x1y + ...
   (-1) .* x3y) .^ 2 + (x1z + (-1) .* x3z) .^ 2) .^ (-3 / 2) .* ( ...
  x1z + (-1) .* x3z) .* (((x1x + (-1) .* x3x) .^ 2 + (x1y + (-1) .*  ...
  x3y) .^ 2 + (x1z + (-1) .* x3z) .^ 2) .^ (-1 / 2) .* (x1z + (-1)  ...
  .* x3z) + ((x2x + (-1) .* x4x) .^ 2 + (x2y + (-1) .* x4y) .^ 2 + ( ...
  x2z + (-1) .* x4z) .^ 2) .^ (-1 / 2) .* (x2z + (-1) .* x4z))) .* ( ...
  ((x1x + (-1) .* x3x) .* ((x1x + (-1) .* x3x) .^ 2 + (x1y + (-1) .* ...
   x3y) .^ 2 + (x1z + (-1) .* x3z) .^ 2) .^ (-1 / 2) + (x2x + (-1)  ...
  .* x4x) .* ((x2x + (-1) .* x4x) .^ 2 + (x2y + (-1) .* x4y) .^ 2 +  ...
  (x2z + (-1) .* x4z) .^ 2) .^ (-1 / 2)) .^ 2 + ((x1y + (-1) .* x3y) ...
   .* ((x1x + (-1) .* x3x) .^ 2 + (x1y + (-1) .* x3y) .^ 2 + (x1z +  ...
  (-1) .* x3z) .^ 2) .^ (-1 / 2) + (x2y + (-1) .* x4y) .* ((x2x + ( ...
  -1) .* x4x) .^ 2 + (x2y + (-1) .* x4y) .^ 2 + (x2z + (-1) .* x4z)  ...
  .^ 2) .^ (-1 / 2)) .^ 2 + (((x1x + (-1) .* x3x) .^ 2 + (x1y + (-1) ...
   .* x3y) .^ 2 + (x1z + (-1) .* x3z) .^ 2) .^ (-1 / 2) .* (x1z + ( ...
  -1) .* x3z) + ((x2x + (-1) .* x4x) .^ 2 + (x2y + (-1) .* x4y) .^  ...
  2 + (x2z + (-1) .* x4z) .^ 2) .^ (-1 / 2) .* (x2z + (-1) .* x4z))  ...
  .^ 2) .^ (-3 / 2) .* ((x1y + (-1) .* x3y) .* ((x1x + (-1) .* x3x)  ...
  .^ 2 + (x1y + (-1) .* x3y) .^ 2 + (x1z + (-1) .* x3z) .^ 2) .^ ( ...
  -1 / 2) + (x2y + (-1) .* x4y) .* ((x2x + (-1) .* x4x) .^ 2 + (x2y  ...
  + (-1) .* x4y) .^ 2 + (x2z + (-1) .* x4z) .^ 2) .^ (-1 / 2)) + ( ...
  -1) .* ((-1) .* x2y + x4y) .* ((((-1) .* x1y + x3y) .* (x2x + (-1) ...
   .* x4x) + (x1x + (-1) .* x3x) .* (x2y + (-1) .* x4y)) .^ 2 + (( ...
  x1z + (-1) .* x3z) .* (x2x + (-1) .* x4x) + (-1) .* (x1x + (-1) .* ...
   x3x) .* (x2z + (-1) .* x4z)) .^ 2 + (((-1) .* x1z + x3z) .* (x2y  ...
  + (-1) .* x4y) + (x1y + (-1) .* x3y) .* (x2z + (-1) .* x4z)) .^ 2) ...
   .^ (-1 / 2) .* (((x1x + (-1) .* x3x) .* ((x1x + (-1) .* x3x) .^  ...
  2 + (x1y + (-1) .* x3y) .^ 2 + (x1z + (-1) .* x3z) .^ 2) .^ (-1 /  ...
  2) + (x2x + (-1) .* x4x) .* ((x2x + (-1) .* x4x) .^ 2 + (x2y + ( ...
  -1) .* x4y) .^ 2 + (x2z + (-1) .* x4z) .^ 2) .^ (-1 / 2)) .^ 2 + ( ...
  (x1y + (-1) .* x3y) .* ((x1x + (-1) .* x3x) .^ 2 + (x1y + (-1) .*  ...
  x3y) .^ 2 + (x1z + (-1) .* x3z) .^ 2) .^ (-1 / 2) + (x2y + (-1) .* ...
   x4y) .* ((x2x + (-1) .* x4x) .^ 2 + (x2y + (-1) .* x4y) .^ 2 + ( ...
  x2z + (-1) .* x4z) .^ 2) .^ (-1 / 2)) .^ 2 + (((x1x + (-1) .* x3x) ...
   .^ 2 + (x1y + (-1) .* x3y) .^ 2 + (x1z + (-1) .* x3z) .^ 2) .^ ( ...
  -1 / 2) .* (x1z + (-1) .* x3z) + ((x2x + (-1) .* x4x) .^ 2 + (x2y  ...
  + (-1) .* x4y) .^ 2 + (x2z + (-1) .* x4z) .^ 2) .^ (-1 / 2) .* ( ...
  x2z + (-1) .* x4z)) .^ 2) .^ (-1 / 2) .* ((x1y + (-1) .* x3y) .* ( ...
  (x1x + (-1) .* x3x) .^ 2 + (x1y + (-1) .* x3y) .^ 2 + (x1z + (-1)  ...
  .* x3z) .^ 2) .^ (-1 / 2) + (x2y + (-1) .* x4y) .* ((x2x + (-1) .* ...
   x4x) .^ 2 + (x2y + (-1) .* x4y) .^ 2 + (x2z + (-1) .* x4z) .^ 2)  ...
  .^ (-1 / 2)) + (x1x + (-1) .* x3x) .* ((x1x + (-1) .* x3x) .^ 2 +  ...
  (x1y + (-1) .* x3y) .^ 2 + (x1z + (-1) .* x3z) .^ 2) .^ (-3 / 2)  ...
  .* (x1z + (-1) .* x3z) .* ((((-1) .* x1y + x3y) .* (x2x + (-1) .*  ...
  x4x) + (x1x + (-1) .* x3x) .* (x2y + (-1) .* x4y)) .^ 2 + ((x1z +  ...
  (-1) .* x3z) .* (x2x + (-1) .* x4x) + (-1) .* (x1x + (-1) .* x3x)  ...
  .* (x2z + (-1) .* x4z)) .^ 2 + (((-1) .* x1z + x3z) .* (x2y + (-1) ...
   .* x4y) + (x1y + (-1) .* x3y) .* (x2z + (-1) .* x4z)) .^ 2) .^ ( ...
  -1 / 2) .* (((x1x + (-1) .* x3x) .* ((x1x + (-1) .* x3x) .^ 2 + ( ...
  x1y + (-1) .* x3y) .^ 2 + (x1z + (-1) .* x3z) .^ 2) .^ (-1 / 2) +  ...
  (x2x + (-1) .* x4x) .* ((x2x + (-1) .* x4x) .^ 2 + (x2y + (-1) .*  ...
  x4y) .^ 2 + (x2z + (-1) .* x4z) .^ 2) .^ (-1 / 2)) .^ 2 + ((x1y +  ...
  (-1) .* x3y) .* ((x1x + (-1) .* x3x) .^ 2 + (x1y + (-1) .* x3y)  ...
  .^ 2 + (x1z + (-1) .* x3z) .^ 2) .^ (-1 / 2) + (x2y + (-1) .* x4y) ...
   .* ((x2x + (-1) .* x4x) .^ 2 + (x2y + (-1) .* x4y) .^ 2 + (x2z +  ...
  (-1) .* x4z) .^ 2) .^ (-1 / 2)) .^ 2 + (((x1x + (-1) .* x3x) .^ 2  ...
  + (x1y + (-1) .* x3y) .^ 2 + (x1z + (-1) .* x3z) .^ 2) .^ (-1 / 2) ...
   .* (x1z + (-1) .* x3z) + ((x2x + (-1) .* x4x) .^ 2 + (x2y + (-1)  ...
  .* x4y) .^ 2 + (x2z + (-1) .* x4z) .^ 2) .^ (-1 / 2) .* (x2z + ( ...
  -1) .* x4z)) .^ 2) .^ (-1 / 2) .* ((x1z + (-1) .* x3z) .* (x2x + ( ...
  -1) .* x4x) + (-1) .* (x1x + (-1) .* x3x) .* (x2z + (-1) .* x4z))  ...
  + (1 / 2) .* (((-1) .* x1y + x3y) .* (x2x + (-1) .* x4x) + (x1x +  ...
  (-1) .* x3x) .* (x2y + (-1) .* x4y)) .* ((((-1) .* x1y + x3y) .* ( ...
  x2x + (-1) .* x4x) + (x1x + (-1) .* x3x) .* (x2y + (-1) .* x4y))  ...
  .^ 2 + ((x1z + (-1) .* x3z) .* (x2x + (-1) .* x4x) + (-1) .* (x1x  ...
  + (-1) .* x3x) .* (x2z + (-1) .* x4z)) .^ 2 + (((-1) .* x1z + x3z) ...
   .* (x2y + (-1) .* x4y) + (x1y + (-1) .* x3y) .* (x2z + (-1) .*  ...
  x4z)) .^ 2) .^ (-3 / 2) .* (((x1x + (-1) .* x3x) .* ((x1x + (-1)  ...
  .* x3x) .^ 2 + (x1y + (-1) .* x3y) .^ 2 + (x1z + (-1) .* x3z) .^  ...
  2) .^ (-1 / 2) + (x2x + (-1) .* x4x) .* ((x2x + (-1) .* x4x) .^ 2  ...
  + (x2y + (-1) .* x4y) .^ 2 + (x2z + (-1) .* x4z) .^ 2) .^ (-1 / 2) ...
  ) .^ 2 + ((x1y + (-1) .* x3y) .* ((x1x + (-1) .* x3x) .^ 2 + (x1y  ...
  + (-1) .* x3y) .^ 2 + (x1z + (-1) .* x3z) .^ 2) .^ (-1 / 2) + ( ...
  x2y + (-1) .* x4y) .* ((x2x + (-1) .* x4x) .^ 2 + (x2y + (-1) .*  ...
  x4y) .^ 2 + (x2z + (-1) .* x4z) .^ 2) .^ (-1 / 2)) .^ 2 + (((x1x + ...
   (-1) .* x3x) .^ 2 + (x1y + (-1) .* x3y) .^ 2 + (x1z + (-1) .*  ...
  x3z) .^ 2) .^ (-1 / 2) .* (x1z + (-1) .* x3z) + ((x2x + (-1) .*  ...
  x4x) .^ 2 + (x2y + (-1) .* x4y) .^ 2 + (x2z + (-1) .* x4z) .^ 2)  ...
  .^ (-1 / 2) .* (x2z + (-1) .* x4z)) .^ 2) .^ (-1 / 2) .* ((x1y + ( ...
  -1) .* x3y) .* ((x1x + (-1) .* x3x) .^ 2 + (x1y + (-1) .* x3y) .^  ...
  2 + (x1z + (-1) .* x3z) .^ 2) .^ (-1 / 2) + (x2y + (-1) .* x4y) .* ...
   ((x2x + (-1) .* x4x) .^ 2 + (x2y + (-1) .* x4y) .^ 2 + (x2z + ( ...
  -1) .* x4z) .^ 2) .^ (-1 / 2)) .* (2 .* (((-1) .* x1y + x3y) .* ( ...
  x2x + (-1) .* x4x) + (x1x + (-1) .* x3x) .* (x2y + (-1) .* x4y))  ...
  .* ((-1) .* x2y + x4y) + 2 .* ((x1z + (-1) .* x3z) .* (x2x + (-1)  ...
  .* x4x) + (-1) .* (x1x + (-1) .* x3x) .* (x2z + (-1) .* x4z)) .* ( ...
  x2z + (-1) .* x4z)) + (-1 / 2) .* ((((-1) .* x1y + x3y) .* (x2x +  ...
  (-1) .* x4x) + (x1x + (-1) .* x3x) .* (x2y + (-1) .* x4y)) .^ 2 +  ...
  ((x1z + (-1) .* x3z) .* (x2x + (-1) .* x4x) + (-1) .* (x1x + (-1)  ...
  .* x3x) .* (x2z + (-1) .* x4z)) .^ 2 + (((-1) .* x1z + x3z) .* ( ...
  x2y + (-1) .* x4y) + (x1y + (-1) .* x3y) .* (x2z + (-1) .* x4z))  ...
  .^ 2) .^ (-1 / 2) .* (2 .* ((x1x + (-1) .* x3x) .^ 2 .* ((x1x + ( ...
  -1) .* x3x) .^ 2 + (x1y + (-1) .* x3y) .^ 2 + (x1z + (-1) .* x3z)  ...
  .^ 2) .^ (-3 / 2) + (-1) .* ((x1x + (-1) .* x3x) .^ 2 + (x1y + ( ...
  -1) .* x3y) .^ 2 + (x1z + (-1) .* x3z) .^ 2) .^ (-1 / 2)) .* (( ...
  x1x + (-1) .* x3x) .* ((x1x + (-1) .* x3x) .^ 2 + (x1y + (-1) .*  ...
  x3y) .^ 2 + (x1z + (-1) .* x3z) .^ 2) .^ (-1 / 2) + (x2x + (-1) .* ...
   x4x) .* ((x2x + (-1) .* x4x) .^ 2 + (x2y + (-1) .* x4y) .^ 2 + ( ...
  x2z + (-1) .* x4z) .^ 2) .^ (-1 / 2)) + 2 .* (x1x + (-1) .* x3x)  ...
  .* (x1y + (-1) .* x3y) .* ((x1x + (-1) .* x3x) .^ 2 + (x1y + (-1)  ...
  .* x3y) .^ 2 + (x1z + (-1) .* x3z) .^ 2) .^ (-3 / 2) .* ((x1y + ( ...
  -1) .* x3y) .* ((x1x + (-1) .* x3x) .^ 2 + (x1y + (-1) .* x3y) .^  ...
  2 + (x1z + (-1) .* x3z) .^ 2) .^ (-1 / 2) + (x2y + (-1) .* x4y) .* ...
   ((x2x + (-1) .* x4x) .^ 2 + (x2y + (-1) .* x4y) .^ 2 + (x2z + ( ...
  -1) .* x4z) .^ 2) .^ (-1 / 2)) + 2 .* (x1x + (-1) .* x3x) .* (( ...
  x1x + (-1) .* x3x) .^ 2 + (x1y + (-1) .* x3y) .^ 2 + (x1z + (-1)  ...
  .* x3z) .^ 2) .^ (-3 / 2) .* (x1z + (-1) .* x3z) .* (((x1x + (-1)  ...
  .* x3x) .^ 2 + (x1y + (-1) .* x3y) .^ 2 + (x1z + (-1) .* x3z) .^  ...
  2) .^ (-1 / 2) .* (x1z + (-1) .* x3z) + ((x2x + (-1) .* x4x) .^ 2  ...
  + (x2y + (-1) .* x4y) .^ 2 + (x2z + (-1) .* x4z) .^ 2) .^ (-1 / 2) ...
   .* (x2z + (-1) .* x4z))) .* (((x1x + (-1) .* x3x) .* ((x1x + (-1) ...
   .* x3x) .^ 2 + (x1y + (-1) .* x3y) .^ 2 + (x1z + (-1) .* x3z) .^  ...
  2) .^ (-1 / 2) + (x2x + (-1) .* x4x) .* ((x2x + (-1) .* x4x) .^ 2  ...
  + (x2y + (-1) .* x4y) .^ 2 + (x2z + (-1) .* x4z) .^ 2) .^ (-1 / 2) ...
  ) .^ 2 + ((x1y + (-1) .* x3y) .* ((x1x + (-1) .* x3x) .^ 2 + (x1y  ...
  + (-1) .* x3y) .^ 2 + (x1z + (-1) .* x3z) .^ 2) .^ (-1 / 2) + ( ...
  x2y + (-1) .* x4y) .* ((x2x + (-1) .* x4x) .^ 2 + (x2y + (-1) .*  ...
  x4y) .^ 2 + (x2z + (-1) .* x4z) .^ 2) .^ (-1 / 2)) .^ 2 + (((x1x + ...
   (-1) .* x3x) .^ 2 + (x1y + (-1) .* x3y) .^ 2 + (x1z + (-1) .*  ...
  x3z) .^ 2) .^ (-1 / 2) .* (x1z + (-1) .* x3z) + ((x2x + (-1) .*  ...
  x4x) .^ 2 + (x2y + (-1) .* x4y) .^ 2 + (x2z + (-1) .* x4z) .^ 2)  ...
  .^ (-1 / 2) .* (x2z + (-1) .* x4z)) .^ 2) .^ (-3 / 2) .* ((x1z + ( ...
  -1) .* x3z) .* (x2x + (-1) .* x4x) + (-1) .* (x1x + (-1) .* x3x)  ...
  .* (x2z + (-1) .* x4z)) .* (((x1x + (-1) .* x3x) .^ 2 + (x1y + ( ...
  -1) .* x3y) .^ 2 + (x1z + (-1) .* x3z) .^ 2) .^ (-1 / 2) .* (x1z + ...
   (-1) .* x3z) + ((x2x + (-1) .* x4x) .^ 2 + (x2y + (-1) .* x4y)  ...
  .^ 2 + (x2z + (-1) .* x4z) .^ 2) .^ (-1 / 2) .* (x2z + (-1) .*  ...
  x4z)) + (-1 / 2) .* ((((-1) .* x1y + x3y) .* (x2x + (-1) .* x4x) + ...
   (x1x + (-1) .* x3x) .* (x2y + (-1) .* x4y)) .^ 2 + ((x1z + (-1)  ...
  .* x3z) .* (x2x + (-1) .* x4x) + (-1) .* (x1x + (-1) .* x3x) .* ( ...
  x2z + (-1) .* x4z)) .^ 2 + (((-1) .* x1z + x3z) .* (x2y + (-1) .*  ...
  x4y) + (x1y + (-1) .* x3y) .* (x2z + (-1) .* x4z)) .^ 2) .^ (-3 /  ...
  2) .* (((x1x + (-1) .* x3x) .* ((x1x + (-1) .* x3x) .^ 2 + (x1y +  ...
  (-1) .* x3y) .^ 2 + (x1z + (-1) .* x3z) .^ 2) .^ (-1 / 2) + (x2x + ...
   (-1) .* x4x) .* ((x2x + (-1) .* x4x) .^ 2 + (x2y + (-1) .* x4y)  ...
  .^ 2 + (x2z + (-1) .* x4z) .^ 2) .^ (-1 / 2)) .^ 2 + ((x1y + (-1)  ...
  .* x3y) .* ((x1x + (-1) .* x3x) .^ 2 + (x1y + (-1) .* x3y) .^ 2 +  ...
  (x1z + (-1) .* x3z) .^ 2) .^ (-1 / 2) + (x2y + (-1) .* x4y) .* (( ...
  x2x + (-1) .* x4x) .^ 2 + (x2y + (-1) .* x4y) .^ 2 + (x2z + (-1)  ...
  .* x4z) .^ 2) .^ (-1 / 2)) .^ 2 + (((x1x + (-1) .* x3x) .^ 2 + ( ...
  x1y + (-1) .* x3y) .^ 2 + (x1z + (-1) .* x3z) .^ 2) .^ (-1 / 2) .* ...
   (x1z + (-1) .* x3z) + ((x2x + (-1) .* x4x) .^ 2 + (x2y + (-1) .*  ...
  x4y) .^ 2 + (x2z + (-1) .* x4z) .^ 2) .^ (-1 / 2) .* (x2z + (-1)  ...
  .* x4z)) .^ 2) .^ (-1 / 2) .* ((x1z + (-1) .* x3z) .* (x2x + (-1)  ...
  .* x4x) + (-1) .* (x1x + (-1) .* x3x) .* (x2z + (-1) .* x4z)) .* ( ...
  2 .* (((-1) .* x1y + x3y) .* (x2x + (-1) .* x4x) + (x1x + (-1) .*  ...
  x3x) .* (x2y + (-1) .* x4y)) .* ((-1) .* x2y + x4y) + 2 .* ((x1z + ...
   (-1) .* x3z) .* (x2x + (-1) .* x4x) + (-1) .* (x1x + (-1) .* x3x) ...
   .* (x2z + (-1) .* x4z)) .* (x2z + (-1) .* x4z)) .* (((x1x + (-1)  ...
  .* x3x) .^ 2 + (x1y + (-1) .* x3y) .^ 2 + (x1z + (-1) .* x3z) .^  ...
  2) .^ (-1 / 2) .* (x1z + (-1) .* x3z) + ((x2x + (-1) .* x4x) .^ 2  ...
  + (x2y + (-1) .* x4y) .^ 2 + (x2z + (-1) .* x4z) .^ 2) .^ (-1 / 2) ...
   .* (x2z + (-1) .* x4z)) + ((((-1) .* x1y + x3y) .* (x2x + (-1) .* ...
   x4x) + (x1x + (-1) .* x3x) .* (x2y + (-1) .* x4y)) .^ 2 + ((x1z + ...
   (-1) .* x3z) .* (x2x + (-1) .* x4x) + (-1) .* (x1x + (-1) .* x3x) ...
   .* (x2z + (-1) .* x4z)) .^ 2 + (((-1) .* x1z + x3z) .* (x2y + ( ...
  -1) .* x4y) + (x1y + (-1) .* x3y) .* (x2z + (-1) .* x4z)) .^ 2)  ...
  .^ (-1 / 2) .* (((x1x + (-1) .* x3x) .* ((x1x + (-1) .* x3x) .^ 2  ...
  + (x1y + (-1) .* x3y) .^ 2 + (x1z + (-1) .* x3z) .^ 2) .^ (-1 / 2) ...
   + (x2x + (-1) .* x4x) .* ((x2x + (-1) .* x4x) .^ 2 + (x2y + (-1)  ...
  .* x4y) .^ 2 + (x2z + (-1) .* x4z) .^ 2) .^ (-1 / 2)) .^ 2 + (( ...
  x1y + (-1) .* x3y) .* ((x1x + (-1) .* x3x) .^ 2 + (x1y + (-1) .*  ...
  x3y) .^ 2 + (x1z + (-1) .* x3z) .^ 2) .^ (-1 / 2) + (x2y + (-1) .* ...
   x4y) .* ((x2x + (-1) .* x4x) .^ 2 + (x2y + (-1) .* x4y) .^ 2 + ( ...
  x2z + (-1) .* x4z) .^ 2) .^ (-1 / 2)) .^ 2 + (((x1x + (-1) .* x3x) ...
   .^ 2 + (x1y + (-1) .* x3y) .^ 2 + (x1z + (-1) .* x3z) .^ 2) .^ ( ...
  -1 / 2) .* (x1z + (-1) .* x3z) + ((x2x + (-1) .* x4x) .^ 2 + (x2y  ...
  + (-1) .* x4y) .^ 2 + (x2z + (-1) .* x4z) .^ 2) .^ (-1 / 2) .* ( ...
  x2z + (-1) .* x4z)) .^ 2) .^ (-1 / 2) .* (((x1x + (-1) .* x3x) .^  ...
  2 + (x1y + (-1) .* x3y) .^ 2 + (x1z + (-1) .* x3z) .^ 2) .^ (-1 /  ...
  2) .* (x1z + (-1) .* x3z) + ((x2x + (-1) .* x4x) .^ 2 + (x2y + ( ...
  -1) .* x4y) .^ 2 + (x2z + (-1) .* x4z) .^ 2) .^ (-1 / 2) .* (x2z + ...
   (-1) .* x4z)) .* (x2z + (-1) .* x4z),(-1) .* ((x1y + (-1) .* x3y) ...
   .^ 2 .* ((x1x + (-1) .* x3x) .^ 2 + (x1y + (-1) .* x3y) .^ 2 + ( ...
  x1z + (-1) .* x3z) .^ 2) .^ (-3 / 2) + (-1) .* ((x1x + (-1) .*  ...
  x3x) .^ 2 + (x1y + (-1) .* x3y) .^ 2 + (x1z + (-1) .* x3z) .^ 2)  ...
  .^ (-1 / 2)) .* (((-1) .* x1y + x3y) .* (x2x + (-1) .* x4x) + ( ...
  x1x + (-1) .* x3x) .* (x2y + (-1) .* x4y)) .* ((((-1) .* x1y +  ...
  x3y) .* (x2x + (-1) .* x4x) + (x1x + (-1) .* x3x) .* (x2y + (-1)  ...
  .* x4y)) .^ 2 + ((x1z + (-1) .* x3z) .* (x2x + (-1) .* x4x) + (-1) ...
   .* (x1x + (-1) .* x3x) .* (x2z + (-1) .* x4z)) .^ 2 + (((-1) .*  ...
  x1z + x3z) .* (x2y + (-1) .* x4y) + (x1y + (-1) .* x3y) .* (x2z +  ...
  (-1) .* x4z)) .^ 2) .^ (-1 / 2) .* (((x1x + (-1) .* x3x) .* ((x1x  ...
  + (-1) .* x3x) .^ 2 + (x1y + (-1) .* x3y) .^ 2 + (x1z + (-1) .*  ...
  x3z) .^ 2) .^ (-1 / 2) + (x2x + (-1) .* x4x) .* ((x2x + (-1) .*  ...
  x4x) .^ 2 + (x2y + (-1) .* x4y) .^ 2 + (x2z + (-1) .* x4z) .^ 2)  ...
  .^ (-1 / 2)) .^ 2 + ((x1y + (-1) .* x3y) .* ((x1x + (-1) .* x3x)  ...
  .^ 2 + (x1y + (-1) .* x3y) .^ 2 + (x1z + (-1) .* x3z) .^ 2) .^ ( ...
  -1 / 2) + (x2y + (-1) .* x4y) .* ((x2x + (-1) .* x4x) .^ 2 + (x2y  ...
  + (-1) .* x4y) .^ 2 + (x2z + (-1) .* x4z) .^ 2) .^ (-1 / 2)) .^ 2  ...
  + (((x1x + (-1) .* x3x) .^ 2 + (x1y + (-1) .* x3y) .^ 2 + (x1z + ( ...
  -1) .* x3z) .^ 2) .^ (-1 / 2) .* (x1z + (-1) .* x3z) + ((x2x + ( ...
  -1) .* x4x) .^ 2 + (x2y + (-1) .* x4y) .^ 2 + (x2z + (-1) .* x4z)  ...
  .^ 2) .^ (-1 / 2) .* (x2z + (-1) .* x4z)) .^ 2) .^ (-1 / 2) + (1  ...
  / 2) .* (((-1) .* x1y + x3y) .* (x2x + (-1) .* x4x) + (x1x + (-1)  ...
  .* x3x) .* (x2y + (-1) .* x4y)) .* ((((-1) .* x1y + x3y) .* (x2x + ...
   (-1) .* x4x) + (x1x + (-1) .* x3x) .* (x2y + (-1) .* x4y)) .^ 2 + ...
   ((x1z + (-1) .* x3z) .* (x2x + (-1) .* x4x) + (-1) .* (x1x + (-1) ...
   .* x3x) .* (x2z + (-1) .* x4z)) .^ 2 + (((-1) .* x1z + x3z) .* ( ...
  x2y + (-1) .* x4y) + (x1y + (-1) .* x3y) .* (x2z + (-1) .* x4z))  ...
  .^ 2) .^ (-1 / 2) .* (2 .* (x1x + (-1) .* x3x) .* (x1y + (-1) .*  ...
  x3y) .* ((x1x + (-1) .* x3x) .^ 2 + (x1y + (-1) .* x3y) .^ 2 + ( ...
  x1z + (-1) .* x3z) .^ 2) .^ (-3 / 2) .* ((x1x + (-1) .* x3x) .* (( ...
  x1x + (-1) .* x3x) .^ 2 + (x1y + (-1) .* x3y) .^ 2 + (x1z + (-1)  ...
  .* x3z) .^ 2) .^ (-1 / 2) + (x2x + (-1) .* x4x) .* ((x2x + (-1) .* ...
   x4x) .^ 2 + (x2y + (-1) .* x4y) .^ 2 + (x2z + (-1) .* x4z) .^ 2)  ...
  .^ (-1 / 2)) + 2 .* ((x1y + (-1) .* x3y) .^ 2 .* ((x1x + (-1) .*  ...
  x3x) .^ 2 + (x1y + (-1) .* x3y) .^ 2 + (x1z + (-1) .* x3z) .^ 2)  ...
  .^ (-3 / 2) + (-1) .* ((x1x + (-1) .* x3x) .^ 2 + (x1y + (-1) .*  ...
  x3y) .^ 2 + (x1z + (-1) .* x3z) .^ 2) .^ (-1 / 2)) .* ((x1y + (-1) ...
   .* x3y) .* ((x1x + (-1) .* x3x) .^ 2 + (x1y + (-1) .* x3y) .^ 2 + ...
   (x1z + (-1) .* x3z) .^ 2) .^ (-1 / 2) + (x2y + (-1) .* x4y) .* (( ...
  x2x + (-1) .* x4x) .^ 2 + (x2y + (-1) .* x4y) .^ 2 + (x2z + (-1)  ...
  .* x4z) .^ 2) .^ (-1 / 2)) + 2 .* (x1y + (-1) .* x3y) .* ((x1x + ( ...
  -1) .* x3x) .^ 2 + (x1y + (-1) .* x3y) .^ 2 + (x1z + (-1) .* x3z)  ...
  .^ 2) .^ (-3 / 2) .* (x1z + (-1) .* x3z) .* (((x1x + (-1) .* x3x)  ...
  .^ 2 + (x1y + (-1) .* x3y) .^ 2 + (x1z + (-1) .* x3z) .^ 2) .^ ( ...
  -1 / 2) .* (x1z + (-1) .* x3z) + ((x2x + (-1) .* x4x) .^ 2 + (x2y  ...
  + (-1) .* x4y) .^ 2 + (x2z + (-1) .* x4z) .^ 2) .^ (-1 / 2) .* ( ...
  x2z + (-1) .* x4z))) .* (((x1x + (-1) .* x3x) .* ((x1x + (-1) .*  ...
  x3x) .^ 2 + (x1y + (-1) .* x3y) .^ 2 + (x1z + (-1) .* x3z) .^ 2)  ...
  .^ (-1 / 2) + (x2x + (-1) .* x4x) .* ((x2x + (-1) .* x4x) .^ 2 + ( ...
  x2y + (-1) .* x4y) .^ 2 + (x2z + (-1) .* x4z) .^ 2) .^ (-1 / 2))  ...
  .^ 2 + ((x1y + (-1) .* x3y) .* ((x1x + (-1) .* x3x) .^ 2 + (x1y +  ...
  (-1) .* x3y) .^ 2 + (x1z + (-1) .* x3z) .^ 2) .^ (-1 / 2) + (x2y + ...
   (-1) .* x4y) .* ((x2x + (-1) .* x4x) .^ 2 + (x2y + (-1) .* x4y)  ...
  .^ 2 + (x2z + (-1) .* x4z) .^ 2) .^ (-1 / 2)) .^ 2 + (((x1x + (-1) ...
   .* x3x) .^ 2 + (x1y + (-1) .* x3y) .^ 2 + (x1z + (-1) .* x3z) .^  ...
  2) .^ (-1 / 2) .* (x1z + (-1) .* x3z) + ((x2x + (-1) .* x4x) .^ 2  ...
  + (x2y + (-1) .* x4y) .^ 2 + (x2z + (-1) .* x4z) .^ 2) .^ (-1 / 2) ...
   .* (x2z + (-1) .* x4z)) .^ 2) .^ (-3 / 2) .* ((x1y + (-1) .* x3y) ...
   .* ((x1x + (-1) .* x3x) .^ 2 + (x1y + (-1) .* x3y) .^ 2 + (x1z +  ...
  (-1) .* x3z) .^ 2) .^ (-1 / 2) + (x2y + (-1) .* x4y) .* ((x2x + ( ...
  -1) .* x4x) .^ 2 + (x2y + (-1) .* x4y) .^ 2 + (x2z + (-1) .* x4z)  ...
  .^ 2) .^ (-1 / 2)) + (-1) .* (x2x + (-1) .* x4x) .* ((((-1) .*  ...
  x1y + x3y) .* (x2x + (-1) .* x4x) + (x1x + (-1) .* x3x) .* (x2y +  ...
  (-1) .* x4y)) .^ 2 + ((x1z + (-1) .* x3z) .* (x2x + (-1) .* x4x) + ...
   (-1) .* (x1x + (-1) .* x3x) .* (x2z + (-1) .* x4z)) .^ 2 + (((-1) ...
   .* x1z + x3z) .* (x2y + (-1) .* x4y) + (x1y + (-1) .* x3y) .* ( ...
  x2z + (-1) .* x4z)) .^ 2) .^ (-1 / 2) .* (((x1x + (-1) .* x3x) .*  ...
  ((x1x + (-1) .* x3x) .^ 2 + (x1y + (-1) .* x3y) .^ 2 + (x1z + (-1) ...
   .* x3z) .^ 2) .^ (-1 / 2) + (x2x + (-1) .* x4x) .* ((x2x + (-1)  ...
  .* x4x) .^ 2 + (x2y + (-1) .* x4y) .^ 2 + (x2z + (-1) .* x4z) .^  ...
  2) .^ (-1 / 2)) .^ 2 + ((x1y + (-1) .* x3y) .* ((x1x + (-1) .*  ...
  x3x) .^ 2 + (x1y + (-1) .* x3y) .^ 2 + (x1z + (-1) .* x3z) .^ 2)  ...
  .^ (-1 / 2) + (x2y + (-1) .* x4y) .* ((x2x + (-1) .* x4x) .^ 2 + ( ...
  x2y + (-1) .* x4y) .^ 2 + (x2z + (-1) .* x4z) .^ 2) .^ (-1 / 2))  ...
  .^ 2 + (((x1x + (-1) .* x3x) .^ 2 + (x1y + (-1) .* x3y) .^ 2 + ( ...
  x1z + (-1) .* x3z) .^ 2) .^ (-1 / 2) .* (x1z + (-1) .* x3z) + (( ...
  x2x + (-1) .* x4x) .^ 2 + (x2y + (-1) .* x4y) .^ 2 + (x2z + (-1)  ...
  .* x4z) .^ 2) .^ (-1 / 2) .* (x2z + (-1) .* x4z)) .^ 2) .^ (-1 /  ...
  2) .* ((x1y + (-1) .* x3y) .* ((x1x + (-1) .* x3x) .^ 2 + (x1y + ( ...
  -1) .* x3y) .^ 2 + (x1z + (-1) .* x3z) .^ 2) .^ (-1 / 2) + (x2y +  ...
  (-1) .* x4y) .* ((x2x + (-1) .* x4x) .^ 2 + (x2y + (-1) .* x4y)  ...
  .^ 2 + (x2z + (-1) .* x4z) .^ 2) .^ (-1 / 2)) + (x1y + (-1) .*  ...
  x3y) .* ((x1x + (-1) .* x3x) .^ 2 + (x1y + (-1) .* x3y) .^ 2 + ( ...
  x1z + (-1) .* x3z) .^ 2) .^ (-3 / 2) .* (x1z + (-1) .* x3z) .* ((( ...
  (-1) .* x1y + x3y) .* (x2x + (-1) .* x4x) + (x1x + (-1) .* x3x) .* ...
   (x2y + (-1) .* x4y)) .^ 2 + ((x1z + (-1) .* x3z) .* (x2x + (-1)  ...
  .* x4x) + (-1) .* (x1x + (-1) .* x3x) .* (x2z + (-1) .* x4z)) .^  ...
  2 + (((-1) .* x1z + x3z) .* (x2y + (-1) .* x4y) + (x1y + (-1) .*  ...
  x3y) .* (x2z + (-1) .* x4z)) .^ 2) .^ (-1 / 2) .* (((x1x + (-1) .* ...
   x3x) .* ((x1x + (-1) .* x3x) .^ 2 + (x1y + (-1) .* x3y) .^ 2 + ( ...
  x1z + (-1) .* x3z) .^ 2) .^ (-1 / 2) + (x2x + (-1) .* x4x) .* (( ...
  x2x + (-1) .* x4x) .^ 2 + (x2y + (-1) .* x4y) .^ 2 + (x2z + (-1)  ...
  .* x4z) .^ 2) .^ (-1 / 2)) .^ 2 + ((x1y + (-1) .* x3y) .* ((x1x +  ...
  (-1) .* x3x) .^ 2 + (x1y + (-1) .* x3y) .^ 2 + (x1z + (-1) .* x3z) ...
   .^ 2) .^ (-1 / 2) + (x2y + (-1) .* x4y) .* ((x2x + (-1) .* x4x)  ...
  .^ 2 + (x2y + (-1) .* x4y) .^ 2 + (x2z + (-1) .* x4z) .^ 2) .^ ( ...
  -1 / 2)) .^ 2 + (((x1x + (-1) .* x3x) .^ 2 + (x1y + (-1) .* x3y)  ...
  .^ 2 + (x1z + (-1) .* x3z) .^ 2) .^ (-1 / 2) .* (x1z + (-1) .*  ...
  x3z) + ((x2x + (-1) .* x4x) .^ 2 + (x2y + (-1) .* x4y) .^ 2 + ( ...
  x2z + (-1) .* x4z) .^ 2) .^ (-1 / 2) .* (x2z + (-1) .* x4z)) .^ 2) ...
   .^ (-1 / 2) .* ((x1z + (-1) .* x3z) .* (x2x + (-1) .* x4x) + (-1) ...
   .* (x1x + (-1) .* x3x) .* (x2z + (-1) .* x4z)) + (-1 / 2) .* (((( ...
  -1) .* x1y + x3y) .* (x2x + (-1) .* x4x) + (x1x + (-1) .* x3x) .*  ...
  (x2y + (-1) .* x4y)) .^ 2 + ((x1z + (-1) .* x3z) .* (x2x + (-1) .* ...
   x4x) + (-1) .* (x1x + (-1) .* x3x) .* (x2z + (-1) .* x4z)) .^ 2 + ...
   (((-1) .* x1z + x3z) .* (x2y + (-1) .* x4y) + (x1y + (-1) .* x3y) ...
   .* (x2z + (-1) .* x4z)) .^ 2) .^ (-1 / 2) .* (2 .* (x1x + (-1) .* ...
   x3x) .* (x1y + (-1) .* x3y) .* ((x1x + (-1) .* x3x) .^ 2 + (x1y + ...
   (-1) .* x3y) .^ 2 + (x1z + (-1) .* x3z) .^ 2) .^ (-3 / 2) .* (( ...
  x1x + (-1) .* x3x) .* ((x1x + (-1) .* x3x) .^ 2 + (x1y + (-1) .*  ...
  x3y) .^ 2 + (x1z + (-1) .* x3z) .^ 2) .^ (-1 / 2) + (x2x + (-1) .* ...
   x4x) .* ((x2x + (-1) .* x4x) .^ 2 + (x2y + (-1) .* x4y) .^ 2 + ( ...
  x2z + (-1) .* x4z) .^ 2) .^ (-1 / 2)) + 2 .* ((x1y + (-1) .* x3y)  ...
  .^ 2 .* ((x1x + (-1) .* x3x) .^ 2 + (x1y + (-1) .* x3y) .^ 2 + ( ...
  x1z + (-1) .* x3z) .^ 2) .^ (-3 / 2) + (-1) .* ((x1x + (-1) .*  ...
  x3x) .^ 2 + (x1y + (-1) .* x3y) .^ 2 + (x1z + (-1) .* x3z) .^ 2)  ...
  .^ (-1 / 2)) .* ((x1y + (-1) .* x3y) .* ((x1x + (-1) .* x3x) .^ 2  ...
  + (x1y + (-1) .* x3y) .^ 2 + (x1z + (-1) .* x3z) .^ 2) .^ (-1 / 2) ...
   + (x2y + (-1) .* x4y) .* ((x2x + (-1) .* x4x) .^ 2 + (x2y + (-1)  ...
  .* x4y) .^ 2 + (x2z + (-1) .* x4z) .^ 2) .^ (-1 / 2)) + 2 .* (x1y  ...
  + (-1) .* x3y) .* ((x1x + (-1) .* x3x) .^ 2 + (x1y + (-1) .* x3y)  ...
  .^ 2 + (x1z + (-1) .* x3z) .^ 2) .^ (-3 / 2) .* (x1z + (-1) .*  ...
  x3z) .* (((x1x + (-1) .* x3x) .^ 2 + (x1y + (-1) .* x3y) .^ 2 + ( ...
  x1z + (-1) .* x3z) .^ 2) .^ (-1 / 2) .* (x1z + (-1) .* x3z) + (( ...
  x2x + (-1) .* x4x) .^ 2 + (x2y + (-1) .* x4y) .^ 2 + (x2z + (-1)  ...
  .* x4z) .^ 2) .^ (-1 / 2) .* (x2z + (-1) .* x4z))) .* (((x1x + ( ...
  -1) .* x3x) .* ((x1x + (-1) .* x3x) .^ 2 + (x1y + (-1) .* x3y) .^  ...
  2 + (x1z + (-1) .* x3z) .^ 2) .^ (-1 / 2) + (x2x + (-1) .* x4x) .* ...
   ((x2x + (-1) .* x4x) .^ 2 + (x2y + (-1) .* x4y) .^ 2 + (x2z + ( ...
  -1) .* x4z) .^ 2) .^ (-1 / 2)) .^ 2 + ((x1y + (-1) .* x3y) .* (( ...
  x1x + (-1) .* x3x) .^ 2 + (x1y + (-1) .* x3y) .^ 2 + (x1z + (-1)  ...
  .* x3z) .^ 2) .^ (-1 / 2) + (x2y + (-1) .* x4y) .* ((x2x + (-1) .* ...
   x4x) .^ 2 + (x2y + (-1) .* x4y) .^ 2 + (x2z + (-1) .* x4z) .^ 2)  ...
  .^ (-1 / 2)) .^ 2 + (((x1x + (-1) .* x3x) .^ 2 + (x1y + (-1) .*  ...
  x3y) .^ 2 + (x1z + (-1) .* x3z) .^ 2) .^ (-1 / 2) .* (x1z + (-1)  ...
  .* x3z) + ((x2x + (-1) .* x4x) .^ 2 + (x2y + (-1) .* x4y) .^ 2 + ( ...
  x2z + (-1) .* x4z) .^ 2) .^ (-1 / 2) .* (x2z + (-1) .* x4z)) .^ 2) ...
   .^ (-3 / 2) .* ((x1z + (-1) .* x3z) .* (x2x + (-1) .* x4x) + (-1) ...
   .* (x1x + (-1) .* x3x) .* (x2z + (-1) .* x4z)) .* (((x1x + (-1)  ...
  .* x3x) .^ 2 + (x1y + (-1) .* x3y) .^ 2 + (x1z + (-1) .* x3z) .^  ...
  2) .^ (-1 / 2) .* (x1z + (-1) .* x3z) + ((x2x + (-1) .* x4x) .^ 2  ...
  + (x2y + (-1) .* x4y) .^ 2 + (x2z + (-1) .* x4z) .^ 2) .^ (-1 / 2) ...
   .* (x2z + (-1) .* x4z)) + (1 / 2) .* (((-1) .* x1y + x3y) .* ( ...
  x2x + (-1) .* x4x) + (x1x + (-1) .* x3x) .* (x2y + (-1) .* x4y))  ...
  .* ((((-1) .* x1y + x3y) .* (x2x + (-1) .* x4x) + (x1x + (-1) .*  ...
  x3x) .* (x2y + (-1) .* x4y)) .^ 2 + ((x1z + (-1) .* x3z) .* (x2x + ...
   (-1) .* x4x) + (-1) .* (x1x + (-1) .* x3x) .* (x2z + (-1) .* x4z) ...
  ) .^ 2 + (((-1) .* x1z + x3z) .* (x2y + (-1) .* x4y) + (x1y + (-1) ...
   .* x3y) .* (x2z + (-1) .* x4z)) .^ 2) .^ (-3 / 2) .* (((x1x + ( ...
  -1) .* x3x) .* ((x1x + (-1) .* x3x) .^ 2 + (x1y + (-1) .* x3y) .^  ...
  2 + (x1z + (-1) .* x3z) .^ 2) .^ (-1 / 2) + (x2x + (-1) .* x4x) .* ...
   ((x2x + (-1) .* x4x) .^ 2 + (x2y + (-1) .* x4y) .^ 2 + (x2z + ( ...
  -1) .* x4z) .^ 2) .^ (-1 / 2)) .^ 2 + ((x1y + (-1) .* x3y) .* (( ...
  x1x + (-1) .* x3x) .^ 2 + (x1y + (-1) .* x3y) .^ 2 + (x1z + (-1)  ...
  .* x3z) .^ 2) .^ (-1 / 2) + (x2y + (-1) .* x4y) .* ((x2x + (-1) .* ...
   x4x) .^ 2 + (x2y + (-1) .* x4y) .^ 2 + (x2z + (-1) .* x4z) .^ 2)  ...
  .^ (-1 / 2)) .^ 2 + (((x1x + (-1) .* x3x) .^ 2 + (x1y + (-1) .*  ...
  x3y) .^ 2 + (x1z + (-1) .* x3z) .^ 2) .^ (-1 / 2) .* (x1z + (-1)  ...
  .* x3z) + ((x2x + (-1) .* x4x) .^ 2 + (x2y + (-1) .* x4y) .^ 2 + ( ...
  x2z + (-1) .* x4z) .^ 2) .^ (-1 / 2) .* (x2z + (-1) .* x4z)) .^ 2) ...
   .^ (-1 / 2) .* ((x1y + (-1) .* x3y) .* ((x1x + (-1) .* x3x) .^ 2  ...
  + (x1y + (-1) .* x3y) .^ 2 + (x1z + (-1) .* x3z) .^ 2) .^ (-1 / 2) ...
   + (x2y + (-1) .* x4y) .* ((x2x + (-1) .* x4x) .^ 2 + (x2y + (-1)  ...
  .* x4y) .^ 2 + (x2z + (-1) .* x4z) .^ 2) .^ (-1 / 2)) .* (2 .* ( ...
  x2x + (-1) .* x4x) .* (((-1) .* x1y + x3y) .* (x2x + (-1) .* x4x)  ...
  + (x1x + (-1) .* x3x) .* (x2y + (-1) .* x4y)) + 2 .* (((-1) .*  ...
  x1z + x3z) .* (x2y + (-1) .* x4y) + (x1y + (-1) .* x3y) .* (x2z +  ...
  (-1) .* x4z)) .* ((-1) .* x2z + x4z)) + (-1 / 2) .* ((((-1) .*  ...
  x1y + x3y) .* (x2x + (-1) .* x4x) + (x1x + (-1) .* x3x) .* (x2y +  ...
  (-1) .* x4y)) .^ 2 + ((x1z + (-1) .* x3z) .* (x2x + (-1) .* x4x) + ...
   (-1) .* (x1x + (-1) .* x3x) .* (x2z + (-1) .* x4z)) .^ 2 + (((-1) ...
   .* x1z + x3z) .* (x2y + (-1) .* x4y) + (x1y + (-1) .* x3y) .* ( ...
  x2z + (-1) .* x4z)) .^ 2) .^ (-3 / 2) .* (((x1x + (-1) .* x3x) .*  ...
  ((x1x + (-1) .* x3x) .^ 2 + (x1y + (-1) .* x3y) .^ 2 + (x1z + (-1) ...
   .* x3z) .^ 2) .^ (-1 / 2) + (x2x + (-1) .* x4x) .* ((x2x + (-1)  ...
  .* x4x) .^ 2 + (x2y + (-1) .* x4y) .^ 2 + (x2z + (-1) .* x4z) .^  ...
  2) .^ (-1 / 2)) .^ 2 + ((x1y + (-1) .* x3y) .* ((x1x + (-1) .*  ...
  x3x) .^ 2 + (x1y + (-1) .* x3y) .^ 2 + (x1z + (-1) .* x3z) .^ 2)  ...
  .^ (-1 / 2) + (x2y + (-1) .* x4y) .* ((x2x + (-1) .* x4x) .^ 2 + ( ...
  x2y + (-1) .* x4y) .^ 2 + (x2z + (-1) .* x4z) .^ 2) .^ (-1 / 2))  ...
  .^ 2 + (((x1x + (-1) .* x3x) .^ 2 + (x1y + (-1) .* x3y) .^ 2 + ( ...
  x1z + (-1) .* x3z) .^ 2) .^ (-1 / 2) .* (x1z + (-1) .* x3z) + (( ...
  x2x + (-1) .* x4x) .^ 2 + (x2y + (-1) .* x4y) .^ 2 + (x2z + (-1)  ...
  .* x4z) .^ 2) .^ (-1 / 2) .* (x2z + (-1) .* x4z)) .^ 2) .^ (-1 /  ...
  2) .* ((x1z + (-1) .* x3z) .* (x2x + (-1) .* x4x) + (-1) .* (x1x + ...
   (-1) .* x3x) .* (x2z + (-1) .* x4z)) .* (((x1x + (-1) .* x3x) .^  ...
  2 + (x1y + (-1) .* x3y) .^ 2 + (x1z + (-1) .* x3z) .^ 2) .^ (-1 /  ...
  2) .* (x1z + (-1) .* x3z) + ((x2x + (-1) .* x4x) .^ 2 + (x2y + ( ...
  -1) .* x4y) .^ 2 + (x2z + (-1) .* x4z) .^ 2) .^ (-1 / 2) .* (x2z + ...
   (-1) .* x4z)) .* (2 .* (x2x + (-1) .* x4x) .* (((-1) .* x1y +  ...
  x3y) .* (x2x + (-1) .* x4x) + (x1x + (-1) .* x3x) .* (x2y + (-1)  ...
  .* x4y)) + 2 .* (((-1) .* x1z + x3z) .* (x2y + (-1) .* x4y) + ( ...
  x1y + (-1) .* x3y) .* (x2z + (-1) .* x4z)) .* ((-1) .* x2z + x4z)) ...
  ,(-1) .* (x1y + (-1) .* x3y) .* ((x1x + (-1) .* x3x) .^ 2 + (x1y + ...
   (-1) .* x3y) .^ 2 + (x1z + (-1) .* x3z) .^ 2) .^ (-3 / 2) .* ( ...
  x1z + (-1) .* x3z) .* (((-1) .* x1y + x3y) .* (x2x + (-1) .* x4x)  ...
  + (x1x + (-1) .* x3x) .* (x2y + (-1) .* x4y)) .* ((((-1) .* x1y +  ...
  x3y) .* (x2x + (-1) .* x4x) + (x1x + (-1) .* x3x) .* (x2y + (-1)  ...
  .* x4y)) .^ 2 + ((x1z + (-1) .* x3z) .* (x2x + (-1) .* x4x) + (-1) ...
   .* (x1x + (-1) .* x3x) .* (x2z + (-1) .* x4z)) .^ 2 + (((-1) .*  ...
  x1z + x3z) .* (x2y + (-1) .* x4y) + (x1y + (-1) .* x3y) .* (x2z +  ...
  (-1) .* x4z)) .^ 2) .^ (-1 / 2) .* (((x1x + (-1) .* x3x) .* ((x1x  ...
  + (-1) .* x3x) .^ 2 + (x1y + (-1) .* x3y) .^ 2 + (x1z + (-1) .*  ...
  x3z) .^ 2) .^ (-1 / 2) + (x2x + (-1) .* x4x) .* ((x2x + (-1) .*  ...
  x4x) .^ 2 + (x2y + (-1) .* x4y) .^ 2 + (x2z + (-1) .* x4z) .^ 2)  ...
  .^ (-1 / 2)) .^ 2 + ((x1y + (-1) .* x3y) .* ((x1x + (-1) .* x3x)  ...
  .^ 2 + (x1y + (-1) .* x3y) .^ 2 + (x1z + (-1) .* x3z) .^ 2) .^ ( ...
  -1 / 2) + (x2y + (-1) .* x4y) .* ((x2x + (-1) .* x4x) .^ 2 + (x2y  ...
  + (-1) .* x4y) .^ 2 + (x2z + (-1) .* x4z) .^ 2) .^ (-1 / 2)) .^ 2  ...
  + (((x1x + (-1) .* x3x) .^ 2 + (x1y + (-1) .* x3y) .^ 2 + (x1z + ( ...
  -1) .* x3z) .^ 2) .^ (-1 / 2) .* (x1z + (-1) .* x3z) + ((x2x + ( ...
  -1) .* x4x) .^ 2 + (x2y + (-1) .* x4y) .^ 2 + (x2z + (-1) .* x4z)  ...
  .^ 2) .^ (-1 / 2) .* (x2z + (-1) .* x4z)) .^ 2) .^ (-1 / 2) + (1  ...
  / 2) .* (((-1) .* x1y + x3y) .* (x2x + (-1) .* x4x) + (x1x + (-1)  ...
  .* x3x) .* (x2y + (-1) .* x4y)) .* ((((-1) .* x1y + x3y) .* (x2x + ...
   (-1) .* x4x) + (x1x + (-1) .* x3x) .* (x2y + (-1) .* x4y)) .^ 2 + ...
   ((x1z + (-1) .* x3z) .* (x2x + (-1) .* x4x) + (-1) .* (x1x + (-1) ...
   .* x3x) .* (x2z + (-1) .* x4z)) .^ 2 + (((-1) .* x1z + x3z) .* ( ...
  x2y + (-1) .* x4y) + (x1y + (-1) .* x3y) .* (x2z + (-1) .* x4z))  ...
  .^ 2) .^ (-1 / 2) .* (2 .* (x1x + (-1) .* x3x) .* ((x1x + (-1) .*  ...
  x3x) .^ 2 + (x1y + (-1) .* x3y) .^ 2 + (x1z + (-1) .* x3z) .^ 2)  ...
  .^ (-3 / 2) .* (x1z + (-1) .* x3z) .* ((x1x + (-1) .* x3x) .* (( ...
  x1x + (-1) .* x3x) .^ 2 + (x1y + (-1) .* x3y) .^ 2 + (x1z + (-1)  ...
  .* x3z) .^ 2) .^ (-1 / 2) + (x2x + (-1) .* x4x) .* ((x2x + (-1) .* ...
   x4x) .^ 2 + (x2y + (-1) .* x4y) .^ 2 + (x2z + (-1) .* x4z) .^ 2)  ...
  .^ (-1 / 2)) + 2 .* (x1y + (-1) .* x3y) .* ((x1x + (-1) .* x3x)  ...
  .^ 2 + (x1y + (-1) .* x3y) .^ 2 + (x1z + (-1) .* x3z) .^ 2) .^ ( ...
  -3 / 2) .* (x1z + (-1) .* x3z) .* ((x1y + (-1) .* x3y) .* ((x1x +  ...
  (-1) .* x3x) .^ 2 + (x1y + (-1) .* x3y) .^ 2 + (x1z + (-1) .* x3z) ...
   .^ 2) .^ (-1 / 2) + (x2y + (-1) .* x4y) .* ((x2x + (-1) .* x4x)  ...
  .^ 2 + (x2y + (-1) .* x4y) .^ 2 + (x2z + (-1) .* x4z) .^ 2) .^ ( ...
  -1 / 2)) + 2 .* ((-1) .* ((x1x + (-1) .* x3x) .^ 2 + (x1y + (-1)  ...
  .* x3y) .^ 2 + (x1z + (-1) .* x3z) .^ 2) .^ (-1 / 2) + ((x1x + ( ...
  -1) .* x3x) .^ 2 + (x1y + (-1) .* x3y) .^ 2 + (x1z + (-1) .* x3z)  ...
  .^ 2) .^ (-3 / 2) .* (x1z + (-1) .* x3z) .^ 2) .* (((x1x + (-1) .* ...
   x3x) .^ 2 + (x1y + (-1) .* x3y) .^ 2 + (x1z + (-1) .* x3z) .^ 2)  ...
  .^ (-1 / 2) .* (x1z + (-1) .* x3z) + ((x2x + (-1) .* x4x) .^ 2 + ( ...
  x2y + (-1) .* x4y) .^ 2 + (x2z + (-1) .* x4z) .^ 2) .^ (-1 / 2) .* ...
   (x2z + (-1) .* x4z))) .* (((x1x + (-1) .* x3x) .* ((x1x + (-1) .* ...
   x3x) .^ 2 + (x1y + (-1) .* x3y) .^ 2 + (x1z + (-1) .* x3z) .^ 2)  ...
  .^ (-1 / 2) + (x2x + (-1) .* x4x) .* ((x2x + (-1) .* x4x) .^ 2 + ( ...
  x2y + (-1) .* x4y) .^ 2 + (x2z + (-1) .* x4z) .^ 2) .^ (-1 / 2))  ...
  .^ 2 + ((x1y + (-1) .* x3y) .* ((x1x + (-1) .* x3x) .^ 2 + (x1y +  ...
  (-1) .* x3y) .^ 2 + (x1z + (-1) .* x3z) .^ 2) .^ (-1 / 2) + (x2y + ...
   (-1) .* x4y) .* ((x2x + (-1) .* x4x) .^ 2 + (x2y + (-1) .* x4y)  ...
  .^ 2 + (x2z + (-1) .* x4z) .^ 2) .^ (-1 / 2)) .^ 2 + (((x1x + (-1) ...
   .* x3x) .^ 2 + (x1y + (-1) .* x3y) .^ 2 + (x1z + (-1) .* x3z) .^  ...
  2) .^ (-1 / 2) .* (x1z + (-1) .* x3z) + ((x2x + (-1) .* x4x) .^ 2  ...
  + (x2y + (-1) .* x4y) .^ 2 + (x2z + (-1) .* x4z) .^ 2) .^ (-1 / 2) ...
   .* (x2z + (-1) .* x4z)) .^ 2) .^ (-3 / 2) .* ((x1y + (-1) .* x3y) ...
   .* ((x1x + (-1) .* x3x) .^ 2 + (x1y + (-1) .* x3y) .^ 2 + (x1z +  ...
  (-1) .* x3z) .^ 2) .^ (-1 / 2) + (x2y + (-1) .* x4y) .* ((x2x + ( ...
  -1) .* x4x) .^ 2 + (x2y + (-1) .* x4y) .^ 2 + (x2z + (-1) .* x4z)  ...
  .^ 2) .^ (-1 / 2)) + (1 / 2) .* (((-1) .* x1y + x3y) .* (x2x + ( ...
  -1) .* x4x) + (x1x + (-1) .* x3x) .* (x2y + (-1) .* x4y)) .* (2 .* ...
   ((-1) .* x2x + x4x) .* ((x1z + (-1) .* x3z) .* (x2x + (-1) .*  ...
  x4x) + (-1) .* (x1x + (-1) .* x3x) .* (x2z + (-1) .* x4z)) + 2 .*  ...
  (x2y + (-1) .* x4y) .* (((-1) .* x1z + x3z) .* (x2y + (-1) .* x4y) ...
   + (x1y + (-1) .* x3y) .* (x2z + (-1) .* x4z))) .* ((((-1) .* x1y  ...
  + x3y) .* (x2x + (-1) .* x4x) + (x1x + (-1) .* x3x) .* (x2y + (-1) ...
   .* x4y)) .^ 2 + ((x1z + (-1) .* x3z) .* (x2x + (-1) .* x4x) + ( ...
  -1) .* (x1x + (-1) .* x3x) .* (x2z + (-1) .* x4z)) .^ 2 + (((-1)  ...
  .* x1z + x3z) .* (x2y + (-1) .* x4y) + (x1y + (-1) .* x3y) .* ( ...
  x2z + (-1) .* x4z)) .^ 2) .^ (-3 / 2) .* (((x1x + (-1) .* x3x) .*  ...
  ((x1x + (-1) .* x3x) .^ 2 + (x1y + (-1) .* x3y) .^ 2 + (x1z + (-1) ...
   .* x3z) .^ 2) .^ (-1 / 2) + (x2x + (-1) .* x4x) .* ((x2x + (-1)  ...
  .* x4x) .^ 2 + (x2y + (-1) .* x4y) .^ 2 + (x2z + (-1) .* x4z) .^  ...
  2) .^ (-1 / 2)) .^ 2 + ((x1y + (-1) .* x3y) .* ((x1x + (-1) .*  ...
  x3x) .^ 2 + (x1y + (-1) .* x3y) .^ 2 + (x1z + (-1) .* x3z) .^ 2)  ...
  .^ (-1 / 2) + (x2y + (-1) .* x4y) .* ((x2x + (-1) .* x4x) .^ 2 + ( ...
  x2y + (-1) .* x4y) .^ 2 + (x2z + (-1) .* x4z) .^ 2) .^ (-1 / 2))  ...
  .^ 2 + (((x1x + (-1) .* x3x) .^ 2 + (x1y + (-1) .* x3y) .^ 2 + ( ...
  x1z + (-1) .* x3z) .^ 2) .^ (-1 / 2) .* (x1z + (-1) .* x3z) + (( ...
  x2x + (-1) .* x4x) .^ 2 + (x2y + (-1) .* x4y) .^ 2 + (x2z + (-1)  ...
  .* x4z) .^ 2) .^ (-1 / 2) .* (x2z + (-1) .* x4z)) .^ 2) .^ (-1 /  ...
  2) .* ((x1y + (-1) .* x3y) .* ((x1x + (-1) .* x3x) .^ 2 + (x1y + ( ...
  -1) .* x3y) .^ 2 + (x1z + (-1) .* x3z) .^ 2) .^ (-1 / 2) + (x2y +  ...
  (-1) .* x4y) .* ((x2x + (-1) .* x4x) .^ 2 + (x2y + (-1) .* x4y)  ...
  .^ 2 + (x2z + (-1) .* x4z) .^ 2) .^ (-1 / 2)) + ((-1) .* ((x1x + ( ...
  -1) .* x3x) .^ 2 + (x1y + (-1) .* x3y) .^ 2 + (x1z + (-1) .* x3z)  ...
  .^ 2) .^ (-1 / 2) + ((x1x + (-1) .* x3x) .^ 2 + (x1y + (-1) .*  ...
  x3y) .^ 2 + (x1z + (-1) .* x3z) .^ 2) .^ (-3 / 2) .* (x1z + (-1)  ...
  .* x3z) .^ 2) .* ((((-1) .* x1y + x3y) .* (x2x + (-1) .* x4x) + ( ...
  x1x + (-1) .* x3x) .* (x2y + (-1) .* x4y)) .^ 2 + ((x1z + (-1) .*  ...
  x3z) .* (x2x + (-1) .* x4x) + (-1) .* (x1x + (-1) .* x3x) .* (x2z  ...
  + (-1) .* x4z)) .^ 2 + (((-1) .* x1z + x3z) .* (x2y + (-1) .* x4y) ...
   + (x1y + (-1) .* x3y) .* (x2z + (-1) .* x4z)) .^ 2) .^ (-1 / 2)  ...
  .* (((x1x + (-1) .* x3x) .* ((x1x + (-1) .* x3x) .^ 2 + (x1y + ( ...
  -1) .* x3y) .^ 2 + (x1z + (-1) .* x3z) .^ 2) .^ (-1 / 2) + (x2x +  ...
  (-1) .* x4x) .* ((x2x + (-1) .* x4x) .^ 2 + (x2y + (-1) .* x4y)  ...
  .^ 2 + (x2z + (-1) .* x4z) .^ 2) .^ (-1 / 2)) .^ 2 + ((x1y + (-1)  ...
  .* x3y) .* ((x1x + (-1) .* x3x) .^ 2 + (x1y + (-1) .* x3y) .^ 2 +  ...
  (x1z + (-1) .* x3z) .^ 2) .^ (-1 / 2) + (x2y + (-1) .* x4y) .* (( ...
  x2x + (-1) .* x4x) .^ 2 + (x2y + (-1) .* x4y) .^ 2 + (x2z + (-1)  ...
  .* x4z) .^ 2) .^ (-1 / 2)) .^ 2 + (((x1x + (-1) .* x3x) .^ 2 + ( ...
  x1y + (-1) .* x3y) .^ 2 + (x1z + (-1) .* x3z) .^ 2) .^ (-1 / 2) .* ...
   (x1z + (-1) .* x3z) + ((x2x + (-1) .* x4x) .^ 2 + (x2y + (-1) .*  ...
  x4y) .^ 2 + (x2z + (-1) .* x4z) .^ 2) .^ (-1 / 2) .* (x2z + (-1)  ...
  .* x4z)) .^ 2) .^ (-1 / 2) .* ((x1z + (-1) .* x3z) .* (x2x + (-1)  ...
  .* x4x) + (-1) .* (x1x + (-1) .* x3x) .* (x2z + (-1) .* x4z)) + (( ...
  -1) .* x2x + x4x) .* ((((-1) .* x1y + x3y) .* (x2x + (-1) .* x4x)  ...
  + (x1x + (-1) .* x3x) .* (x2y + (-1) .* x4y)) .^ 2 + ((x1z + (-1)  ...
  .* x3z) .* (x2x + (-1) .* x4x) + (-1) .* (x1x + (-1) .* x3x) .* ( ...
  x2z + (-1) .* x4z)) .^ 2 + (((-1) .* x1z + x3z) .* (x2y + (-1) .*  ...
  x4y) + (x1y + (-1) .* x3y) .* (x2z + (-1) .* x4z)) .^ 2) .^ (-1 /  ...
  2) .* (((x1x + (-1) .* x3x) .* ((x1x + (-1) .* x3x) .^ 2 + (x1y +  ...
  (-1) .* x3y) .^ 2 + (x1z + (-1) .* x3z) .^ 2) .^ (-1 / 2) + (x2x + ...
   (-1) .* x4x) .* ((x2x + (-1) .* x4x) .^ 2 + (x2y + (-1) .* x4y)  ...
  .^ 2 + (x2z + (-1) .* x4z) .^ 2) .^ (-1 / 2)) .^ 2 + ((x1y + (-1)  ...
  .* x3y) .* ((x1x + (-1) .* x3x) .^ 2 + (x1y + (-1) .* x3y) .^ 2 +  ...
  (x1z + (-1) .* x3z) .^ 2) .^ (-1 / 2) + (x2y + (-1) .* x4y) .* (( ...
  x2x + (-1) .* x4x) .^ 2 + (x2y + (-1) .* x4y) .^ 2 + (x2z + (-1)  ...
  .* x4z) .^ 2) .^ (-1 / 2)) .^ 2 + (((x1x + (-1) .* x3x) .^ 2 + ( ...
  x1y + (-1) .* x3y) .^ 2 + (x1z + (-1) .* x3z) .^ 2) .^ (-1 / 2) .* ...
   (x1z + (-1) .* x3z) + ((x2x + (-1) .* x4x) .^ 2 + (x2y + (-1) .*  ...
  x4y) .^ 2 + (x2z + (-1) .* x4z) .^ 2) .^ (-1 / 2) .* (x2z + (-1)  ...
  .* x4z)) .^ 2) .^ (-1 / 2) .* (((x1x + (-1) .* x3x) .^ 2 + (x1y +  ...
  (-1) .* x3y) .^ 2 + (x1z + (-1) .* x3z) .^ 2) .^ (-1 / 2) .* (x1z  ...
  + (-1) .* x3z) + ((x2x + (-1) .* x4x) .^ 2 + (x2y + (-1) .* x4y)  ...
  .^ 2 + (x2z + (-1) .* x4z) .^ 2) .^ (-1 / 2) .* (x2z + (-1) .*  ...
  x4z)) + (-1 / 2) .* ((((-1) .* x1y + x3y) .* (x2x + (-1) .* x4x) + ...
   (x1x + (-1) .* x3x) .* (x2y + (-1) .* x4y)) .^ 2 + ((x1z + (-1)  ...
  .* x3z) .* (x2x + (-1) .* x4x) + (-1) .* (x1x + (-1) .* x3x) .* ( ...
  x2z + (-1) .* x4z)) .^ 2 + (((-1) .* x1z + x3z) .* (x2y + (-1) .*  ...
  x4y) + (x1y + (-1) .* x3y) .* (x2z + (-1) .* x4z)) .^ 2) .^ (-1 /  ...
  2) .* (2 .* (x1x + (-1) .* x3x) .* ((x1x + (-1) .* x3x) .^ 2 + ( ...
  x1y + (-1) .* x3y) .^ 2 + (x1z + (-1) .* x3z) .^ 2) .^ (-3 / 2) .* ...
   (x1z + (-1) .* x3z) .* ((x1x + (-1) .* x3x) .* ((x1x + (-1) .*  ...
  x3x) .^ 2 + (x1y + (-1) .* x3y) .^ 2 + (x1z + (-1) .* x3z) .^ 2)  ...
  .^ (-1 / 2) + (x2x + (-1) .* x4x) .* ((x2x + (-1) .* x4x) .^ 2 + ( ...
  x2y + (-1) .* x4y) .^ 2 + (x2z + (-1) .* x4z) .^ 2) .^ (-1 / 2)) + ...
   2 .* (x1y + (-1) .* x3y) .* ((x1x + (-1) .* x3x) .^ 2 + (x1y + ( ...
  -1) .* x3y) .^ 2 + (x1z + (-1) .* x3z) .^ 2) .^ (-3 / 2) .* (x1z + ...
   (-1) .* x3z) .* ((x1y + (-1) .* x3y) .* ((x1x + (-1) .* x3x) .^  ...
  2 + (x1y + (-1) .* x3y) .^ 2 + (x1z + (-1) .* x3z) .^ 2) .^ (-1 /  ...
  2) + (x2y + (-1) .* x4y) .* ((x2x + (-1) .* x4x) .^ 2 + (x2y + ( ...
  -1) .* x4y) .^ 2 + (x2z + (-1) .* x4z) .^ 2) .^ (-1 / 2)) + 2 .* ( ...
  (-1) .* ((x1x + (-1) .* x3x) .^ 2 + (x1y + (-1) .* x3y) .^ 2 + ( ...
  x1z + (-1) .* x3z) .^ 2) .^ (-1 / 2) + ((x1x + (-1) .* x3x) .^ 2 + ...
   (x1y + (-1) .* x3y) .^ 2 + (x1z + (-1) .* x3z) .^ 2) .^ (-3 / 2)  ...
  .* (x1z + (-1) .* x3z) .^ 2) .* (((x1x + (-1) .* x3x) .^ 2 + (x1y  ...
  + (-1) .* x3y) .^ 2 + (x1z + (-1) .* x3z) .^ 2) .^ (-1 / 2) .* ( ...
  x1z + (-1) .* x3z) + ((x2x + (-1) .* x4x) .^ 2 + (x2y + (-1) .*  ...
  x4y) .^ 2 + (x2z + (-1) .* x4z) .^ 2) .^ (-1 / 2) .* (x2z + (-1)  ...
  .* x4z))) .* (((x1x + (-1) .* x3x) .* ((x1x + (-1) .* x3x) .^ 2 +  ...
  (x1y + (-1) .* x3y) .^ 2 + (x1z + (-1) .* x3z) .^ 2) .^ (-1 / 2) + ...
   (x2x + (-1) .* x4x) .* ((x2x + (-1) .* x4x) .^ 2 + (x2y + (-1) .* ...
   x4y) .^ 2 + (x2z + (-1) .* x4z) .^ 2) .^ (-1 / 2)) .^ 2 + ((x1y + ...
   (-1) .* x3y) .* ((x1x + (-1) .* x3x) .^ 2 + (x1y + (-1) .* x3y)  ...
  .^ 2 + (x1z + (-1) .* x3z) .^ 2) .^ (-1 / 2) + (x2y + (-1) .* x4y) ...
   .* ((x2x + (-1) .* x4x) .^ 2 + (x2y + (-1) .* x4y) .^ 2 + (x2z +  ...
  (-1) .* x4z) .^ 2) .^ (-1 / 2)) .^ 2 + (((x1x + (-1) .* x3x) .^ 2  ...
  + (x1y + (-1) .* x3y) .^ 2 + (x1z + (-1) .* x3z) .^ 2) .^ (-1 / 2) ...
   .* (x1z + (-1) .* x3z) + ((x2x + (-1) .* x4x) .^ 2 + (x2y + (-1)  ...
  .* x4y) .^ 2 + (x2z + (-1) .* x4z) .^ 2) .^ (-1 / 2) .* (x2z + ( ...
  -1) .* x4z)) .^ 2) .^ (-3 / 2) .* ((x1z + (-1) .* x3z) .* (x2x + ( ...
  -1) .* x4x) + (-1) .* (x1x + (-1) .* x3x) .* (x2z + (-1) .* x4z))  ...
  .* (((x1x + (-1) .* x3x) .^ 2 + (x1y + (-1) .* x3y) .^ 2 + (x1z +  ...
  (-1) .* x3z) .^ 2) .^ (-1 / 2) .* (x1z + (-1) .* x3z) + ((x2x + ( ...
  -1) .* x4x) .^ 2 + (x2y + (-1) .* x4y) .^ 2 + (x2z + (-1) .* x4z)  ...
  .^ 2) .^ (-1 / 2) .* (x2z + (-1) .* x4z)) + (-1 / 2) .* (2 .* (( ...
  -1) .* x2x + x4x) .* ((x1z + (-1) .* x3z) .* (x2x + (-1) .* x4x) + ...
   (-1) .* (x1x + (-1) .* x3x) .* (x2z + (-1) .* x4z)) + 2 .* (x2y + ...
   (-1) .* x4y) .* (((-1) .* x1z + x3z) .* (x2y + (-1) .* x4y) + ( ...
  x1y + (-1) .* x3y) .* (x2z + (-1) .* x4z))) .* ((((-1) .* x1y +  ...
  x3y) .* (x2x + (-1) .* x4x) + (x1x + (-1) .* x3x) .* (x2y + (-1)  ...
  .* x4y)) .^ 2 + ((x1z + (-1) .* x3z) .* (x2x + (-1) .* x4x) + (-1) ...
   .* (x1x + (-1) .* x3x) .* (x2z + (-1) .* x4z)) .^ 2 + (((-1) .*  ...
  x1z + x3z) .* (x2y + (-1) .* x4y) + (x1y + (-1) .* x3y) .* (x2z +  ...
  (-1) .* x4z)) .^ 2) .^ (-3 / 2) .* (((x1x + (-1) .* x3x) .* ((x1x  ...
  + (-1) .* x3x) .^ 2 + (x1y + (-1) .* x3y) .^ 2 + (x1z + (-1) .*  ...
  x3z) .^ 2) .^ (-1 / 2) + (x2x + (-1) .* x4x) .* ((x2x + (-1) .*  ...
  x4x) .^ 2 + (x2y + (-1) .* x4y) .^ 2 + (x2z + (-1) .* x4z) .^ 2)  ...
  .^ (-1 / 2)) .^ 2 + ((x1y + (-1) .* x3y) .* ((x1x + (-1) .* x3x)  ...
  .^ 2 + (x1y + (-1) .* x3y) .^ 2 + (x1z + (-1) .* x3z) .^ 2) .^ ( ...
  -1 / 2) + (x2y + (-1) .* x4y) .* ((x2x + (-1) .* x4x) .^ 2 + (x2y  ...
  + (-1) .* x4y) .^ 2 + (x2z + (-1) .* x4z) .^ 2) .^ (-1 / 2)) .^ 2  ...
  + (((x1x + (-1) .* x3x) .^ 2 + (x1y + (-1) .* x3y) .^ 2 + (x1z + ( ...
  -1) .* x3z) .^ 2) .^ (-1 / 2) .* (x1z + (-1) .* x3z) + ((x2x + ( ...
  -1) .* x4x) .^ 2 + (x2y + (-1) .* x4y) .^ 2 + (x2z + (-1) .* x4z)  ...
  .^ 2) .^ (-1 / 2) .* (x2z + (-1) .* x4z)) .^ 2) .^ (-1 / 2) .* (( ...
  x1z + (-1) .* x3z) .* (x2x + (-1) .* x4x) + (-1) .* (x1x + (-1) .* ...
   x3x) .* (x2z + (-1) .* x4z)) .* (((x1x + (-1) .* x3x) .^ 2 + ( ...
  x1y + (-1) .* x3y) .^ 2 + (x1z + (-1) .* x3z) .^ 2) .^ (-1 / 2) .* ...
   (x1z + (-1) .* x3z) + ((x2x + (-1) .* x4x) .^ 2 + (x2y + (-1) .*  ...
  x4y) .^ 2 + (x2z + (-1) .* x4z) .^ 2) .^ (-1 / 2) .* (x2z + (-1)  ...
  .* x4z)),(1 / 2) .* (((-1) .* x1y + x3y) .* (x2x + (-1) .* x4x) +  ...
  (x1x + (-1) .* x3x) .* (x2y + (-1) .* x4y)) .* (2 .* (x1y + (-1)  ...
  .* x3y) .* (((-1) .* x1y + x3y) .* (x2x + (-1) .* x4x) + (x1x + ( ...
  -1) .* x3x) .* (x2y + (-1) .* x4y)) + 2 .* ((-1) .* x1z + x3z) .*  ...
  ((x1z + (-1) .* x3z) .* (x2x + (-1) .* x4x) + (-1) .* (x1x + (-1)  ...
  .* x3x) .* (x2z + (-1) .* x4z))) .* ((((-1) .* x1y + x3y) .* (x2x  ...
  + (-1) .* x4x) + (x1x + (-1) .* x3x) .* (x2y + (-1) .* x4y)) .^ 2  ...
  + ((x1z + (-1) .* x3z) .* (x2x + (-1) .* x4x) + (-1) .* (x1x + ( ...
  -1) .* x3x) .* (x2z + (-1) .* x4z)) .^ 2 + (((-1) .* x1z + x3z) .* ...
   (x2y + (-1) .* x4y) + (x1y + (-1) .* x3y) .* (x2z + (-1) .* x4z)) ...
   .^ 2) .^ (-3 / 2) .* (((x1x + (-1) .* x3x) .* ((x1x + (-1) .*  ...
  x3x) .^ 2 + (x1y + (-1) .* x3y) .^ 2 + (x1z + (-1) .* x3z) .^ 2)  ...
  .^ (-1 / 2) + (x2x + (-1) .* x4x) .* ((x2x + (-1) .* x4x) .^ 2 + ( ...
  x2y + (-1) .* x4y) .^ 2 + (x2z + (-1) .* x4z) .^ 2) .^ (-1 / 2))  ...
  .^ 2 + ((x1y + (-1) .* x3y) .* ((x1x + (-1) .* x3x) .^ 2 + (x1y +  ...
  (-1) .* x3y) .^ 2 + (x1z + (-1) .* x3z) .^ 2) .^ (-1 / 2) + (x2y + ...
   (-1) .* x4y) .* ((x2x + (-1) .* x4x) .^ 2 + (x2y + (-1) .* x4y)  ...
  .^ 2 + (x2z + (-1) .* x4z) .^ 2) .^ (-1 / 2)) .^ 2 + (((x1x + (-1) ...
   .* x3x) .^ 2 + (x1y + (-1) .* x3y) .^ 2 + (x1z + (-1) .* x3z) .^  ...
  2) .^ (-1 / 2) .* (x1z + (-1) .* x3z) + ((x2x + (-1) .* x4x) .^ 2  ...
  + (x2y + (-1) .* x4y) .^ 2 + (x2z + (-1) .* x4z) .^ 2) .^ (-1 / 2) ...
   .* (x2z + (-1) .* x4z)) .^ 2) .^ (-1 / 2) .* ((x1y + (-1) .* x3y) ...
   .* ((x1x + (-1) .* x3x) .^ 2 + (x1y + (-1) .* x3y) .^ 2 + (x1z +  ...
  (-1) .* x3z) .^ 2) .^ (-1 / 2) + (x2y + (-1) .* x4y) .* ((x2x + ( ...
  -1) .* x4x) .^ 2 + (x2y + (-1) .* x4y) .^ 2 + (x2z + (-1) .* x4z)  ...
  .^ 2) .^ (-1 / 2)) + (-1) .* (x1y + (-1) .* x3y) .* ((((-1) .*  ...
  x1y + x3y) .* (x2x + (-1) .* x4x) + (x1x + (-1) .* x3x) .* (x2y +  ...
  (-1) .* x4y)) .^ 2 + ((x1z + (-1) .* x3z) .* (x2x + (-1) .* x4x) + ...
   (-1) .* (x1x + (-1) .* x3x) .* (x2z + (-1) .* x4z)) .^ 2 + (((-1) ...
   .* x1z + x3z) .* (x2y + (-1) .* x4y) + (x1y + (-1) .* x3y) .* ( ...
  x2z + (-1) .* x4z)) .^ 2) .^ (-1 / 2) .* (((x1x + (-1) .* x3x) .*  ...
  ((x1x + (-1) .* x3x) .^ 2 + (x1y + (-1) .* x3y) .^ 2 + (x1z + (-1) ...
   .* x3z) .^ 2) .^ (-1 / 2) + (x2x + (-1) .* x4x) .* ((x2x + (-1)  ...
  .* x4x) .^ 2 + (x2y + (-1) .* x4y) .^ 2 + (x2z + (-1) .* x4z) .^  ...
  2) .^ (-1 / 2)) .^ 2 + ((x1y + (-1) .* x3y) .* ((x1x + (-1) .*  ...
  x3x) .^ 2 + (x1y + (-1) .* x3y) .^ 2 + (x1z + (-1) .* x3z) .^ 2)  ...
  .^ (-1 / 2) + (x2y + (-1) .* x4y) .* ((x2x + (-1) .* x4x) .^ 2 + ( ...
  x2y + (-1) .* x4y) .^ 2 + (x2z + (-1) .* x4z) .^ 2) .^ (-1 / 2))  ...
  .^ 2 + (((x1x + (-1) .* x3x) .^ 2 + (x1y + (-1) .* x3y) .^ 2 + ( ...
  x1z + (-1) .* x3z) .^ 2) .^ (-1 / 2) .* (x1z + (-1) .* x3z) + (( ...
  x2x + (-1) .* x4x) .^ 2 + (x2y + (-1) .* x4y) .^ 2 + (x2z + (-1)  ...
  .* x4z) .^ 2) .^ (-1 / 2) .* (x2z + (-1) .* x4z)) .^ 2) .^ (-1 /  ...
  2) .* ((x1y + (-1) .* x3y) .* ((x1x + (-1) .* x3x) .^ 2 + (x1y + ( ...
  -1) .* x3y) .^ 2 + (x1z + (-1) .* x3z) .^ 2) .^ (-1 / 2) + (x2y +  ...
  (-1) .* x4y) .* ((x2x + (-1) .* x4x) .^ 2 + (x2y + (-1) .* x4y)  ...
  .^ 2 + (x2z + (-1) .* x4z) .^ 2) .^ (-1 / 2)) + (1 / 2) .* (((-1)  ...
  .* x1y + x3y) .* (x2x + (-1) .* x4x) + (x1x + (-1) .* x3x) .* ( ...
  x2y + (-1) .* x4y)) .* ((((-1) .* x1y + x3y) .* (x2x + (-1) .*  ...
  x4x) + (x1x + (-1) .* x3x) .* (x2y + (-1) .* x4y)) .^ 2 + ((x1z +  ...
  (-1) .* x3z) .* (x2x + (-1) .* x4x) + (-1) .* (x1x + (-1) .* x3x)  ...
  .* (x2z + (-1) .* x4z)) .^ 2 + (((-1) .* x1z + x3z) .* (x2y + (-1) ...
   .* x4y) + (x1y + (-1) .* x3y) .* (x2z + (-1) .* x4z)) .^ 2) .^ ( ...
  -1 / 2) .* (((x1x + (-1) .* x3x) .* ((x1x + (-1) .* x3x) .^ 2 + ( ...
  x1y + (-1) .* x3y) .^ 2 + (x1z + (-1) .* x3z) .^ 2) .^ (-1 / 2) +  ...
  (x2x + (-1) .* x4x) .* ((x2x + (-1) .* x4x) .^ 2 + (x2y + (-1) .*  ...
  x4y) .^ 2 + (x2z + (-1) .* x4z) .^ 2) .^ (-1 / 2)) .^ 2 + ((x1y +  ...
  (-1) .* x3y) .* ((x1x + (-1) .* x3x) .^ 2 + (x1y + (-1) .* x3y)  ...
  .^ 2 + (x1z + (-1) .* x3z) .^ 2) .^ (-1 / 2) + (x2y + (-1) .* x4y) ...
   .* ((x2x + (-1) .* x4x) .^ 2 + (x2y + (-1) .* x4y) .^ 2 + (x2z +  ...
  (-1) .* x4z) .^ 2) .^ (-1 / 2)) .^ 2 + (((x1x + (-1) .* x3x) .^ 2  ...
  + (x1y + (-1) .* x3y) .^ 2 + (x1z + (-1) .* x3z) .^ 2) .^ (-1 / 2) ...
   .* (x1z + (-1) .* x3z) + ((x2x + (-1) .* x4x) .^ 2 + (x2y + (-1)  ...
  .* x4y) .^ 2 + (x2z + (-1) .* x4z) .^ 2) .^ (-1 / 2) .* (x2z + ( ...
  -1) .* x4z)) .^ 2) .^ (-3 / 2) .* ((x1y + (-1) .* x3y) .* ((x1x +  ...
  (-1) .* x3x) .^ 2 + (x1y + (-1) .* x3y) .^ 2 + (x1z + (-1) .* x3z) ...
   .^ 2) .^ (-1 / 2) + (x2y + (-1) .* x4y) .* ((x2x + (-1) .* x4x)  ...
  .^ 2 + (x2y + (-1) .* x4y) .^ 2 + (x2z + (-1) .* x4z) .^ 2) .^ ( ...
  -1 / 2)) .* (2 .* ((x2x + (-1) .* x4x) .^ 2 .* ((x2x + (-1) .*  ...
  x4x) .^ 2 + (x2y + (-1) .* x4y) .^ 2 + (x2z + (-1) .* x4z) .^ 2)  ...
  .^ (-3 / 2) + (-1) .* ((x2x + (-1) .* x4x) .^ 2 + (x2y + (-1) .*  ...
  x4y) .^ 2 + (x2z + (-1) .* x4z) .^ 2) .^ (-1 / 2)) .* ((x1x + (-1) ...
   .* x3x) .* ((x1x + (-1) .* x3x) .^ 2 + (x1y + (-1) .* x3y) .^ 2 + ...
   (x1z + (-1) .* x3z) .^ 2) .^ (-1 / 2) + (x2x + (-1) .* x4x) .* (( ...
  x2x + (-1) .* x4x) .^ 2 + (x2y + (-1) .* x4y) .^ 2 + (x2z + (-1)  ...
  .* x4z) .^ 2) .^ (-1 / 2)) + 2 .* (x2x + (-1) .* x4x) .* (x2y + ( ...
  -1) .* x4y) .* ((x1y + (-1) .* x3y) .* ((x1x + (-1) .* x3x) .^ 2 + ...
   (x1y + (-1) .* x3y) .^ 2 + (x1z + (-1) .* x3z) .^ 2) .^ (-1 / 2)  ...
  + (x2y + (-1) .* x4y) .* ((x2x + (-1) .* x4x) .^ 2 + (x2y + (-1)  ...
  .* x4y) .^ 2 + (x2z + (-1) .* x4z) .^ 2) .^ (-1 / 2)) .* ((x2x + ( ...
  -1) .* x4x) .^ 2 + (x2y + (-1) .* x4y) .^ 2 + (x2z + (-1) .* x4z)  ...
  .^ 2) .^ (-3 / 2) + 2 .* (x2x + (-1) .* x4x) .* (((x1x + (-1) .*  ...
  x3x) .^ 2 + (x1y + (-1) .* x3y) .^ 2 + (x1z + (-1) .* x3z) .^ 2)  ...
  .^ (-1 / 2) .* (x1z + (-1) .* x3z) + ((x2x + (-1) .* x4x) .^ 2 + ( ...
  x2y + (-1) .* x4y) .^ 2 + (x2z + (-1) .* x4z) .^ 2) .^ (-1 / 2) .* ...
   (x2z + (-1) .* x4z)) .* ((x2x + (-1) .* x4x) .^ 2 + (x2y + (-1)  ...
  .* x4y) .^ 2 + (x2z + (-1) .* x4z) .^ 2) .^ (-3 / 2) .* (x2z + ( ...
  -1) .* x4z)) + ((-1) .* x1z + x3z) .* ((((-1) .* x1y + x3y) .* ( ...
  x2x + (-1) .* x4x) + (x1x + (-1) .* x3x) .* (x2y + (-1) .* x4y))  ...
  .^ 2 + ((x1z + (-1) .* x3z) .* (x2x + (-1) .* x4x) + (-1) .* (x1x  ...
  + (-1) .* x3x) .* (x2z + (-1) .* x4z)) .^ 2 + (((-1) .* x1z + x3z) ...
   .* (x2y + (-1) .* x4y) + (x1y + (-1) .* x3y) .* (x2z + (-1) .*  ...
  x4z)) .^ 2) .^ (-1 / 2) .* (((x1x + (-1) .* x3x) .* ((x1x + (-1)  ...
  .* x3x) .^ 2 + (x1y + (-1) .* x3y) .^ 2 + (x1z + (-1) .* x3z) .^  ...
  2) .^ (-1 / 2) + (x2x + (-1) .* x4x) .* ((x2x + (-1) .* x4x) .^ 2  ...
  + (x2y + (-1) .* x4y) .^ 2 + (x2z + (-1) .* x4z) .^ 2) .^ (-1 / 2) ...
  ) .^ 2 + ((x1y + (-1) .* x3y) .* ((x1x + (-1) .* x3x) .^ 2 + (x1y  ...
  + (-1) .* x3y) .^ 2 + (x1z + (-1) .* x3z) .^ 2) .^ (-1 / 2) + ( ...
  x2y + (-1) .* x4y) .* ((x2x + (-1) .* x4x) .^ 2 + (x2y + (-1) .*  ...
  x4y) .^ 2 + (x2z + (-1) .* x4z) .^ 2) .^ (-1 / 2)) .^ 2 + (((x1x + ...
   (-1) .* x3x) .^ 2 + (x1y + (-1) .* x3y) .^ 2 + (x1z + (-1) .*  ...
  x3z) .^ 2) .^ (-1 / 2) .* (x1z + (-1) .* x3z) + ((x2x + (-1) .*  ...
  x4x) .^ 2 + (x2y + (-1) .* x4y) .^ 2 + (x2z + (-1) .* x4z) .^ 2)  ...
  .^ (-1 / 2) .* (x2z + (-1) .* x4z)) .^ 2) .^ (-1 / 2) .* (((x1x +  ...
  (-1) .* x3x) .^ 2 + (x1y + (-1) .* x3y) .^ 2 + (x1z + (-1) .* x3z) ...
   .^ 2) .^ (-1 / 2) .* (x1z + (-1) .* x3z) + ((x2x + (-1) .* x4x)  ...
  .^ 2 + (x2y + (-1) .* x4y) .^ 2 + (x2z + (-1) .* x4z) .^ 2) .^ ( ...
  -1 / 2) .* (x2z + (-1) .* x4z)) + (-1 / 2) .* (2 .* (x1y + (-1) .* ...
   x3y) .* (((-1) .* x1y + x3y) .* (x2x + (-1) .* x4x) + (x1x + (-1) ...
   .* x3x) .* (x2y + (-1) .* x4y)) + 2 .* ((-1) .* x1z + x3z) .* (( ...
  x1z + (-1) .* x3z) .* (x2x + (-1) .* x4x) + (-1) .* (x1x + (-1) .* ...
   x3x) .* (x2z + (-1) .* x4z))) .* ((((-1) .* x1y + x3y) .* (x2x +  ...
  (-1) .* x4x) + (x1x + (-1) .* x3x) .* (x2y + (-1) .* x4y)) .^ 2 +  ...
  ((x1z + (-1) .* x3z) .* (x2x + (-1) .* x4x) + (-1) .* (x1x + (-1)  ...
  .* x3x) .* (x2z + (-1) .* x4z)) .^ 2 + (((-1) .* x1z + x3z) .* ( ...
  x2y + (-1) .* x4y) + (x1y + (-1) .* x3y) .* (x2z + (-1) .* x4z))  ...
  .^ 2) .^ (-3 / 2) .* (((x1x + (-1) .* x3x) .* ((x1x + (-1) .* x3x) ...
   .^ 2 + (x1y + (-1) .* x3y) .^ 2 + (x1z + (-1) .* x3z) .^ 2) .^ ( ...
